simulink model "FeedBack_Linearization"  (R2021b)
settings: Solver=VariableStepAuto  StartTime=0.0  StopTime=10.0  RelTol=1e-3
undefined symbols (not defined in the file): Kd, Kp, q_dq_init
(part 2 of 9)

== matlab function FeedBack_Linearization/M ==
  data: q input; M output
function M = M_fun(q)
%M_fun
%    M = M_fun(Q1,Q2,Q3,Q4,Q5,Q6,Q7)

%    This function was generated by the Symbolic Math Toolbox version 9.0.
%    15-Apr-2022 02:51:43

q1 = q(1);
q2 = q(2);
q3 = q(3);
q4 = q(4);
q5 = q(5);
q6 = q(6);
q7 = q(7);

t2 = cos(q1);
t3 = cos(q2);
t4 = cos(q3);
t5 = cos(q4);
t6 = cos(q5);
t7 = cos(q6);
t8 = cos(q7);
t9 = sin(q1);
t10 = sin(q2);
t11 = sin(q3);
t12 = sin(q4);
t13 = sin(q5);
t14 = sin(q6);
t15 = sin(q7);
t16 = t2.^2;
t17 = t3.^2;
t18 = t9.^2;
t19 = t10.^2;
t20 = t11.^2;
t21 = t2.*t4;
t22 = t3.*t5;
t23 = t2.*t11;
t24 = t4.*t9;
t25 = t3.*t12;
t26 = t5.*t10;
t27 = t9.*t11;
t28 = t10.*t12;
t30 = t10.*t11.*t13;
t44 = t3.*t4.*t10;
t48 = t3.*t6.*t11;
t49 = t4.*t6.*t10;
t55 = t3.*t11.*t13;
t56 = t4.*t10.*t13;
t57 = t6.*t10.*t11;
t60 = t10.*(2.1e+1./5.0e+1);
t86 = t2.*t3.*(2.1e+1./5.0e+1);
t90 = t3.*t9.*(2.1e+1./5.0e+1);
t329 = t2.*3.55e-3;
t332 = t9.*3.55e-3;
t359 = t10.*t11.*2.25e-3;
t360 = t2.*t3.*1.6669e-1;
t361 = t2.*t10.*1.6669e-1;
t362 = t3.*t9.*1.6669e-1;
t364 = t9.*t10.*1.6669e-1;
t372 = t3.*t4.*2.25e-3;
t383 = t3.*t11.*3.492e-2;
t384 = t4.*t10.*3.492e-2;
t388 = t2.*t10.*7.669999999999999e-3;
t389 = t3.*t9.*7.669999999999999e-3;
t390 = t9.*t10.*7.669999999999999e-3;
t405 = t3.*t11.*3.818e-2;
t406 = t4.*t10.*3.818e-2;
t415 = t2.*t3.*7.669999999999999e-3;
t416 = t10.*3.9348e-1;
t471 = t2.*t3.*3.9348e-1;
t473 = t3.*t9.*3.9348e-1;
t493 = t9.*t10.*(-3.9348e-1);
t29 = t9.*t28;
t31 = t3.*t16;
t32 = t3.*t18;
t33 = t10.*t16;
t34 = t4.*t19;
t35 = t11.*t17;
t36 = t10.*t18;
t37 = t3.*t21;
t38 = t2.*t22;
t39 = t4.*t22;
t40 = t3.*t23;
t41 = t3.*t24;
t42 = t2.*t25;
t43 = t2.*t26;
t45 = t9.*t22;
t46 = t4.*t25;
t47 = t4.*t26;
t50 = t3.*t27;
t51 = t2.*t28;
t52 = t9.*t25;
t53 = t9.*t26;
t54 = t4.*t28;
t58 = t25.*(2.0./5.0);
t59 = t26.*(2.0./5.0);
t62 = t21.*t26;
t63 = t21.*t28;
t64 = t11.*t44;
t65 = t24.*t26;
t66 = t6.*t10.*t23;
t67 = t6.*t11.*t26;
t68 = t16.*t19;
t70 = t24.*t28;
t71 = t10.*t13.*t23;
t72 = t6.*t10.*t27;
t73 = t11.*t13.*t26;
t74 = t7.*t11.*t28;
t75 = t18.*t19;
t76 = t19.*t20;
t79 = t10.*t13.*t27;
t80 = t11.*t14.*t28;
t84 = -t55;
t85 = -t57;
t88 = t11.*t28.*(2.0./5.0);
t89 = t2.*t60;
t91 = t9.*t60;
t99 = -t86;
t101 = -t90;
t330 = t25.*1.8866e-1;
t331 = t26.*1.8866e-1;
t335 = -t332;
t355 = t11.*t28.*1.8866e-1;
t356 = t23.*2.25e-3;
t357 = t24.*2.25e-3;
t358 = t27.*2.25e-3;
t371 = t21.*2.25e-3;
t373 = t25.*5.267999999999999e-2;
t374 = t26.*5.267999999999999e-2;
t377 = t48.*2.37e-3;
t378 = t49.*2.37e-3;
t379 = t21.*3.492e-2;
t380 = t30.*2.37e-3;
t381 = t23.*3.492e-2;
t382 = t24.*3.492e-2;
t385 = t27.*3.492e-2;
t387 = -t372;
t391 = t48.*2.75e-2;
t392 = t49.*2.75e-2;
t393 = t30.*2.75e-2;
t402 = t21.*3.818e-2;
t403 = t23.*3.818e-2;
t404 = t24.*3.818e-2;
t408 = t27.*3.818e-2;
t418 = -t388;
t423 = -t390;
t428 = t11.*t28.*5.267999999999999e-2;
t435 = t22.*2.0e-4;
t440 = t28.*2.0e-4;
t441 = -t406;
t447 = t55.*5.000000000000001e-5;
t448 = t56.*5.000000000000001e-5;
t449 = t57.*5.000000000000001e-5;
t466 = t10.*t23.*(-3.492e-2);
t469 = t10.*t27.*(-3.492e-2);
t472 = t2.*t416;
t474 = t9.*t416;
t491 = t11.*t26.*2.0e-4;
t615 = t17.*1.16152294893368e-19;
t629 = t17.*8.909980864224564e-21;
t807 = t44.*7.000000000000001e-5;
t830 = t44.*4.999999999999997e-5;
t845 = t44.*2.23e-3;
t944 = t359+t384;
t1327 = t329+t364+t389;
t61 = -t58;
t69 = -t37;
t77 = -t46;
t78 = -t47;
t81 = -t50;
t82 = -t51;
t83 = -t53;
t87 = t29.*(2.0./5.0);
t92 = t38.*(2.0./5.0);
t93 = t43.*(2.0./5.0);
t94 = t45.*(2.0./5.0);
t95 = t46.*(2.0./5.0);
t96 = t47.*(2.0./5.0);
t97 = t51.*(2.0./5.0);
t98 = t53.*(2.0./5.0);
t100 = -t88;
t102 = t11.*t68;
t103 = -t62;
t104 = t11.*t75;
t105 = t12.*t76;
t106 = -t65;
t107 = -t66;
t108 = -t72;
t109 = -t73;
t110 = -t74;
t113 = t63.*(2.0./5.0);
t114 = t70.*(2.0./5.0);
t115 = t23+t41;
t116 = t24+t40;
t117 = t22+t54;
t118 = t28+t39;
t119 = t31+t32;
t120 = t33+t36;
t137 = t38+t63;
t138 = t45+t70;
t139 = t56+t67;
t223 = t17+t68+t75;
t334 = -t330;
t347 = t38.*1.8866e-1;
t348 = t43.*1.8866e-1;
t349 = t45.*1.8866e-1;
t350 = t46.*1.8866e-1;
t351 = t47.*1.8866e-1;
t352 = t51.*1.8866e-1;
t353 = t53.*1.8866e-1;
t354 = t29.*1.8866e-1;
t366 = -t355;
t375 = t63.*1.8866e-1;
t376 = t70.*1.8866e-1;
t386 = -t371;
t394 = -t374;
t400 = -t378;
t407 = t37.*2.25e-3;
t409 = -t385;
t410 = t40.*2.25e-3;
t411 = t10.*t371;
t412 = t41.*2.25e-3;
t413 = t50.*2.25e-3;
t414 = t10.*t357;
t417 = t38.*5.267999999999999e-2;
t419 = t43.*5.267999999999999e-2;
t420 = t45.*5.267999999999999e-2;
t421 = t46.*5.267999999999999e-2;
t422 = t47.*5.267999999999999e-2;
t424 = -t392;
t425 = t51.*5.267999999999999e-2;
t426 = t53.*5.267999999999999e-2;
t427 = t29.*5.267999999999999e-2;
t429 = t66.*2.37e-3;
t430 = t37.*3.492e-2;
t431 = t72.*2.37e-3;
t432 = t73.*2.37e-3;
t433 = t40.*3.492e-2;
t434 = t41.*3.492e-2;
t436 = t10.*t381;
t437 = t50.*3.492e-2;
t438 = -t402;
t439 = t10.*t385;
t443 = t72.*2.75e-2;
t444 = t73.*2.75e-2;
t458 = t37.*3.818e-2;
t460 = t40.*3.818e-2;
t461 = t41.*3.818e-2;
t464 = t10.*t403;
t465 = t50.*3.818e-2;
t468 = t10.*t408;
t475 = t66.*2.75e-2;
t476 = t70.*5.267999999999999e-2;
t478 = -t447;
t479 = t39.*2.0e-4;
t482 = t42.*2.0e-4;
t483 = t43.*2.0e-4;
t487 = t51.*2.0e-4;
t488 = t52.*2.0e-4;
t489 = t53.*2.0e-4;
t490 = t54.*2.0e-4;
t492 = t29.*2.0e-4;
t494 = t80.*4.9e-4;
t495 = t63.*5.267999999999999e-2;
t497 = t79.*5.000000000000001e-5;
t502 = t74.*2.019e-2;
t505 = t67.*5.000000000000001e-5;
t506 = t71.*5.000000000000001e-5;
t507 = t62.*2.0e-4;
t509 = t65.*2.0e-4;
t559 = t74.*1.9738e-1;
t647 = t31.*1.16152294893368e-19;
t652 = t32.*1.16152294893368e-19;
t662 = t33.*8.909980864224564e-21;
t663 = t36.*8.909980864224564e-21;
t666 = t68.*1.16152294893368e-19;
t667 = t75.*1.16152294893368e-19;
t681 = t68.*8.909980864224564e-21;
t684 = t75.*8.909980864224564e-21;
t805 = t34.*7.000000000000022e-5;
t811 = t35.*7.000000000000001e-5;
t829 = t64.*7.000000000000001e-5;
t831 = t76.*7.000000000000001e-5;
t832 = t64.*7.000000000000022e-5;
t833 = t76.*7.000000000000022e-5;
t834 = t34.*4.999999999999997e-5;
t835 = t35.*4.999999999999997e-5;
t839 = -t830;
t840 = t35.*2.23e-3;
t853 = t34.*2.19e-3;
t886 = t64.*7.299999999999999e-4;
t887 = t76.*7.299999999999999e-4;
t979 = t360+t418;
t980 = t362+t423;
t1340 = t335+t361+t415;
t1366 = t383+t387+t416;
t1410 = t428+t441+t491;
t111 = -t95;
t112 = -t97;
t121 = t21+t81;
t122 = t27+t69;
t123 = t25+t78;
t124 = t26+t77;
t125 = t116.^2;
t126 = t117.^2;
t127 = t5.*t115;
t128 = t6.*t115;
t129 = t6.*t116;
t130 = t6.*t118;
t131 = t7.*t117;
t132 = t12.*t115;
t133 = t13.*t115;
t134 = t13.*t116;
t135 = t13.*t118;
t136 = t14.*t117;
t145 = t2.*t10.*t115;
t146 = t3.*t9.*t115;
t148 = t7.*t12.*t116;
t150 = t8.*t13.*t117;
t151 = t9.*t10.*t115;
t152 = t9.*t10.*t116;
t153 = t12.*t14.*t116;
t154 = t13.*t15.*t117;
t169 = t42+t103;
t170 = t52+t106;
t171 = t49+t109;
t174 = t12.*t116.*(2.0./5.0);
t176 = t7.*t137;
t177 = t10.*t21.*t116;
t178 = t14.*t137;
t179 = t7.*t138;
t180 = t11.*t26.*t117;
t181 = t7.*t139;
t185 = t14.*t138;
t186 = t14.*t139;
t230 = t115.*t116;
t231 = t117.*t118;
t252 = t35+t102+t104;
t272 = t116.*t137;
t363 = -t350;
t365 = -t352;
t442 = -t407;
t445 = -t419;
t446 = -t422;
t450 = -t426;
t457 = -t429;
t459 = -t431;
t467 = -t437;
t477 = -t443;
t484 = -t458;
t496 = -t475;
t501 = -t482;
t503 = -t488;
t522 = t12.*t116.*1.8866e-1;
t542 = t13.*t117.*2.37e-3;
t556 = t13.*t117.*2.75e-2;
t571 = t12.*t116.*5.267999999999999e-2;
t578 = t6.*t117.*5.000000000000001e-5;
t588 = t5.*t116.*2.0e-4;
t837 = -t829;
t846 = -t834;
t847 = t102.*7.000000000000001e-5;
t849 = t104.*7.000000000000001e-5;
t859 = t102.*4.999999999999997e-5;
t860 = t104.*4.999999999999997e-5;
t867 = -t853;
t884 = t102.*2.23e-3;
t885 = t104.*2.23e-3;
t895 = -t886;
t907 = t105.*3.844e-2;
t915 = t105.*1.12e-3;
t916 = t105.*8.8e-4;
t1403 = t411+t466+t471;
t1404 = t414+t469+t473;
t1568 = t357+t409+t410+t430;
t1569 = t381+t386+t413+t434;
t1576 = t615+t666+t667;
t1594 = t629+t681+t684;
t1781 = t979.*t1327.*4.50275;
t1782 = t366+t400+t432+t448+t505;
t1785 = t980.*t1340.*4.50275;
t1789 = t944.*t1366.*2.4552;
t1797 = t60+t394+t405+t421+t440+t479;
t1801 = t647+t652+t662+t663;
t140 = t121.^2;
t141 = t12.*t125;
t142 = t13.*t126;
t143 = t5.*t129;
t144 = t6.*t131;
t147 = t5.*t134;
t149 = t6.*t136;
t155 = t5.*t122;
t156 = t6.*t121;
t157 = t6.*t122;
t158 = -t129;
t159 = t6.*t123;
t160 = t7.*t123;
t161 = t7.*t124;
t162 = t12.*t122;
t163 = t13.*t121;
t164 = t13.*t122;
t165 = t13.*t123;
t166 = t14.*t123;
t167 = t14.*t124;
t168 = -t136;
t172 = t127.*(2.0./5.0);
t173 = t132.*(2.0./5.0);
t182 = t2.*t3.*t122;
t187 = t2.*t10.*t121;
t188 = t2.*t10.*t122;
t190 = t3.*t11.*t123;
t191 = t4.*t10.*t123;
t192 = t7.*t12.*t121;
t194 = t9.*t10.*t122;
t195 = -t151;
t196 = t10.*t11.*t123;
t197 = t10.*t11.*t124;
t198 = t12.*t14.*t121;
t199 = -t153;
t200 = -t154;
t203 = -t174;
t206 = t12.*t121.*(2.0./5.0);
t208 = t6.*t169;
t209 = -t177;
t210 = t13.*t169;
t211 = t10.*t24.*t121;
t212 = t6.*t170;
t213 = -t180;
t214 = t8.*t171;
t217 = t13.*t170;
t218 = t15.*t171;
t224 = t29+t127;
t225 = t48+t135;
t226 = t83+t132;
t229 = t84+t130;
t240 = (t53-t132).^2;
t243 = -t7.*(t55-t130);
t244 = -t7.*(t53-t132);
t247 = -t14.*(t55-t130);
t249 = -t14.*(t53-t132);
t254 = t80+t181;
t260 = -t8.*t13.*(t53-t132);
t262 = t121.*t122;
t265 = -t13.*t15.*(t53-t132);
t276 = t110+t186;
t277 = t6.*t7.*(t53-t132);
t281 = t8.*t13.*(t53-t132);
t286 = t121.*t138;
t287 = t117.*t171;
t326 = -t116.*(t53-t132);
t342 = t116.*(t53-t132);
t367 = -t5.*t121.*(t53-t132);
t398 = -t170.*(t53-t132);
t520 = t127.*1.8866e-1;
t521 = t132.*1.8866e-1;
t525 = -t522;
t537 = t12.*t121.*1.8866e-1;
t539 = t128.*2.37e-3;
t540 = t129.*2.37e-3;
t541 = t134.*2.37e-3;
t543 = t135.*2.37e-3;
t553 = t128.*2.75e-2;
t554 = t129.*2.75e-2;
t555 = t134.*2.75e-2;
t557 = t135.*2.75e-2;
t566 = t131.*4.9e-4;
t569 = t127.*5.267999999999999e-2;
t570 = t132.*5.267999999999999e-2;
t574 = t136.*2.019e-2;
t577 = t129.*5.000000000000001e-5;
t579 = t130.*5.000000000000001e-5;
t583 = t133.*5.000000000000001e-5;
t584 = t134.*5.000000000000001e-5;
t587 = t127.*2.0e-4;
t589 = t132.*2.0e-4;
t593 = t153.*4.9e-4;
t602 = t12.*t121.*5.267999999999999e-2;
t604 = t148.*2.019e-2;
t623 = t5.*t121.*2.0e-4;
t627 = t154.*3.466000000000001e-2;
t628 = t178.*4.9e-4;
t630 = t181.*4.9e-4;
t631 = t185.*4.9e-4;
t636 = t179.*2.019e-2;
t637 = t150.*2.324e-2;
t640 = t186.*2.019e-2;
t657 = t176.*2.019e-2;
t664 = t136.*1.9738e-1;
t679 = t148.*1.9738e-1;
t700 = t176.*1.9738e-1;
t702 = t179.*1.9738e-1;
t704 = t186.*1.9738e-1;
t714 = t13.*(t53-t132).*(-2.37e-3);
t719 = t13.*(t53-t132).*(-2.75e-2);
t729 = t7.*(t55-t130).*(-4.9e-4);
t730 = t7.*(t53-t132).*(-4.9e-4);
t732 = t14.*(t53-t132).*(-4.9e-4);
t741 = t7.*(t53-t132).*4.9e-4;
t745 = t6.*(t53-t132).*(-5.000000000000001e-5);
t751 = t7.*(t53-t132).*(-2.019e-2);
t754 = t14.*(t55-t130).*(-2.019e-2);
t756 = t14.*(t53-t132).*(-2.019e-2);
t764 = t14.*(t55-t130).*2.019e-2;
t782 = t6.*t14.*(t53-t132).*2.019e-2;
t784 = t13.*t15.*(t53-t132).*(-3.466000000000001e-2);
t790 = t7.*(t53-t132).*(-1.9738e-1);
t793 = t14.*(t55-t130).*(-1.9738e-1);
t794 = t14.*(t53-t132).*(-1.9738e-1);
t804 = t7.*(t53-t132).*1.9738e-1;
t900 = t125.*7.000000000000001e-5;
t904 = t125.*7.000000000000022e-5;
t908 = t151.*7.000000000000001e-5;
t909 = t152.*7.000000000000001e-5;
t910 = t145.*7.000000000000022e-5;
t911 = t146.*7.000000000000022e-5;
M = ft_1({q1,q2,t10,t100,t101,t105,t107,t108,t11,t111,t112,t113,t114,t115,t116,t117,t119,t12,t120,t121,t122,t123,t124,t125,t126,t128,t129,t13,t130,t131,t132,t1327,t133,t134,t1340,t136,t1366,t137,t138,t139,t14,t140,t1403,t1404,t141,t1410,t142,t143,t144,t145,t146,t147,t148,t149,t15,t150,t151,t152,t153,t154,t155,t156,t1568,t1569,t157,t1576,t158,t159,t1594,t16,t160,t161,t162,t163,t164,t165,t166,t167,t168,t169,t17,t170,t171,t172,t173,t174,t176,t177,t178,t1781,t1782,t1785,t1789,t179,t1797,t18,t180,t1801,t182,t185,t186,t187,t188,t190,t191,t192,t194,t195,t196,t197,t198,t199,t200,t203,t206,t208,t209,t210,t211,t212,t213,t214,t217,t218,t223,t224,t225,t23,t230,t231,t240,t243,t244,t247,t249,t252,t254,t262,t265,t27,t272,t277,t28,t281,t286,t287,t30,t31,t32,t33,t331,t334,t34,t342,t347,t348,t349,t351,t353,t354,t356,t358,t36,t363,t365,t367,t373,t375,t376,t377,t379,t380,t382,t391,t393,t398,t403,t404,t408,t412,t417,t420,t424,t425,t427,t43,t433,t435,t438,t44,t442,t444,t445,t446,t449,t450,t457,t459,t460,t461,t464,t465,t467,t468,t472,t476,t477,t478,t483,t484,t487,t489,t490,t492,t493,t494,t495,t496,t497,t5,t501,t502,t503,t506,t507,t509,t51,t520,t521,t525,t53,t537,t539,t540,t541,t542,t543,t55,t553,t554,t555,t556,t557,t559,t566,t569,t57,t570,t571,t574,t577,t578,t579,t583,t584,t587,t588,t589,t59,t593,t6,t60,t602,t604,t61,t623,t627,t628,t630,t631,t636,t637,t64,t640,t657,t66,t664,t679,t68,t7,t700,t702,t704,t71,t714,t719,t72,t729,t732,t74,t741,t745,t75,t751,t756,t76,t764,t782,t784,t79,t793,t794,t8,t804,t805,t807,t811,t82,t831,t832,t833,t835,t837,t839,t840,t845,t846,t847,t849,t85,t859,t86,t860,t867,t87,t88,t884,t885,t887,t89,t895,t9,t90,t900,t904,t907,t908,t909,t91,t910,t911,t915,t916,t92,t93,t94,t944,t96,t97,t979,t98,t980,t99});
end
function M = ft_1(ct)
q1 = ct{1};
q2 = ct{2};
t10 = ct{3};
t100 = ct{4};
t101 = ct{5};
t105 = ct{6};
t107 = ct{7};
t108 = ct{8};
t11 = ct{9};
t111 = ct{10};
t112 = ct{11};
t113 = ct{12};
t114 = ct{13};
t115 = ct{14};
t116 = ct{15};
t117 = ct{16};
t119 = ct{17};
t12 = ct{18};
t120 = ct{19};
t121 = ct{20};
t122 = ct{21};
t123 = ct{22};
t124 = ct{23};
t125 = ct{24};
t126 = ct{25};
t128 = ct{26};
t129 = ct{27};
t13 = ct{28};
t130 = ct{29};
t131 = ct{30};
t132 = ct{31};
t1327 = ct{32};
t133 = ct{33};
t134 = ct{34};
t1340 = ct{35};
t136 = ct{36};
t1366 = ct{37};
t137 = ct{38};
t138 = ct{39};
t139 = ct{40};
t14 = ct{41};
t140 = ct{42};
t1403 = ct{43};
t1404 = ct{44};
t141 = ct{45};
t1410 = ct{46};
t142 = ct{47};
t143 = ct{48};
t144 = ct{49};
t145 = ct{50};
t146 = ct{51};
t147 = ct{52};
t148 = ct{53};
t149 = ct{54};
t15 = ct{55};
t150 = ct{56};
t151 = ct{57};
t152 = ct{58};
t153 = ct{59};
t154 = ct{60};
t155 = ct{61};
t156 = ct{62};
t1568 = ct{63};
t1569 = ct{64};
t157 = ct{65};
t1576 = ct{66};
t158 = ct{67};
t159 = ct{68};
t1594 = ct{69};
t16 = ct{70};
t160 = ct{71};
t161 = ct{72};
t162 = ct{73};
t163 = ct{74};
t164 = ct{75};
t165 = ct{76};
t166 = ct{77};
t167 = ct{78};
t168 = ct{79};
t169 = ct{80};
t17 = ct{81};
t170 = ct{82};
t171 = ct{83};
t172 = ct{84};
t173 = ct{85};
t174 = ct{86};
t176 = ct{87};
t177 = ct{88};
t178 = ct{89};
t1781 = ct{90};
t1782 = ct{91};
t1785 = ct{92};
t1789 = ct{93};
t179 = ct{94};
t1797 = ct{95};
t18 = ct{96};
t180 = ct{97};
t1801 = ct{98};
t182 = ct{99};
t185 = ct{100};
t186 = ct{101};
t187 = ct{102};
t188 = ct{103};
t190 = ct{104};
t191 = ct{105};
t192 = ct{106};
t194 = ct{107};
t195 = ct{108};
t196 = ct{109};
t197 = ct{110};
t198 = ct{111};
t199 = ct{112};
t200 = ct{113};
t203 = ct{114};
t206 = ct{115};
t208 = ct{116};
t209 = ct{117};
t210 = ct{118};
t211 = ct{119};
t212 = ct{120};
t213 = ct{121};
t214 = ct{122};
t217 = ct{123};
t218 = ct{124};
t223 = ct{125};
t224 = ct{126};
t225 = ct{127};
t23 = ct{128};
t230 = ct{129};
t231 = ct{130};
t240 = ct{131};
t243 = ct{132};
t244 = ct{133};
t247 = ct{134};
t249 = ct{135};
t252 = ct{136};
t254 = ct{137};
t262 = ct{138};
t265 = ct{139};
t27 = ct{140};
t272 = ct{141};
t277 = ct{142};
t28 = ct{143};
t281 = ct{144};
t286 = ct{145};
t287 = ct{146};
t30 = ct{147};
t31 = ct{148};
t32 = ct{149};
t33 = ct{150};
t331 = ct{151};
t334 = ct{152};
t34 = ct{153};
t342 = ct{154};
t347 = ct{155};
t348 = ct{156};
t349 = ct{157};
t351 = ct{158};
t353 = ct{159};
t354 = ct{160};
t356 = ct{161};
t358 = ct{162};
t36 = ct{163};
t363 = ct{164};
t365 = ct{165};
t367 = ct{166};
t373 = ct{167};
t375 = ct{168};
t376 = ct{169};
t377 = ct{170};
t379 = ct{171};
t380 = ct{172};
t382 = ct{173};
t391 = ct{174};
t393 = ct{175};
t398 = ct{176};
t403 = ct{177};
t404 = ct{178};
t408 = ct{179};
t412 = ct{180};
t417 = ct{181};
t420 = ct{182};
t424 = ct{183};
t425 = ct{184};
t427 = ct{185};
t43 = ct{186};
t433 = ct{187};
t435 = ct{188};
t438 = ct{189};
t44 = ct{190};
t442 = ct{191};
t444 = ct{192};
t445 = ct{193};
t446 = ct{194};
t449 = ct{195};
t450 = ct{196};
t457 = ct{197};
t459 = ct{198};
t460 = ct{199};
t461 = ct{200};
t464 = ct{201};
t465 = ct{202};
t467 = ct{203};
t468 = ct{204};
t472 = ct{205};
t476 = ct{206};
t477 = ct{207};
t478 = ct{208};
t483 = ct{209};
t484 = ct{210};
t487 = ct{211};
t489 = ct{212};
t490 = ct{213};
t492 = ct{214};
t493 = ct{215};
t494 = ct{216};
t495 = ct{217};
t496 = ct{218};
t497 = ct{219};
t5 = ct{220};
t501 = ct{221};
t502 = ct{222};
t503 = ct{223};
t506 = ct{224};
t507 = ct{225};
t509 = ct{226};
t51 = ct{227};
t520 = ct{228};
t521 = ct{229};
t525 = ct{230};
t53 = ct{231};
t537 = ct{232};
t539 = ct{233};
t540 = ct{234};
t541 = ct{235};
t542 = ct{236};
t543 = ct{237};
t55 = ct{238};
t553 = ct{239};
t554 = ct{240};
t555 = ct{241};
t556 = ct{242};
t557 = ct{243};
t559 = ct{244};
t566 = ct{245};
t569 = ct{246};
t57 = ct{247};
t570 = ct{248};
t571 = ct{249};
t574 = ct{250};
t577 = ct{251};
t578 = ct{252};
t579 = ct{253};
t583 = ct{254};
t584 = ct{255};
t587 = ct{256};
t588 = ct{257};
t589 = ct{258};
t59 = ct{259};
t593 = ct{260};
t6 = ct{261};
t60 = ct{262};
t602 = ct{263};
t604 = ct{264};
t61 = ct{265};
t623 = ct{266};
t627 = ct{267};
t628 = ct{268};
t630 = ct{269};
t631 = ct{270};
t636 = ct{271};
t637 = ct{272};
t64 = ct{273};
t640 = ct{274};
t657 = ct{275};
t66 = ct{276};
t664 = ct{277};
t679 = ct{278};
t68 = ct{279};
t7 = ct{280};
t700 = ct{281};
t702 = ct{282};
t704 = ct{283};
t71 = ct{284};
t714 = ct{285};
t719 = ct{286};
t72 = ct{287};
t729 = ct{288};
t732 = ct{289};
t74 = ct{290};
t741 = ct{291};
t745 = ct{292};
t75 = ct{293};
t751 = ct{294};
t756 = ct{295};
t76 = ct{296};
t764 = ct{297};
t782 = ct{298};
t784 = ct{299};
t79 = ct{300};
t793 = ct{301};
t794 = ct{302};
t8 = ct{303};
t804 = ct{304};
t805 = ct{305};
t807 = ct{306};
t811 = ct{307};
t82 = ct{308};
t831 = ct{309};
t832 = ct{310};
t833 = ct{311};
t835 = ct{312};
t837 = ct{313};
t839 = ct{314};
t840 = ct{315};
t845 = ct{316};
t846 = ct{317};
t847 = ct{318};
t849 = ct{319};
t85 = ct{320};
t859 = ct{321};
t86 = ct{322};
t860 = ct{323};
t867 = ct{324};
t87 = ct{325};
t88 = ct{326};
t884 = ct{327};
t885 = ct{328};
t887 = ct{329};
t89 = ct{330};
t895 = ct{331};
t9 = ct{332};
t90 = ct{333};
t900 = ct{334};
t904 = ct{335};
t907 = ct{336};
t908 = ct{337};
t909 = ct{338};
t91 = ct{339};
t910 = ct{340};
t911 = ct{341};
t915 = ct{342};
t916 = ct{343};
t92 = ct{344};
t93 = ct{345};
t94 = ct{346};
t944 = ct{347};
t96 = ct{348};
t97 = ct{349};
t979 = ct{350};
t98 = ct{351};
t980 = ct{352};
t99 = ct{353};
t921 = t126.*1.11e-3;
t927 = t177.*7.000000000000022e-5;
t932 = t177.*7.000000000000001e-5;
t934 = t145.*4.999999999999997e-5;
t935 = t146.*4.999999999999997e-5;
t936 = t151.*4.999999999999997e-5;
t937 = t152.*4.999999999999997e-5;
t940 = t125.*7.299999999999999e-4;
t946 = t151.*2.23e-3;
t947 = t152.*2.23e-3;
t967 = t126.*1.12e-3;
t974 = t180.*1.11e-3;
t975 = t145.*2.19e-3;
t976 = t146.*2.19e-3;
t1004 = t177.*7.299999999999999e-4;
t1021 = t230.*7.000000000000022e-5;
t1030 = t180.*1.12e-3;
t1036 = t230.*7.000000000000001e-5;
t1063 = t126.*4.988e-2;
t1066 = t231.*1.11e-3;
t1079 = t230.*7.299999999999999e-4;
t1086 = t180.*4.988e-2;
t1094 = t231.*1.12e-3;
t1124 = t272.*3.844e-2;
t1125 = t272.*8.8e-4;
t1136 = t272.*1.12e-3;
t1155 = t231.*4.988e-2;
t1209 = t5.*t121.*(t53-t132).*(-1.11e-3);
t1233 = t170.*(t53-t132).*(-1.11e-3);
t1249 = t5.*t121.*(t53-t132).*(-1.12e-3);
t1259 = t170.*(t53-t132).*(-1.12e-3);
t1285 = t5.*t121.*(t53-t132).*(-4.988e-2);
t1303 = t170.*(t53-t132).*(-4.988e-2);
t1601 = t373+t435+t446+t490;
t1625 = t334+t351+t542+t578;
t1671 = (t119.*t1576)./2.0;
t1687 = (t120.*t1594)./2.0;
t1699 = t408+t484+t571+t588;
t1771 = t358+t382+t433+t442+t472;
t1777 = t356+t379+t412+t467+t493;
t1784 = -t1781;
t1808 = t101+t420+t468+t476+t503+t509;
t1810 = t99+t417+t464+t495+t501+t507;
t1867 = (t223.*t1801)./2.0;
t1969 = t1403.*t1568.*2.4552;
t1970 = t1404.*t1569.*2.4552;
t1995 = t1410.*t1797.*2.61155;
t175 = t12.*t140;
t183 = t5.*t156;
t184 = -t143;
t189 = t5.*t163;
t193 = -t149;
t201 = -t156;
t202 = -t173;
t204 = -t167;
t205 = t155.*(2.0./5.0);
t207 = t162.*(2.0./5.0);
t215 = -t182;
t219 = -t191;
t220 = -t198;
t222 = -t206;
t227 = t30+t159;
t228 = t43+t162;
t232 = t8.*t225;
t233 = t6.*t224;
t234 = t7.*t224;
t235 = t15.*t225;
t236 = t13.*t224;
t237 = t14.*t224;
t238 = t85+t165;
t241 = t82+t155;
t253 = (t57-t165).^2;
t255 = t6.*t244;
t258 = t10.*t27.*t224;
t259 = t6.*t249;
t263 = -t6.*(t51-t155);
t264 = -t7.*(t51-t155);
t266 = -t13.*(t51-t155);
t267 = -t14.*(t51-t155);
t268 = -t8.*(t57-t165);
t269 = -t15.*(t57-t165);
t271 = t13.*t240;
t274 = t71+t208;
t275 = t79+t212;
t283 = -t262;
t285 = t8.*t254;
t288 = t15.*t254;
t290 = t107+t210;
t291 = t108+t217;
t292 = t7.*t15.*(t57-t165);
t296 = -t286;
t297 = -t10.*t23.*(t51-t155);
t301 = t147+t157;
t302 = t144+t166;
t304 = -t8.*(t66-t210);
t305 = -t15.*(t66-t210);
t307 = -t8.*(t72-t217);
t308 = t10.*t23.*(t51-t155);
t309 = -t15.*(t72-t217);
t310 = t117.*t225;
t311 = t115.*t224;
t312 = t116.*t224;
t313 = t145+t194;
t314 = t152+t187;
t318 = t8.*(t66-t210);
t325 = t121.*t224;
t337 = -t7.*(t143-t164);
t338 = -t116.*(t51-t155);
t341 = -t14.*(t143-t164);
t346 = t76+t125+t140;
t368 = -t6.*t117.*(t57-t165);
t369 = -t121.*(t51-t155);
t370 = -t122.*(t51-t155);
t399 = -t139.*(t57-t165);
t401 = t6.*t117.*(t57-t165);
t452 = t161+t247;
t455 = t44+t188+t195;
t462 = t139.*(t57-t165);
t523 = (t129+t13.*(t51-t155)).^2;
t524 = -t521;
t528 = -t8.*(t129+t13.*(t51-t155));
t529 = -t8.*(t167+t7.*(t55-t130));
t531 = -t15.*(t129+t13.*(t51-t155));
t532 = -t15.*(t167+t7.*(t55-t130));
t536 = t155.*1.8866e-1;
t538 = t162.*1.8866e-1;
t544 = t64+t209+t211;
t545 = -t537;
t548 = (t53-t132).*(t51-t155);
t550 = (t55-t130).*(t57-t165);
t551 = t8.*(t167+t7.*(t55-t130));
t552 = t15.*(t129+t13.*(t51-t155));
t560 = t147.*2.37e-3;
t561 = t156.*2.37e-3;
t562 = t157.*2.37e-3;
t563 = t159.*2.37e-3;
t564 = t163.*2.37e-3;
t576 = t147.*2.75e-2;
t580 = t156.*2.75e-2;
t581 = t157.*2.75e-2;
t582 = t159.*2.75e-2;
t585 = t163.*2.75e-2;
t590 = -t574;
t592 = t144.*4.9e-4;
t594 = t166.*4.9e-4;
t595 = t167.*4.9e-4;
t598 = t155.*5.267999999999999e-2;
t600 = -t583;
t601 = -t584;
t603 = t162.*5.267999999999999e-2;
t605 = t149.*2.019e-2;
t606 = -t589;
t607 = t160.*2.019e-2;
t608 = t161.*2.019e-2;
t609 = t143.*5.000000000000001e-5;
t613 = t156.*5.000000000000001e-5;
t617 = t163.*5.000000000000001e-5;
t618 = t164.*5.000000000000001e-5;
t619 = t165.*5.000000000000001e-5;
t621 = t217.*2.37e-3;
t624 = t155.*2.0e-4;
t625 = t162.*2.0e-4;
t632 = t198.*4.9e-4;
t635 = t210.*2.37e-3;
t638 = (t53-t132).*(t72-t217);
t639 = (t57-t165).*(t74-t186);
t641 = t192.*2.019e-2;
t643 = -t628;
t644 = -t631;
t645 = t210.*2.75e-2;
t651 = t217.*2.75e-2;
t660 = -t636;
t661 = -t640;
t665 = -t657;
t669 = t208.*5.000000000000001e-5;
t670 = t212.*5.000000000000001e-5;
t674 = -t664;
t678 = t218.*3.466000000000001e-2;
t680 = t149.*1.9738e-1;
t682 = t160.*1.9738e-1;
t683 = t161.*1.9738e-1;
t699 = t214.*2.324e-2;
t705 = t192.*1.9738e-1;
t707 = -t8.*(t153+t7.*(t143-t164));
t709 = -t15.*(t153+t7.*(t143-t164));
t712 = -t704;
t725 = t15.*(t153+t7.*(t143-t164));
t726 = (t57-t165).*(t149-t160);
t736 = t6.*(t51-t155).*(-2.37e-3);
t738 = t13.*(t51-t155).*(-2.37e-3);
t744 = t6.*(t51-t155).*(-2.75e-2);
t746 = t13.*(t51-t155).*(-2.75e-2);
t755 = t13.*(t51-t155).*2.37e-3;
t758 = t277.*(-4.9e-4);
t759 = t14.*(t51-t155).*(-4.9e-4);
t760 = t7.*(t57-t165).*(-4.9e-4);
t761 = t13.*(t51-t155).*2.75e-2;
t766 = t7.*(t57-t165).*4.9e-4;
t767 = t6.*(t51-t155).*(-5.000000000000001e-5);
t768 = t13.*(t51-t155).*(-5.000000000000001e-5);
t770 = t6.*t756;
t772 = t7.*(t51-t155).*(-2.019e-2);
t774 = t14.*(t57-t165).*(-2.019e-2);
t776 = t6.*(t51-t155).*5.000000000000001e-5;
t778 = t13.*(t51-t155).*5.000000000000001e-5;
t785 = t8.*(t57-t165).*(-3.466000000000001e-2);
t787 = t281.*(-2.324e-2);
t788 = t15.*(t57-t165).*(-2.324e-2);
t802 = t15.*(t57-t165).*2.324e-2;
t813 = t6.*t794;
t814 = t7.*(t51-t155).*(-1.9738e-1);
t816 = t14.*(t57-t165).*(-1.9738e-1);
t822 = (t129+t13.*(t51-t155)).*(t53-t132);
t828 = t14.*(t57-t165).*1.9738e-1;
t842 = t15.*(t66-t210).*(-3.466000000000001e-2);
t844 = t15.*(t72-t217).*(-3.466000000000001e-2);
t850 = t8.*(t72-t217).*(-2.324e-2);
t869 = t7.*(t143-t164).*(-4.9e-4);
t877 = t14.*(t143-t164).*(-2.019e-2);
t883 = t7.*(t143-t164).*4.9e-4;
t912 = t142.*9.999999999999998e-6;
t913 = t140.*7.000000000000001e-5;
t917 = t140.*7.000000000000022e-5;
t918 = -t908;
t919 = -t909;
t924 = t14.*(t143-t164).*(-1.9738e-1);
t925 = t187.*7.000000000000001e-5;
t926 = t188.*7.000000000000001e-5;
t928 = t182.*7.000000000000022e-5;
t929 = t194.*7.000000000000022e-5;
t939 = (t129+t13.*(t51-t155)).*(t143-t164);
t943 = -t927;
t948 = -t935;
t951 = t211.*7.000000000000022e-5;
t956 = -t946;
t957 = t182.*4.999999999999997e-5;
t958 = t211.*7.000000000000001e-5;
t959 = t187.*4.999999999999997e-5;
t960 = t188.*4.999999999999997e-5;
t961 = t194.*4.999999999999997e-5;
t965 = t140.*7.299999999999999e-4;
t969 = t142.*2.769999999999999e-3;
t971 = t187.*2.23e-3;
t972 = t188.*2.23e-3;
t977 = t190.*1.11e-3;
t978 = t191.*1.11e-3;
t981 = t142.*1.0e-5;
t985 = t141.*3.844e-2;
t991 = t7.*(t129+t13.*(t51-t155)).*(-4.9e-4);
t994 = -t974;
t995 = -t976;
t1000 = t141.*1.12e-3;
t1002 = t14.*(t129+t13.*(t51-t155)).*(-2.019e-2);
t1003 = t141.*8.8e-4;
t1005 = t7.*(t129+t13.*(t51-t155)).*4.9e-4;
t1007 = t182.*2.19e-3;
t1008 = t194.*2.19e-3;
t1012 = t8.*(t129+t13.*(t51-t155)).*(-3.466000000000001e-2);
t1019 = t196.*3.844e-2;
t1020 = t197.*3.844e-2;
t1023 = t15.*(t167+t7.*(t55-t130)).*(-2.324e-2);
t1028 = t211.*7.299999999999999e-4;
t1032 = t196.*1.12e-3;
t1033 = t197.*1.12e-3;
t1034 = t190.*8.8e-4;
t1035 = t191.*8.8e-4;
t1038 = t196.*8.8e-4;
t1039 = t197.*8.8e-4;
t1041 = t8.*(t129+t13.*(t51-t155)).*(-2.324e-2);
t1045 = -t1030;
t1052 = -t1036;
t1058 = t8.*(t129+t13.*(t51-t155)).*2.324e-2;
t1067 = t14.*(t129+t13.*(t51-t155)).*(-1.9738e-1);
t1071 = t262.*7.000000000000022e-5;
t1076 = t14.*(t129+t13.*(t51-t155)).*1.9738e-1;
t1077 = t262.*7.000000000000001e-5;
t1080 = t190.*1.144e-2;
t1081 = t191.*1.144e-2;
t1085 = t240.*1.11e-3;
t1090 = t287.*9.999999999999998e-6;
t1092 = -t1086;
t1104 = t262.*7.299999999999999e-4;
t1115 = t240.*1.12e-3;
t1130 = t287.*2.769999999999999e-3;
t1135 = t287.*1.0e-5;
t1140 = t286.*3.844e-2;
t1146 = t8.*(t153+t7.*(t143-t164)).*(-3.466000000000001e-2);
t1151 = t286.*8.8e-4;
t1154 = t8.*(t153+t7.*(t143-t164)).*3.466000000000001e-2;
t1159 = t286.*1.12e-3;
t1173 = t240.*4.988e-2;
t1200 = t342.*(-3.844e-2);
t1211 = t342.*(-1.12e-3);
t1213 = t121.*(t51-t155).*(-1.11e-3);
t1214 = t122.*(t51-t155).*(-1.11e-3);
t1217 = t342.*(-8.8e-4);
t1221 = t116.*(t51-t155).*(-3.844e-2);
t1223 = t121.*(t51-t155).*1.11e-3;
t1231 = t116.*(t51-t155).*(-1.12e-3);
t1234 = t116.*(t51-t155).*3.844e-2;
t1236 = t116.*(t51-t155).*(-8.8e-4);
t1242 = t116.*(t51-t155).*1.12e-3;
t1246 = t116.*(t51-t155).*8.8e-4;
t1250 = t121.*(t51-t155).*(-8.8e-4);
t1251 = t122.*(t51-t155).*(-8.8e-4);
t1252 = t121.*(t51-t155).*8.8e-4;
t1273 = t121.*(t51-t155).*(-1.144e-2);
t1274 = t122.*(t51-t155).*(-1.144e-2);
t1286 = t121.*(t51-t155).*1.144e-2;
t1715 = t403+t461+t602+t623;
t1776 = t354+t520+t714+t745;
t1919 = t60+t331+t363+t377+t478+t543+t579;
t1949 = t91+t438+t450+t465+t492+t570+t587;
t1972 = t1410.*t1601.*2.61155;
t1991 = t1404.*t1771.*2.4552;
t1992 = t1403.*t1777.*2.4552;
t1996 = -t1995;
t2004 = t1569.*t1771.*2.4552;
t2005 = t1568.*t1777.*2.4552;
t2013 = t1625.*t1782.*(3.41e+2./1.0e+2);
t2015 = t1601.*t1797.*2.61155;
t2021 = t1699.*t1810.*2.61155;
t216 = -t183;
t221 = -t205;
t239 = t228.^2;
t242 = t7.*t228;
t245 = t14.*t228;
t246 = t7.*t227;
t248 = t8.*t227;
t250 = t14.*t227;
t251 = t15.*t227;
t257 = t8.*t13.*t228;
t261 = t13.*t15.*t228;
t279 = t7.*t268;
t280 = t11.*t28.*t227;
t282 = t7.*t269;
t284 = t14.*t253;
t293 = t7.*t274;
t294 = t14.*t274;
t295 = t7.*t275;
t298 = t14.*t275;
t299 = -t288;
t300 = t128+t189;
t316 = t164+t184;
t317 = t160+t193;
t320 = t8.*t301;
t321 = t8.*t302;
t323 = t15.*t301;
t324 = t15.*t302;
t327 = -t312;
t328 = t117.*t227;
t333 = t5.*t116.*t228;
t339 = t121.*t228;
t343 = t123.*t227;
t344 = t124.*t227;
t395 = t163+t233;
t397 = t169.*t228;
t451 = t134+t263;
t453 = t201+t236;
t470 = t34+t146+t215;
t498 = t158+t266;
t499 = t204+t243;
t500 = t105+t141+t175;
t504 = (t156-t236).^2;
t508 = t224.*t228;
t513 = -t8.*(t156-t236);
t517 = -t15.*(t156-t236);
t534 = t15.*(t156-t236);
t546 = t7.*t528;
t547 = t7.*t531;
t558 = t14.*t523;
t568 = t218+t285;
t572 = -t561;
t573 = t7.*t552;
t575 = -t548;
t586 = t189.*2.37e-3;
t599 = -t580;
t611 = t189.*2.75e-2;
t612 = -t595;
t614 = t234+t259;
t616 = -t598;
t620 = -t603;
t622 = -t605;
t626 = -t608;
t633 = -t618;
t634 = -t619;
t642 = -t624;
t646 = t183.*5.000000000000001e-5;
t648 = t148+t341;
t654 = t230+t283;
t655 = t237+t277;
t656 = -t228.*(t66-t210);
t668 = -t639;
t672 = t199+t337;
t676 = t228.*(t66-t210);
t685 = t228.*t301;
t695 = -t682;
t697 = t233.*2.37e-3;
t698 = t236.*2.37e-3;
t701 = t233.*2.75e-2;
t703 = t236.*2.75e-2;
t711 = t237.*4.9e-4;
t713 = t13.*t228.*2.37e-3;
t716 = t233.*5.000000000000001e-5;
t717 = t13.*t228.*2.75e-2;
t718 = t236.*5.000000000000001e-5;
t727 = t234.*2.019e-2;
t739 = t235.*3.466000000000001e-2;
t743 = t6.*t228.*5.000000000000001e-5;
t747 = t232.*2.324e-2;
t777 = t234.*1.9738e-1;
t797 = -t228.*(t156-t236);
t799 = t285.*3.466000000000001e-2;
t801 = t7.*t785;
t808 = t288.*2.324e-2;
t810 = t292.*(-2.324e-2);
t818 = t6.*(t53-t132).*(t156-t236);
t824 = -t452.*(t57-t165);
t827 = t292.*2.324e-2;
t838 = -t6.*t228.*(t129+t13.*(t51-t155));
t843 = -t822;
t848 = t318.*(-2.324e-2);
t852 = -t275.*(t156-t236);
t857 = t232+t532;
t866 = t253.*4.466636216449161e-20;
t870 = -t274.*(t129+t13.*(t51-t155));
t875 = t275.*(t156-t236);
t889 = t235+t551;
t914 = t197+t272+t296;
t933 = t190+t258+t308;
t938 = -t925;
t945 = -t928;
t954 = t7.*(t156-t236).*(-4.9e-4);
t968 = t14.*(t156-t236).*(-2.019e-2);
t973 = t7.*(t156-t236).*4.9e-4;
t982 = -t958;
t983 = -t960;
t986 = t8.*(t156-t236).*(-3.466000000000001e-2);
t990 = -t969;
t996 = -t977;
t997 = -t978;
t998 = t8.*(t156-t236).*(-2.324e-2);
t1013 = t551.*(-3.466000000000001e-2);
t1014 = t175.*3.844e-2;
t1015 = t552.*(-3.466000000000001e-2);
t1016 = t401.*(-4.466636216449161e-20);
t1022 = t552.*(-2.324e-2);
t1024 = t175.*1.12e-3;
t1025 = t551.*3.466000000000001e-2;
t1026 = t552.*3.466000000000001e-2;
t1027 = t175.*8.8e-4;
t1029 = t401.*4.466636216449161e-20;
t1037 = -t1019;
t1042 = t552.*2.324e-2;
t1043 = t462.*(-4.466636216449161e-20);
t1044 = -t1028;
t1048 = t14.*(t156-t236).*(-1.9738e-1);
t1049 = -t1032;
t1050 = -t1034;
t1051 = -t1035;
t1053 = -t1038;
t1059 = t7.*t1012;
t1062 = t14.*(t156-t236).*1.9738e-1;
t1073 = t271.*9.999999999999998e-6;
t1074 = t253.*9.999999999999998e-6;
t1078 = -t1071;
t1087 = -t1080;
t1088 = -t1081;
t1095 = t258.*1.11e-3;
t1097 = t196+t325+t338;
t1103 = t523.*4.466636216449161e-20;
t1109 = t219+t311+t370;
t1111 = t271.*1.0e-5;
t1117 = t271.*2.769999999999999e-3;
t1118 = t550.*4.466636216449161e-20;
t1119 = -t1104;
t1128 = t308.*(-1.11e-3);
t1129 = t310.*9.999999999999998e-6;
t1131 = t258.*8.8e-4;
t1150 = -t1140;
t1153 = t725.*(-2.324e-2);
t1160 = -t1151;
t1163 = t253.*1.2e-4;
t1166 = -t1159;
t1167 = t311.*1.11e-3;
t1168 = t312.*1.11e-3;
t1169 = t308.*(-8.8e-4);
t1176 = t310.*2.769999999999999e-3;
t1181 = t310.*1.0e-5;
t1182 = t258.*1.144e-2;
t1183 = t401.*(-9.999999999999998e-6);
t1186 = t401.*9.999999999999998e-6;
t1193 = t311.*8.8e-4;
t1194 = t312.*8.8e-4;
t1199 = t325.*3.844e-2;
t1201 = t462.*(-9.999999999999998e-6);
t1208 = t308.*(-1.144e-2);
t1210 = t325.*1.12e-3;
t1216 = t325.*8.8e-4;
t1218 = t462.*9.999999999999998e-6;
M = ft_2({q1,q2,t10,t100,t1000,t1002,t1003,t1004,t1005,t1007,t1008,t1012,t1014,t1020,t1021,t1023,t1024,t1025,t1026,t1027,t1029,t1033,t1034,t1037,t1039,t1042,t1043,t1044,t1045,t1049,t1050,t1051,t1052,t1053,t1058,t1059,t1062,t1063,t1066,t1073,t1074,t1076,t1077,t1078,t1079,t1080,t1085,t1087,t1088,t1090,t1092,t1094,t1095,t1097,t1103,t111,t1111,t1115,t1117,t1118,t1119,t112,t1124,t1125,t1128,t1129,t113,t1130,t1131,t1135,t1136,t114,t1140,t1146,t1150,t1151,t1153,t1154,t1155,t1159,t116,t1160,t1163,t1166,t1167,t1168,t1169,t117,t1173,t1176,t1181,t1182,t1183,t1186,t119,t1193,t1194,t1199,t12,t120,t1200,t1208,t1209,t121,t1210,t1211,t1213,t1214,t1216,t1217,t1218,t122,t1223,t1233,t1234,t1242,t1246,t1249,t1250,t1251,t1252,t1259,t126,t1274,t1285,t1286,t129,t13,t130,t1303,t131,t132,t1327,t133,t1340,t136,t1366,t137,t138,t14,t1403,t1404,t1410,t142,t143,t149,t15,t150,t153,t154,t155,t156,t1568,t1569,t16,t160,t1601,t1625,t164,t165,t167,t1671,t168,t1687,t1699,t17,t170,t171,t1715,t172,t173,t174,t176,t1771,t1776,t1777,t178,t1782,t1784,t1785,t1789,t179,t1797,t18,t180,t1808,t1810,t185,t186,t1867,t191,t1919,t192,t1949,t1969,t1970,t1972,t198,t1991,t1992,t1996,t200,t2004,t2005,t2013,t2015,t202,t2021,t203,t205,t206,t207,t210,t213,t214,t216,t217,t220,t221,t222,t223,t224,t225,t227,t228,t231,t236,t239,t240,t242,t244,t245,t246,t248,t249,t250,t251,t252,t253,t254,t257,t261,t264,t265,t267,t268,t269,t271,t274,t277,t279,t280,t281,t284,t287,t292,t293,t294,t295,t298,t299,t300,t301,t302,t305,t307,t308,t309,t31,t310,t311,t312,t313,t314,t318,t32,t320,t321,t323,t324,t327,t328,t33,t333,t339,t342,t343,t344,t346,t347,t348,t349,t353,t36,t365,t367,t369,t375,t376,t380,t391,t393,t395,t397,t398,t401,t404,t424,t425,t427,t444,t445,t449,t451,t452,t455,t457,t459,t460,t462,t470,t477,t483,t487,t489,t494,t496,t497,t5,t500,t502,t504,t506,t508,t51,t513,t517,t523,t524,t525,t528,t53,t534,t536,t538,t539,t540,t541,t544,t545,t546,t548,t55,t550,t552,t553,t554,t555,t556,t557,t558,t559,t560,t562,t563,t564,t566,t568,t569,t57,t572,t573,t575,t576,t577,t580,t581,t582,t585,t586,t59,t590,t592,t593,t594,t599,t6,t60,t600,t601,t604,t606,t607,t609,t61,t611,t612,t613,t614,t616,t617,t620,t621,t622,t625,t626,t627,t630,t632,t633,t634,t635,t637,t638,t639,t641,t642,t643,t644,t645,t646,t648,t651,t654,t655,t66,t660,t661,t665,t668,t669,t670,t674,t676,t678,t679,t68,t680,t683,t685,t695,t697,t698,t699,t7,t700,t701,t702,t703,t705,t707,t711,t712,t713,t716,t717,t718,t719,t72,t725,t726,t727,t729,t732,t736,t739,t74,t741,t743,t744,t747,t75,t751,t755,t756,t758,t759,t761,t764,t766,t770,t772,t774,t776,t777,t778,t782,t784,t785,t787,t788,t793,t794,t797,t799,t8,t801,t802,t804,t805,t807,t808,t811,t813,t814,t818,t822,t824,t827,t828,t831,t832,t833,t835,t837,t838,t839,t840,t842,t843,t844,t845,t846,t847,t848,t849,t850,t857,t859,t86,t860,t866,t867,t87,t870,t875,t877,t88,t883,t884,t885,t887,t889,t89,t895,t9,t90,t900,t904,t907,t909,t91,t910,t911,t912,t913,t914,t915,t916,t917,t918,t919,t92,t921,t924,t926,t929,t93,t932,t933,t934,t936,t937,t938,t939,t94,t940,t943,t944,t945,t947,t948,t951,t956,t957,t959,t96,t961,t965,t967,t968,t969,t97,t971,t972,t973,t975,t977,t979,t98,t980,t981,t982,t983,t985,t986,t990,t994,t995,t996,t997,t998});
end
function M = ft_2(ct)
q1 = ct{1};
q2 = ct{2};
t10 = ct{3};
t100 = ct{4};
t1000 = ct{5};
t1002 = ct{6};
t1003 = ct{7};
t1004 = ct{8};
t1005 = ct{9};
t1007 = ct{10};
t1008 = ct{11};
t1012 = ct{12};
t1014 = ct{13};
t1020 = ct{14};
t1021 = ct{15};
t1023 = ct{16};
t1024 = ct{17};
t1025 = ct{18};
t1026 = ct{19};
t1027 = ct{20};
t1029 = ct{21};
t1033 = ct{22};
t1034 = ct{23};
t1037 = ct{24};
t1039 = ct{25};
t1042 = ct{26};
t1043 = ct{27};
t1044 = ct{28};
t1045 = ct{29};
t1049 = ct{30};
t1050 = ct{31};
t1051 = ct{32};
t1052 = ct{33};
t1053 = ct{34};
t1058 = ct{35};
t1059 = ct{36};
t1062 = ct{37};
t1063 = ct{38};
t1066 = ct{39};
t1073 = ct{40};
t1074 = ct{41};
t1076 = ct{42};
t1077 = ct{43};
t1078 = ct{44};
t1079 = ct{45};
t1080 = ct{46};
t1085 = ct{47};
t1087 = ct{48};
t1088 = ct{49};
t1090 = ct{50};
t1092 = ct{51};
t1094 = ct{52};
t1095 = ct{53};
t1097 = ct{54};
t1103 = ct{55};
t111 = ct{56};
t1111 = ct{57};
t1115 = ct{58};
t1117 = ct{59};
t1118 = ct{60};
t1119 = ct{61};
t112 = ct{62};
t1124 = ct{63};
t1125 = ct{64};
t1128 = ct{65};
t1129 = ct{66};
t113 = ct{67};
t1130 = ct{68};
t1131 = ct{69};
t1135 = ct{70};
t1136 = ct{71};
t114 = ct{72};
t1140 = ct{73};
t1146 = ct{74};
t1150 = ct{75};
t1151 = ct{76};
t1153 = ct{77};
t1154 = ct{78};
t1155 = ct{79};
t1159 = ct{80};
t116 = ct{81};
t1160 = ct{82};
t1163 = ct{83};
t1166 = ct{84};
t1167 = ct{85};
t1168 = ct{86};
t1169 = ct{87};
t117 = ct{88};
t1173 = ct{89};
t1176 = ct{90};
t1181 = ct{91};
t1182 = ct{92};
t1183 = ct{93};
t1186 = ct{94};
t119 = ct{95};
t1193 = ct{96};
t1194 = ct{97};
t1199 = ct{98};
t12 = ct{99};
t120 = ct{100};
t1200 = ct{101};
t1208 = ct{102};
t1209 = ct{103};
t121 = ct{104};
t1210 = ct{105};
t1211 = ct{106};
t1213 = ct{107};
t1214 = ct{108};
t1216 = ct{109};
t1217 = ct{110};
t1218 = ct{111};
t122 = ct{112};
t1223 = ct{113};
t1233 = ct{114};
t1234 = ct{115};
t1242 = ct{116};
t1246 = ct{117};
t1249 = ct{118};
t1250 = ct{119};
t1251 = ct{120};
t1252 = ct{121};
t1259 = ct{122};
t126 = ct{123};
t1274 = ct{124};
t1285 = ct{125};
t1286 = ct{126};
t129 = ct{127};
t13 = ct{128};
t130 = ct{129};
t1303 = ct{130};
t131 = ct{131};
t132 = ct{132};
t1327 = ct{133};
t133 = ct{134};
t1340 = ct{135};
t136 = ct{136};
t1366 = ct{137};
t137 = ct{138};
t138 = ct{139};
t14 = ct{140};
t1403 = ct{141};
t1404 = ct{142};
t1410 = ct{143};
t142 = ct{144};
t143 = ct{145};
t149 = ct{146};
t15 = ct{147};
t150 = ct{148};
t153 = ct{149};
t154 = ct{150};
t155 = ct{151};
t156 = ct{152};
t1568 = ct{153};
t1569 = ct{154};
t16 = ct{155};
t160 = ct{156};
t1601 = ct{157};
t1625 = ct{158};
t164 = ct{159};
t165 = ct{160};
t167 = ct{161};
t1671 = ct{162};
t168 = ct{163};
t1687 = ct{164};
t1699 = ct{165};
t17 = ct{166};
t170 = ct{167};
t171 = ct{168};
t1715 = ct{169};
t172 = ct{170};
t173 = ct{171};
t174 = ct{172};
t176 = ct{173};
t1771 = ct{174};
t1776 = ct{175};
t1777 = ct{176};
t178 = ct{177};
t1782 = ct{178};
t1784 = ct{179};
t1785 = ct{180};
t1789 = ct{181};
t179 = ct{182};
t1797 = ct{183};
t18 = ct{184};
t180 = ct{185};
t1808 = ct{186};
t1810 = ct{187};
t185 = ct{188};
t186 = ct{189};
t1867 = ct{190};
t191 = ct{191};
t1919 = ct{192};
t192 = ct{193};
t1949 = ct{194};
t1969 = ct{195};
t1970 = ct{196};
t1972 = ct{197};
t198 = ct{198};
t1991 = ct{199};
t1992 = ct{200};
t1996 = ct{201};
t200 = ct{202};
t2004 = ct{203};
t2005 = ct{204};
t2013 = ct{205};
t2015 = ct{206};
t202 = ct{207};
t2021 = ct{208};
t203 = ct{209};
t205 = ct{210};
t206 = ct{211};
t207 = ct{212};
t210 = ct{213};
t213 = ct{214};
t214 = ct{215};
t216 = ct{216};
t217 = ct{217};
t220 = ct{218};
t221 = ct{219};
t222 = ct{220};
t223 = ct{221};
t224 = ct{222};
t225 = ct{223};
t227 = ct{224};
t228 = ct{225};
t231 = ct{226};
t236 = ct{227};
t239 = ct{228};
t240 = ct{229};
t242 = ct{230};
t244 = ct{231};
t245 = ct{232};
t246 = ct{233};
t248 = ct{234};
t249 = ct{235};
t250 = ct{236};
t251 = ct{237};
t252 = ct{238};
t253 = ct{239};
t254 = ct{240};
t257 = ct{241};
t261 = ct{242};
t264 = ct{243};
t265 = ct{244};
t267 = ct{245};
t268 = ct{246};
t269 = ct{247};
t271 = ct{248};
t274 = ct{249};
t277 = ct{250};
t279 = ct{251};
t280 = ct{252};
t281 = ct{253};
t284 = ct{254};
t287 = ct{255};
t292 = ct{256};
t293 = ct{257};
t294 = ct{258};
t295 = ct{259};
t298 = ct{260};
t299 = ct{261};
t300 = ct{262};
t301 = ct{263};
t302 = ct{264};
t305 = ct{265};
t307 = ct{266};
t308 = ct{267};
t309 = ct{268};
t31 = ct{269};
t310 = ct{270};
t311 = ct{271};
t312 = ct{272};
t313 = ct{273};
t314 = ct{274};
t318 = ct{275};
t32 = ct{276};
t320 = ct{277};
t321 = ct{278};
t323 = ct{279};
t324 = ct{280};
t327 = ct{281};
t328 = ct{282};
t33 = ct{283};
t333 = ct{284};
t339 = ct{285};
t342 = ct{286};
t343 = ct{287};
t344 = ct{288};
t346 = ct{289};
t347 = ct{290};
t348 = ct{291};
t349 = ct{292};
t353 = ct{293};
t36 = ct{294};
t365 = ct{295};
t367 = ct{296};
t369 = ct{297};
t375 = ct{298};
t376 = ct{299};
t380 = ct{300};
t391 = ct{301};
t393 = ct{302};
t395 = ct{303};
t397 = ct{304};
t398 = ct{305};
t401 = ct{306};
t404 = ct{307};
t424 = ct{308};
t425 = ct{309};
t427 = ct{310};
t444 = ct{311};
t445 = ct{312};
t449 = ct{313};
t451 = ct{314};
t452 = ct{315};
t455 = ct{316};
t457 = ct{317};
t459 = ct{318};
t460 = ct{319};
t462 = ct{320};
t470 = ct{321};
t477 = ct{322};
t483 = ct{323};
t487 = ct{324};
t489 = ct{325};
t494 = ct{326};
t496 = ct{327};
t497 = ct{328};
t5 = ct{329};
t500 = ct{330};
t502 = ct{331};
t504 = ct{332};
t506 = ct{333};
t508 = ct{334};
t51 = ct{335};
t513 = ct{336};
t517 = ct{337};
t523 = ct{338};
t524 = ct{339};
t525 = ct{340};
t528 = ct{341};
t53 = ct{342};
t534 = ct{343};
t536 = ct{344};
t538 = ct{345};
t539 = ct{346};
t540 = ct{347};
t541 = ct{348};
t544 = ct{349};
t545 = ct{350};
t546 = ct{351};
t548 = ct{352};
t55 = ct{353};
t550 = ct{354};
t552 = ct{355};
t553 = ct{356};
t554 = ct{357};
t555 = ct{358};
t556 = ct{359};
t557 = ct{360};
t558 = ct{361};
t559 = ct{362};
t560 = ct{363};
t562 = ct{364};
t563 = ct{365};
t564 = ct{366};
t566 = ct{367};
t568 = ct{368};
t569 = ct{369};
t57 = ct{370};
t572 = ct{371};
t573 = ct{372};
t575 = ct{373};
t576 = ct{374};
t577 = ct{375};
t580 = ct{376};
t581 = ct{377};
t582 = ct{378};
t585 = ct{379};
t586 = ct{380};
t59 = ct{381};
t590 = ct{382};
t592 = ct{383};
t593 = ct{384};
t594 = ct{385};
t599 = ct{386};
t6 = ct{387};
t60 = ct{388};
t600 = ct{389};
t601 = ct{390};
t604 = ct{391};
t606 = ct{392};
t607 = ct{393};
t609 = ct{394};
t61 = ct{395};
t611 = ct{396};
t612 = ct{397};
t613 = ct{398};
t614 = ct{399};
t616 = ct{400};
t617 = ct{401};
t620 = ct{402};
t621 = ct{403};
t622 = ct{404};
t625 = ct{405};
t626 = ct{406};
t627 = ct{407};
t630 = ct{408};
t632 = ct{409};
t633 = ct{410};
t634 = ct{411};
t635 = ct{412};
t637 = ct{413};
t638 = ct{414};
t639 = ct{415};
t641 = ct{416};
t642 = ct{417};
t643 = ct{418};
t644 = ct{419};
t645 = ct{420};
t646 = ct{421};
t648 = ct{422};
t651 = ct{423};
t654 = ct{424};
t655 = ct{425};
t66 = ct{426};
t660 = ct{427};
t661 = ct{428};
t665 = ct{429};
t668 = ct{430};
t669 = ct{431};
t670 = ct{432};
t674 = ct{433};
t676 = ct{434};
t678 = ct{435};
t679 = ct{436};
t68 = ct{437};
t680 = ct{438};
t683 = ct{439};
t685 = ct{440};
t695 = ct{441};
t697 = ct{442};
t698 = ct{443};
t699 = ct{444};
t7 = ct{445};
t700 = ct{446};
t701 = ct{447};
t702 = ct{448};
t703 = ct{449};
t705 = ct{450};
t707 = ct{451};
t711 = ct{452};
t712 = ct{453};
t713 = ct{454};
t716 = ct{455};
t717 = ct{456};
t718 = ct{457};
t719 = ct{458};
t72 = ct{459};
t725 = ct{460};
t726 = ct{461};
t727 = ct{462};
t729 = ct{463};
t732 = ct{464};
t736 = ct{465};
t739 = ct{466};
t74 = ct{467};
t741 = ct{468};
t743 = ct{469};
t744 = ct{470};
t747 = ct{471};
t75 = ct{472};
t751 = ct{473};
t755 = ct{474};
t756 = ct{475};
t758 = ct{476};
t759 = ct{477};
t761 = ct{478};
t764 = ct{479};
t766 = ct{480};
t770 = ct{481};
t772 = ct{482};
t774 = ct{483};
t776 = ct{484};
t777 = ct{485};
t778 = ct{486};
t782 = ct{487};
t784 = ct{488};
t785 = ct{489};
t787 = ct{490};
t788 = ct{491};
t793 = ct{492};
t794 = ct{493};
t797 = ct{494};
t799 = ct{495};
t8 = ct{496};
t801 = ct{497};
t802 = ct{498};
t804 = ct{499};
t805 = ct{500};
t807 = ct{501};
t808 = ct{502};
t811 = ct{503};
t813 = ct{504};
t814 = ct{505};
t818 = ct{506};
t822 = ct{507};
t824 = ct{508};
t827 = ct{509};
t828 = ct{510};
t831 = ct{511};
t832 = ct{512};
t833 = ct{513};
t835 = ct{514};
t837 = ct{515};
t838 = ct{516};
t839 = ct{517};
t840 = ct{518};
t842 = ct{519};
t843 = ct{520};
t844 = ct{521};
t845 = ct{522};
t846 = ct{523};
t847 = ct{524};
t848 = ct{525};
t849 = ct{526};
t850 = ct{527};
t857 = ct{528};
t859 = ct{529};
t86 = ct{530};
t860 = ct{531};
t866 = ct{532};
t867 = ct{533};
t87 = ct{534};
t870 = ct{535};
t875 = ct{536};
t877 = ct{537};
t88 = ct{538};
t883 = ct{539};
t884 = ct{540};
t885 = ct{541};
t887 = ct{542};
t889 = ct{543};
t89 = ct{544};
t895 = ct{545};
t9 = ct{546};
t90 = ct{547};
t900 = ct{548};
t904 = ct{549};
t907 = ct{550};
t909 = ct{551};
t91 = ct{552};
t910 = ct{553};
t911 = ct{554};
t912 = ct{555};
t913 = ct{556};
t914 = ct{557};
t915 = ct{558};
t916 = ct{559};
t917 = ct{560};
t918 = ct{561};
t919 = ct{562};
t92 = ct{563};
t921 = ct{564};
t924 = ct{565};
t926 = ct{566};
t929 = ct{567};
t93 = ct{568};
t932 = ct{569};
t933 = ct{570};
t934 = ct{571};
t936 = ct{572};
t937 = ct{573};
t938 = ct{574};
t939 = ct{575};
t94 = ct{576};
t940 = ct{577};
t943 = ct{578};
t944 = ct{579};
t945 = ct{580};
t947 = ct{581};
t948 = ct{582};
t951 = ct{583};
t956 = ct{584};
t957 = ct{585};
t959 = ct{586};
t96 = ct{587};
t961 = ct{588};
t965 = ct{589};
t967 = ct{590};
t968 = ct{591};
t969 = ct{592};
t97 = ct{593};
t971 = ct{594};
t972 = ct{595};
t973 = ct{596};
t975 = ct{597};
t977 = ct{598};
t979 = ct{599};
t98 = ct{600};
t980 = ct{601};
t981 = ct{602};
t982 = ct{603};
t983 = ct{604};
t985 = ct{605};
t986 = ct{606};
t990 = ct{607};
t994 = ct{608};
t995 = ct{609};
t996 = ct{610};
t997 = ct{611};
t998 = ct{612};
t1238 = t311.*1.144e-2;
t1239 = t312.*1.144e-2;
t1253 = t523.*9.999999999999998e-6;
t1260 = t401.*(-1.2e-4);
t1270 = t550.*9.999999999999998e-6;
t1272 = t462.*(-1.2e-4);
t1283 = t462.*1.2e-4;
t1294 = t548.*1.11e-3;
t1315 = t6.*t228.*(t129+t13.*(t51-t155)).*(-4.466636216449161e-20);
t1318 = t638.*9.999999999999998e-6;
t1324 = t548.*1.12e-3;
t1325 = t639.*3.0e-5;
t1335 = t523.*1.2e-4;
t1342 = t639.*5.0e-5;
t1343 = t550.*1.2e-4;
t1350 = t274.*(t129+t13.*(t51-t155)).*(-4.466636216449161e-20);
t1353 = t638.*2.769999999999999e-3;
t1355 = t639.*5.000000000000004e-4;
t1356 = t274.*(t129+t13.*(t51-t155)).*4.466636216449161e-20;
t1357 = t638.*1.0e-5;
t1365 = t548.*4.988e-2;
t1375 = t726.*3.0e-5;
t1389 = t726.*5.0e-5;
t1392 = t939.*4.466636216449161e-20;
t1396 = t726.*5.000000000000004e-4;
t1405 = t228.*(t156-t236).*(-9.999999999999998e-6);
t1417 = t822.*9.999999999999998e-6;
t1427 = t452.*(t57-t165).*(-3.0e-5);
t1441 = t6.*t228.*(t129+t13.*(t51-t155)).*(-9.999999999999998e-6);
t1444 = t228.*(t156-t236).*(-1.0e-5);
t1446 = t452.*(t57-t165).*(-5.0e-5);
t1450 = t228.*(t156-t236).*(-2.769999999999999e-3);
t1454 = t228.*(t156-t236).*1.0e-5;
t1457 = t228.*(t156-t236).*2.769999999999999e-3;
t1458 = t452.*(t57-t165).*(-5.000000000000004e-4);
t1463 = t822.*1.0e-5;
t1467 = t822.*2.769999999999999e-3;
t1470 = t274.*(t129+t13.*(t51-t155)).*(-9.999999999999998e-6);
t1487 = t6.*t228.*(t129+t13.*(t51-t155)).*(-1.2e-4);
t1491 = t6.*t228.*(t129+t13.*(t51-t155)).*1.2e-4;
t1492 = t939.*9.999999999999998e-6;
t1503 = t274.*(t129+t13.*(t51-t155)).*(-1.2e-4);
t1523 = t939.*1.2e-4;
t1707 = t427+t489+t569+t606;
t1802 = t393+t582+t766+t774;
t1805 = t541+t577+t736+t778;
t1945 = t555+t744+t1002+t1005;
t1953 = t90+t349+t376+t459+t497+t621+t670;
t1954 = t86+t347+t375+t457+t506+t635+t669;
t1965 = t100+t424+t444+t494+t502+t630+t661;
t1985 = t89+t348+t538+t540+t601+t755+t776;
t1999 = t203+t576+t581+t593+t604+t877+t883;
t2017 = -t2015;
t2023 = t1715.*t1808.*2.61155;
t2040 = t1625.*t1919.*(3.41e+2./1.0e+2);
t2043 = t831+t845+t900+t913+t956+t972;
t2048 = t807+t887+t918+t926+t940+t965;
t2056 = t1699.*t1949.*2.61155;
t2058 = t1782.*t1919.*(3.41e+2./1.0e+2);
t2075 = t934+t947+t961+t971+t1052+t1077;
t2095 = t1810.*t1949.*2.61155;
t2191 = t832+t835+t859+t860+t867+t943+t951+t995+t1007;
t256 = t6.*t245;
t270 = t13.*t239;
t273 = t6.*t242;
t278 = -t257;
t303 = -t293;
t306 = -t295;
t315 = t133+t216;
t319 = t8.*t300;
t322 = t15.*t300;
t345 = -t328;
t396 = t131+t250;
t454 = t168+t246;
t456 = -t397;
t480 = t7.*t395;
t481 = t8.*t395;
t485 = t14.*t395;
t486 = t15.*t395;
t510 = t7.*t451;
t511 = t8.*t451;
t512 = t14.*t451;
t514 = t15.*t451;
t515 = -t8.*(t136-t246);
t518 = -t15.*(t136-t246);
t526 = t7.*t513;
t527 = t7.*t517;
t533 = t8.*(t136-t246);
t535 = t14.*t504;
t549 = t7.*t534;
t565 = t176+t294;
t567 = t179+t298;
t597 = t214+t299;
t610 = t150+t324;
t649 = t200+t321;
t675 = t251+t279;
t686 = t138.*t395;
t687 = -t300.*(t53-t132);
t688 = t12.*t116.*t451;
t689 = t12.*t121.*t395;
t690 = t8.*t655;
t691 = -t13.*t117.*(t136-t246);
t692 = t15.*t655;
t696 = t248+t292;
t706 = t137.*t451;
t710 = t13.*t117.*(t136-t246);
t715 = -t711;
t722 = -t171.*(t136-t246);
t728 = t242.*4.9e-4;
t731 = t245.*4.9e-4;
t733 = t250.*4.9e-4;
t734 = -t717;
t735 = -t718;
t737 = -t727;
t748 = t171.*(t136-t246);
t749 = t242.*2.019e-2;
t752 = t245.*2.019e-2;
t753 = t246.*2.019e-2;
t757 = t251.*3.466000000000001e-2;
t762 = t224.*t395;
t771 = t248.*2.324e-2;
t773 = t126+t239+t240;
t779 = t228.*t395;
t780 = -t225.*(t136-t246);
t781 = -t395.*(t53-t132);
t783 = t261.*3.466000000000001e-2;
t786 = t257.*2.324e-2;
t789 = t242.*1.9738e-1;
t791 = t245.*1.9738e-1;
t792 = t246.*1.9738e-1;
t795 = t228.*t451;
t796 = -t451.*(t53-t132);
t798 = -t227.*(t136-t246);
t800 = t293.*4.9e-4;
t803 = t295.*4.9e-4;
t806 = t294.*2.019e-2;
t809 = t298.*2.019e-2;
t820 = -t451.*(t51-t155);
t821 = -t808;
t823 = t451.*(t53-t132);
t826 = (t57-t165).*(t136-t246);
t855 = t294.*1.9738e-1;
t858 = t298.*1.9738e-1;
t863 = t321.*3.466000000000001e-2;
t865 = t323.*3.466000000000001e-2;
t873 = t320.*2.324e-2;
t874 = t324.*2.324e-2;
t896 = t280.*4.466636216449161e-20;
t899 = (t8.*(t57-t165)+t15.*(t136-t246)).^2;
t902 = t339+t342;
t903 = t327+t369;
t988 = t534.*(-3.466000000000001e-2);
t989 = t15.*(t136-t246).*(-3.466000000000001e-2);
t992 = t343.*4.466636216449161e-20;
t993 = t344.*4.466636216449161e-20;
t1001 = t534.*(-2.324e-2);
t1010 = t7.*t986;
t1011 = t534.*2.324e-2;
t1054 = -t451.*(t156-t236);
t1055 = -t395.*(t129+t13.*(t51-t155));
t1064 = t573.*(-2.324e-2);
t1069 = t395.*(t129+t13.*(t51-t155));
t1070 = t573.*2.324e-2;
t1084 = t239.*1.11e-3;
t1091 = t504.*4.466636216449161e-20;
t1098 = t284.*3.0e-5;
t1101 = -t1095;
t1112 = t284.*5.0e-5;
t1114 = t239.*1.12e-3;
t1123 = -t1117;
t1127 = -t1118;
t1132 = t284.*5.000000000000004e-4;
t1137 = t280.*1.0e-5;
t1138 = t323+t707;
t1142 = -t1131;
t1144 = -t614.*(t156-t236);
t1149 = t508+t575;
t1152 = t328.*9.999999999999998e-6;
t1156 = t320+t725;
t1158 = t213+t333+t367;
t1170 = t239.*4.988e-2;
t1177 = -t648.*(t129+t13.*(t51-t155));
t1184 = t280.*2.840000000000012e-3;
t1185 = -t1182;
t1187 = t328.*2.769999999999999e-3;
t1191 = t328.*1.0e-5;
t1192 = t333.*1.11e-3;
t1204 = t343.*1.0e-5;
t1205 = t344.*1.0e-5;
t1215 = -t1199;
t1220 = -t1210;
t1222 = t339.*3.844e-2;
t1225 = -t1216;
t1229 = t397.*1.11e-3;
t1230 = t333.*1.12e-3;
t1232 = t339.*1.12e-3;
t1237 = t339.*8.8e-4;
t1248 = t504.*9.999999999999998e-6;
t1255 = t397.*1.12e-3;
t1256 = t343.*2.840000000000012e-3;
t1257 = t344.*2.840000000000012e-3;
t1263 = t508.*1.11e-3;
t1268 = t333.*4.988e-2;
t1275 = t558.*3.0e-5;
t1292 = t508.*1.12e-3;
t1295 = t558.*5.0e-5;
t1300 = t397.*4.988e-2;
t1301 = t818.*4.466636216449161e-20;
t1302 = t451.*(t51-t155).*(-4.466636216449161e-20);
t1305 = -t1294;
t1312 = t558.*5.000000000000004e-4;
t1316 = t676.*(-9.999999999999998e-6);
t1322 = t504.*1.2e-4;
t1323 = t676.*9.999999999999998e-6;
t1326 = t875.*(-4.466636216449161e-20);
t1328 = -t1324;
t1337 = t508.*4.988e-2;
t1338 = t685.*9.999999999999998e-6;
t1339 = t300.*(t53-t132).*(-9.999999999999998e-6);
t1341 = t253+t504+t523;
t1351 = -t1342;
t1352 = t676.*(-2.769999999999999e-3);
t1354 = t676.*(-1.0e-5);
t1358 = t676.*2.769999999999999e-3;
t1362 = t676.*1.0e-5;
t1369 = -t1365;
t1370 = t685.*2.769999999999999e-3;
t1371 = t300.*(t53-t132).*(-2.769999999999999e-3);
t1373 = t685.*1.0e-5;
t1376 = t300.*(t53-t132).*(-1.0e-5);
t1385 = -t568.*(t8.*(t57-t165)+t15.*(t136-t246));
t1393 = t395.*(t53-t132).*(-9.999999999999998e-6);
t1395 = t568.*(t8.*(t57-t165)+t15.*(t136-t246));
t1400 = -t1392;
t1401 = t225.*(t136-t246).*(-4.000000000000028e-5);
t1406 = t225.*(t136-t246).*4.000000000000028e-5;
t1412 = (t8.*(t57-t165)+t15.*(t136-t246)).*(t154-t321);
t1413 = t227.*(t136-t246).*(-4.000000000000028e-5);
t1416 = t225.*(t136-t246).*(-5.0e-5);
t1419 = t818.*9.999999999999998e-6;
t1420 = -t1417;
t1426 = t225.*(t136-t246).*(-2.81e-3);
t1430 = t395.*(t53-t132).*(-1.0e-5);
t1431 = t227.*(t136-t246).*(-5.0e-5);
t1434 = t395.*(t53-t132).*(-2.769999999999999e-3);
t1438 = t395.*(t53-t132).*1.0e-5;
t1439 = t451.*(t156-t236).*(-4.466636216449161e-20);
t1445 = t227.*(t136-t246).*(-2.81e-3);
t1455 = t227.*(t136-t246).*2.81e-3;
t1456 = t875.*(-9.999999999999998e-6);
t1461 = t451.*(t51-t155).*(-1.0e-5);
t1466 = t875.*9.999999999999998e-6;
t1477 = t797+t843;
t1479 = t818.*1.2e-4;
t1483 = t451.*(t51-t155).*(-2.840000000000012e-3);
t1488 = t451.*(t51-t155).*2.840000000000012e-3;
t1493 = t875.*(-1.2e-4);
t1497 = t875.*1.2e-4;
t1505 = t310+t638+t676;
t1515 = t451.*(t156-t236).*(-9.999999999999998e-6);
t1517 = t451.*(t156-t236).*9.999999999999998e-6;
t1519 = -t889.*(t8.*(t57-t165)+t15.*(t136-t246));
t1528 = t451.*(t156-t236).*(-1.2e-4);
t1533 = t614.*(t156-t236).*(-3.0e-5);
t1539 = t614.*(t156-t236).*(-5.0e-5);
t1557 = t648.*(t129+t13.*(t51-t155)).*(-3.0e-5);
t1558 = t614.*(t156-t236).*(-5.000000000000004e-4);
t1563 = t648.*(t129+t13.*(t51-t155)).*3.0e-5;
t1566 = t648.*(t129+t13.*(t51-t155)).*(-5.0e-5);
t1579 = t648.*(t129+t13.*(t51-t155)).*(-5.000000000000004e-4);
t1587 = t648.*(t129+t13.*(t51-t155)).*5.000000000000004e-4;
t1658 = t401+t818+t838;
t1697 = t380+t449+t563+t634;
t1731 = t425+t483+t616+t625;
t1757 = t550+t870+t875;
t1783 = t365+t536+t713+t743;
t1794 = t889.*(t8.*(t57-t165)+t15.*(t136-t246)).*(-2.900000000000001e-4);
t1795 = t889.*(t8.*(t57-t165)+t15.*(t136-t246)).*(-2.9e-4);
t1798 = t889.*(t8.*(t57-t165)+t15.*(t136-t246)).*(-2.94e-3);
t1883 = t525+t560+t562+t609+t633;
t1885 = t539+t545+t586+t600+t646;
t1930 = t585+t701+t968+t973;
t1935 = t61+t96+t556+t592+t594+t607+t622;
t1960 = t89+t404+t445+t460+t487+t620+t642;
t1983 = t91+t353+t524+t572+t617+t698+t716;
t1993 = t59+t60+t111+t391+t557+t612+t626+t729+t764;
t2008 = t1707.*t1715.*2.61155;
t2022 = t1707.*t1808.*2.61155;
t2025 = -t2023;
t2036 = t59+t60+t111+t683+t739+t747+t793+t1023+t1025;
t2041 = -t2040;
t2042 = t833+t839+t904+t917+t936+t983;
t2059 = -t2058;
t2068 = (t252.*t2043)./2.0;
t2071 = (t314.*t2043)./2.0;
t2076 = t1776.*t1953.*(3.41e+2./1.0e+2);
t2078 = t910+t919+t929+t938+t1079+t1119;
t2081 = t937+t959+t975+t1008+t1021+t1078;
t2086 = (t544.*t2048)./2.0;
t2092 = t1805.*t1954.*(3.41e+2./1.0e+2);
t2094 = (t654.*t2048)./2.0;
t2096 = t1802.*t1965.*3.38795;
t2099 = (t252.*t2075)./2.0;
t2105 = t1776.*t1985.*(3.41e+2./1.0e+2);
t2107 = (t346.*(-t909+t910+t929+t938+t1079+t1119))./2.0;
t2108 = (t455.*t2075)./2.0;
t2116 = (t544.*(-t909+t910+t929+t938+t1079+t1119))./2.0;
t2142 = t1953.*t1985.*(3.41e+2./1.0e+2);
t2168 = t1945.*t1999.*3.38795;
t2183 = t805+t811+t847+t849+t895+t911+t945+t1004+t1044;
t2184 = t837+t840+t846+t884+t885+t932+t948+t957+t982;
t2207 = (t313.*t2191)./2.0;
t289 = -t273;
t336 = t7.*t315;
t340 = t14.*t315;
t463 = t396.^2;
t516 = -t485;
t530 = -t512;
t591 = t178+t303;
t596 = t185+t306;
t671 = t256+t264;
t708 = -t686;
t720 = -t8.*(t273+t14.*(t51-t155));
t723 = -t15.*(t273+t14.*(t51-t155));
t740 = -t728;
t742 = -t731;
t763 = -t749;
t765 = t273.*4.9e-4;
t769 = t256.*2.019e-2;
t812 = t256.*1.9738e-1;
t815 = t254.*t396;
t817 = -t806;
t819 = -t7.*t396.*(t57-t165);
t825 = -t809;
t836 = t249+t480;
t841 = t7.*t396.*(t57-t165);
t854 = t142+t270+t271;
t856 = t245+t510;
t864 = t322.*3.466000000000001e-2;
t871 = t268+t518;
t872 = t319.*2.324e-2;
t878 = -t863;
t880 = -t865;
t881 = (t485+t7.*(t53-t132)).^2;
t890 = t302.*t396;
t893 = -t873;
t897 = t269+t533;
t901 = -t896;
t920 = -t315.*(t156-t236);
t930 = t480.*4.9e-4;
t931 = t485.*4.9e-4;
t941 = t480.*2.019e-2;
t942 = t485.*2.019e-2;
t950 = t8.*t396.*3.466000000000001e-2;
t952 = t486.*3.466000000000001e-2;
t953 = t510.*4.9e-4;
t955 = t512.*4.9e-4;
t962 = t481.*2.324e-2;
t963 = t510.*2.019e-2;
t964 = t15.*t396.*2.324e-2;
t966 = t512.*2.019e-2;
t987 = t514.*3.466000000000001e-2;
t999 = t533.*(-2.324e-2);
t1006 = -t993;
t1009 = t511.*2.324e-2;
t1017 = t480.*1.9738e-1;
t1018 = t485.*1.9738e-1;
t1031 = t265+t690;
t1040 = t549.*(-2.324e-2);
t1046 = t510.*1.9738e-1;
t1047 = t512.*1.9738e-1;
t1056 = -t396.*(t167+t7.*(t55-t130));
t1057 = t549.*2.324e-2;
t1060 = t281+t692;
t1072 = t270.*9.999999999999998e-6;
t1093 = t486+t526;
t1105 = t481+t549;
t1107 = -t567.*(t156-t236);
t1108 = t396.*t597;
t1110 = t270.*1.0e-5;
t1116 = t270.*2.769999999999999e-3;
t1120 = t396.*t610;
t1121 = t690.*3.466000000000001e-2;
t1126 = t514+t546;
t1133 = t567.*(t156-t236);
t1134 = t692.*2.324e-2;
t1139 = -t565.*(t129+t13.*(t51-t155));
t1143 = -t1132;
t1148 = t511+t573;
t1162 = -t1152;
t1164 = t8.*(t273+t14.*(t51-t155)).*(-3.466000000000001e-2);
t1171 = t15.*(t273+t14.*(t51-t155)).*(-2.324e-2);
t1179 = t396.*t696;
t1180 = t15.*(t273+t14.*(t51-t155)).*2.324e-2;
t1195 = -t1187;
t1196 = t686.*4.466636216449161e-20;
t1197 = t688.*4.466636216449161e-20;
t1198 = t689.*4.466636216449161e-20;
t1203 = t14.*(t515+t15.*(t57-t165)).*(t57-t165);
t1219 = t706.*4.466636216449161e-20;
t1226 = (t515+t15.*(t57-t165)).*(t74-t186);
t1235 = -t1222;
t1240 = -t1229;
t1243 = -t1232;
t1247 = -t1237;
t1254 = t762.*4.466636216449161e-20;
t1258 = t231+t398+t456;
t1261 = -t1255;
t1262 = -t1256;
t1264 = t535.*3.0e-5;
t1269 = t779.*4.466636216449161e-20;
t1276 = t535.*5.0e-5;
t1278 = (t515+t15.*(t57-t165)).*(t149-t160);
t1281 = t8.*(t485+t7.*(t53-t132)).*(-3.466000000000001e-2);
t1284 = t823.*(-4.466636216449161e-20);
t1290 = t8.*(t485+t7.*(t53-t132)).*3.466000000000001e-2;
t1291 = t823.*4.466636216449161e-20;
t1293 = t535.*5.000000000000004e-4;
t1299 = t15.*(t485+t7.*(t53-t132)).*(-2.324e-2);
t1306 = t396.*t857;
t1311 = -t1300;
t1317 = -t1312;
t1330 = t7.*(t485+t7.*(t53-t132)).*(t156-t236);
t1331 = -t8.*t396.*(t8.*(t57-t165)+t15.*(t136-t246));
t1333 = (t129+t13.*(t51-t155)).*(t485+t7.*(t53-t132));
t1336 = -t396.*(t515+t15.*(t57-t165));
t1345 = t710.*(-4.000000000000028e-5);
t1346 = t8.*t396.*(t8.*(t57-t165)+t15.*(t136-t246));
t1348 = -t452.*(t515+t15.*(t57-t165));
t1349 = (t515+t15.*(t57-t165)).*(t136-t246);
t1364 = t710.*(-5.0e-5);
t1367 = t710.*5.0e-5;
t1372 = t748.*(-4.000000000000028e-5);
t1374 = t686.*1.0e-5;
t1377 = t688.*1.0e-5;
t1378 = t710.*(-2.81e-3);
t1379 = t689.*1.0e-5;
t1381 = t710.*2.81e-3;
t1382 = t315.*(t156-t236).*(-4.466636216449161e-20);
t1387 = t706.*1.0e-5;
t1388 = t748.*(-5.0e-5);
t1390 = t315.*(t156-t236).*4.466636216449161e-20;
t1391 = t748.*5.0e-5;
t1397 = t748.*(-2.81e-3);
t1398 = t284+t535+t558;
t1402 = -t655.*(t485+t7.*(t53-t132));
t1407 = t686.*2.840000000000012e-3;
t1408 = t688.*2.840000000000012e-3;
t1409 = t689.*2.840000000000012e-3;
t1411 = t795.*9.999999999999998e-6;
t1414 = t762.*1.0e-5;
t1418 = t706.*2.840000000000012e-3;
t1424 = -t675.*(t8.*(t57-t165)+t15.*(t136-t246));
t1428 = t779.*1.0e-5;
t1429 = t826.*3.0e-5;
t1440 = t1069.*(-4.466636216449161e-20);
t1442 = t795.*1.0e-5;
t1443 = t823.*(-1.0e-5);
t1447 = t826.*5.0e-5;
t1448 = t1069.*4.466636216449161e-20;
t1449 = t795.*2.769999999999999e-3;
t1453 = t823.*1.0e-5;
t1459 = t826.*5.000000000000004e-4;
t1460 = t762.*2.840000000000012e-3;
t1465 = t779+t823;
t1471 = t779.*2.840000000000012e-3;
t1476 = t823.*(-2.840000000000012e-3);
t1480 = t823.*2.840000000000012e-3;
t1484 = -t1479;
t1485 = t315.*(t156-t236).*(-9.999999999999998e-6);
t1495 = t899.*2.9e-4;
t1499 = t899.*2.900000000000001e-4;
t1501 = t280+t688+t689;
t1504 = t287+t685+t687;
t1507 = t899.*2.94e-3;
t1516 = t1069.*(-9.999999999999998e-6);
t1518 = t396.*(t167+t7.*(t55-t130)).*(-4.000000000000028e-5);
t1520 = t396.*(t167+t7.*(t55-t130)).*(-3.0e-5);
t1521 = t315.*(t156-t236).*(-1.2e-4);
t1522 = t396.*(t167+t7.*(t55-t130)).*4.000000000000028e-5;
t1524 = t396.*(t167+t7.*(t55-t130)).*(-2.32e-3);
t1529 = t1069.*(-1.2e-4);
t1531 = t1069.*1.2e-4;
t1532 = t565.*(t129+t13.*(t51-t155)).*(-3.0e-5);
t1536 = t565.*(t129+t13.*(t51-t155)).*(-5.0e-5);
t1547 = t565.*(t129+t13.*(t51-t155)).*(-5.000000000000004e-4);
t1602 = t345+t781+t795;
t1603 = t343+t762+t820;
t1627 = t1054+t1069;
t1678 = t396.*(t515+t15.*(t57-t165)).*(-2.2e-4);
t1682 = t396.*(t515+t15.*(t57-t165)).*(-2.900000000000001e-4);
t1689 = t396.*(t515+t15.*(t57-t165)).*(-7.950000000000001e-3);
t1690 = t452.*(t515+t15.*(t57-t165)).*(-1.089e-2);
t1691 = t452.*(t515+t15.*(t57-t165)).*(-2.9e-4);
t1695 = t452.*(t515+t15.*(t57-t165)).*(-2.2e-4);
t1716 = t655.*(t485+t7.*(t53-t132)).*(-4.000000000000028e-5);
t1717 = t655.*(t485+t7.*(t53-t132)).*(-3.0e-5);
t1720 = t655.*(t485+t7.*(t53-t132)).*4.000000000000028e-5;
t1723 = t1395.*(-2.9e-4);
t1724 = t1395.*(-2.900000000000001e-4);
M = ft_3({q1,q2,t10,t1000,t1003,t1006,t1009,t1010,t1011,t1012,t1014,t1017,t1018,t1020,t1024,t1026,t1027,t1029,t1031,t1033,t1034,t1037,t1039,t1042,t1043,t1045,t1046,t1047,t1049,t1050,t1051,t1053,t1056,t1057,t1058,t1059,t1060,t1062,t1063,t1066,t1070,t1072,t1073,t1074,t1076,t1079,t1080,t1084,t1085,t1087,t1088,t1090,t1091,t1092,t1093,t1094,t1095,t1097,t1098,t1101,t1103,t1105,t1107,t1108,t1110,t1111,t1112,t1114,t1115,t1116,t1117,t1119,t112,t1120,t1121,t1123,t1124,t1125,t1126,t1127,t1128,t1129,t113,t1130,t1131,t1132,t1133,t1134,t1135,t1136,t1137,t1138,t1139,t114,t1140,t1142,t1143,t1144,t1146,t1148,t1149,t1150,t1151,t1153,t1154,t1155,t1156,t1159,t1160,t1162,t1163,t1164,t1166,t1167,t1168,t1169,t1170,t1173,t1176,t1177,t1179,t1180,t1181,t1182,t1183,t1184,t1185,t1186,t119,t1191,t1192,t1193,t1194,t1195,t1196,t1197,t1198,t120,t1200,t1203,t1204,t1205,t1208,t1209,t121,t1211,t1213,t1214,t1215,t1217,t1218,t1219,t122,t1220,t1222,t1223,t1225,t1226,t1229,t1230,t1232,t1233,t1234,t1235,t1238,t1239,t1240,t1242,t1243,t1246,t1247,t1248,t1249,t1250,t1251,t1252,t1253,t1254,t1255,t1257,t1259,t1260,t1261,t1262,t1263,t1264,t1268,t1269,t1270,t1272,t1274,t1275,t1276,t1278,t1283,t1284,t1285,t1286,t129,t1290,t1291,t1292,t1293,t1295,t1299,t13,t130,t1300,t1301,t1302,t1303,t1305,t1306,t1311,t1312,t1315,t1317,t1318,t132,t1322,t1323,t1324,t1325,t1326,t1327,t1328,t1330,t1333,t1335,t1336,t1337,t1338,t1339,t1340,t1341,t1342,t1343,t1345,t1346,t1348,t1349,t1351,t1353,t1355,t1356,t1357,t1358,t136,t1362,t1364,t1365,t1366,t1367,t1369,t1370,t1371,t1372,t1373,t1374,t1375,t1376,t1377,t1379,t1381,t1387,t1389,t1390,t1391,t1393,t1395,t1396,t1397,t1398,t14,t1400,t1402,t1403,t1404,t1405,t1406,t1407,t1408,t1409,t1410,t1411,t1412,t1413,t1414,t1416,t1417,t1418,t1419,t1420,t1424,t1426,t1427,t1428,t1429,t143,t1431,t1434,t1438,t1439,t1441,t1442,t1446,t1447,t1448,t1449,t1453,t1454,t1455,t1457,t1458,t1459,t1460,t1461,t1463,t1465,t1466,t1467,t1470,t1471,t1480,t1484,t1485,t1488,t1491,t1492,t1495,t1497,t1499,t15,t1501,t1503,t1504,t1505,t1507,t1516,t1517,t1518,t1519,t1520,t1521,t1522,t1523,t1524,t1528,t1529,t153,t1531,t1532,t1533,t1536,t1539,t1547,t155,t1558,t156,t1563,t1566,t1568,t1569,t1587,t16,t1601,t1603,t1625,t1627,t164,t165,t1658,t167,t1671,t1678,t1682,t1687,t1689,t1690,t1691,t1695,t1697,t1699,t17,t170,t1707,t1715,t1717,t172,t1720,t173,t1731,t174,t1757,t1771,t1776,t1777,t1782,t1783,t1784,t1785,t1789,t1794,t1795,t1797,t1798,t18,t180,t1802,t1805,t1808,t1810,t1867,t1883,t1885,t191,t1919,t192,t1930,t1935,t1945,t1949,t1953,t1954,t1960,t1965,t1969,t1970,t1972,t198,t1983,t1985,t1991,t1992,t1993,t1996,t1999,t2004,t2005,t2008,t2013,t2017,t202,t2021,t2022,t2025,t203,t2036,t2041,t2042,t2043,t2048,t205,t2056,t2059,t206,t2068,t207,t2071,t2075,t2076,t2081,t2086,t2092,t2094,t2095,t2096,t2099,t210,t2105,t2107,t2108,t2116,t2142,t2168,t217,t2183,t2184,t2191,t220,t2207,t221,t222,t223,t225,t227,t228,t231,t236,t242,t244,t246,t252,t257,t261,t267,t273,t277,t278,t289,t300,t301,t305,t307,t308,t309,t31,t311,t312,t313,t314,t315,t318,t319,t32,t322,t328,t33,t333,t336,t340,t342,t344,t346,t36,t395,t396,t397,t451,t452,t455,t462,t463,t470,t477,t485,t496,t5,t500,t51,t513,t515,t516,t528,t53,t530,t533,t534,t544,t55,t552,t553,t554,t559,t564,t565,t566,t567,t57,t580,t590,t591,t596,t599,t6,t61,t611,t613,t614,t627,t632,t637,t639,t641,t643,t644,t645,t648,t651,t654,t655,t66,t660,t665,t668,t671,t674,t675,t678,t679,t68,t680,t695,t697,t699,t7,t700,t702,t703,t705,t706,t708,t710,t711,t712,t715,t717,t719,t72,t720,t723,t725,t726,t727,t732,t733,t734,t735,t737,t740,t741,t742,t748,t75,t751,t752,t753,t756,t757,t758,t759,t761,t763,t765,t769,t770,t771,t772,t773,t777,t780,t782,t783,t784,t785,t786,t787,t788,t789,t791,t792,t794,t795,t798,t799,t8,t800,t801,t802,t803,t804,t812,t813,t814,t815,t817,t821,t822,t824,t825,t826,t827,t828,t836,t841,t842,t844,t848,t850,t854,t855,t856,t858,t86,t864,t865,t866,t87,t872,t873,t874,t878,t88,t880,t881,t889,t89,t890,t893,t896,t899,t9,t90,t901,t902,t907,t909,t91,t910,t912,t914,t915,t916,t92,t920,t921,t924,t929,t93,t930,t931,t933,t938,t939,t94,t941,t942,t944,t950,t952,t953,t955,t96,t962,t963,t964,t966,t967,t969,t97,t977,t979,t98,t980,t981,t985,t986,t987,t988,t989,t990,t992,t994,t996,t997,t998,t999});
end
function M = ft_3(ct)
q1 = ct{1};
q2 = ct{2};
t10 = ct{3};
t1000 = ct{4};
t1003 = ct{5};
t1006 = ct{6};
t1009 = ct{7};
t1010 = ct{8};
t1011 = ct{9};
t1012 = ct{10};
t1014 = ct{11};
t1017 = ct{12};
t1018 = ct{13};
t1020 = ct{14};
t1024 = ct{15};
t1026 = ct{16};
t1027 = ct{17};
t1029 = ct{18};
t1031 = ct{19};
t1033 = ct{20};
t1034 = ct{21};
t1037 = ct{22};
t1039 = ct{23};
t1042 = ct{24};
t1043 = ct{25};
t1045 = ct{26};
t1046 = ct{27};
t1047 = ct{28};
t1049 = ct{29};
t1050 = ct{30};
t1051 = ct{31};
t1053 = ct{32};
t1056 = ct{33};
t1057 = ct{34};
t1058 = ct{35};
t1059 = ct{36};
t1060 = ct{37};
t1062 = ct{38};
t1063 = ct{39};
t1066 = ct{40};
t1070 = ct{41};
t1072 = ct{42};
t1073 = ct{43};
t1074 = ct{44};
t1076 = ct{45};
t1079 = ct{46};
t1080 = ct{47};
t1084 = ct{48};
t1085 = ct{49};
t1087 = ct{50};
t1088 = ct{51};
t1090 = ct{52};
t1091 = ct{53};
t1092 = ct{54};
t1093 = ct{55};
t1094 = ct{56};
t1095 = ct{57};
t1097 = ct{58};
t1098 = ct{59};
t1101 = ct{60};
t1103 = ct{61};
t1105 = ct{62};
t1107 = ct{63};
t1108 = ct{64};
t1110 = ct{65};
t1111 = ct{66};
t1112 = ct{67};
t1114 = ct{68};
t1115 = ct{69};
t1116 = ct{70};
t1117 = ct{71};
t1119 = ct{72};
t112 = ct{73};
t1120 = ct{74};
t1121 = ct{75};
t1123 = ct{76};
t1124 = ct{77};
t1125 = ct{78};
t1126 = ct{79};
t1127 = ct{80};
t1128 = ct{81};
t1129 = ct{82};
t113 = ct{83};
t1130 = ct{84};
t1131 = ct{85};
t1132 = ct{86};
t1133 = ct{87};
t1134 = ct{88};
t1135 = ct{89};
t1136 = ct{90};
t1137 = ct{91};
t1138 = ct{92};
t1139 = ct{93};
t114 = ct{94};
t1140 = ct{95};
t1142 = ct{96};
t1143 = ct{97};
t1144 = ct{98};
t1146 = ct{99};
t1148 = ct{100};
t1149 = ct{101};
t1150 = ct{102};
t1151 = ct{103};
t1153 = ct{104};
t1154 = ct{105};
t1155 = ct{106};
t1156 = ct{107};
t1159 = ct{108};
t1160 = ct{109};
t1162 = ct{110};
t1163 = ct{111};
t1164 = ct{112};
t1166 = ct{113};
t1167 = ct{114};
t1168 = ct{115};
t1169 = ct{116};
t1170 = ct{117};
t1173 = ct{118};
t1176 = ct{119};
t1177 = ct{120};
t1179 = ct{121};
t1180 = ct{122};
t1181 = ct{123};
t1182 = ct{124};
t1183 = ct{125};
t1184 = ct{126};
t1185 = ct{127};
t1186 = ct{128};
t119 = ct{129};
t1191 = ct{130};
t1192 = ct{131};
t1193 = ct{132};
t1194 = ct{133};
t1195 = ct{134};
t1196 = ct{135};
t1197 = ct{136};
t1198 = ct{137};
t120 = ct{138};
t1200 = ct{139};
t1203 = ct{140};
t1204 = ct{141};
t1205 = ct{142};
t1208 = ct{143};
t1209 = ct{144};
t121 = ct{145};
t1211 = ct{146};
t1213 = ct{147};
t1214 = ct{148};
t1215 = ct{149};
t1217 = ct{150};
t1218 = ct{151};
t1219 = ct{152};
t122 = ct{153};
t1220 = ct{154};
t1222 = ct{155};
t1223 = ct{156};
t1225 = ct{157};
t1226 = ct{158};
t1229 = ct{159};
t1230 = ct{160};
t1232 = ct{161};
t1233 = ct{162};
t1234 = ct{163};
t1235 = ct{164};
t1238 = ct{165};
t1239 = ct{166};
t1240 = ct{167};
t1242 = ct{168};
t1243 = ct{169};
t1246 = ct{170};
t1247 = ct{171};
t1248 = ct{172};
t1249 = ct{173};
t1250 = ct{174};
t1251 = ct{175};
t1252 = ct{176};
t1253 = ct{177};
t1254 = ct{178};
t1255 = ct{179};
t1257 = ct{180};
t1259 = ct{181};
t1260 = ct{182};
t1261 = ct{183};
t1262 = ct{184};
t1263 = ct{185};
t1264 = ct{186};
t1268 = ct{187};
t1269 = ct{188};
t1270 = ct{189};
t1272 = ct{190};
t1274 = ct{191};
t1275 = ct{192};
t1276 = ct{193};
t1278 = ct{194};
t1283 = ct{195};
t1284 = ct{196};
t1285 = ct{197};
t1286 = ct{198};
t129 = ct{199};
t1290 = ct{200};
t1291 = ct{201};
t1292 = ct{202};
t1293 = ct{203};
t1295 = ct{204};
t1299 = ct{205};
t13 = ct{206};
t130 = ct{207};
t1300 = ct{208};
t1301 = ct{209};
t1302 = ct{210};
t1303 = ct{211};
t1305 = ct{212};
t1306 = ct{213};
t1311 = ct{214};
t1312 = ct{215};
t1315 = ct{216};
t1317 = ct{217};
t1318 = ct{218};
t132 = ct{219};
t1322 = ct{220};
t1323 = ct{221};
t1324 = ct{222};
t1325 = ct{223};
t1326 = ct{224};
t1327 = ct{225};
t1328 = ct{226};
t1330 = ct{227};
t1333 = ct{228};
t1335 = ct{229};
t1336 = ct{230};
t1337 = ct{231};
t1338 = ct{232};
t1339 = ct{233};
t1340 = ct{234};
t1341 = ct{235};
t1342 = ct{236};
t1343 = ct{237};
t1345 = ct{238};
t1346 = ct{239};
t1348 = ct{240};
t1349 = ct{241};
t1351 = ct{242};
t1353 = ct{243};
t1355 = ct{244};
t1356 = ct{245};
t1357 = ct{246};
t1358 = ct{247};
t136 = ct{248};
t1362 = ct{249};
t1364 = ct{250};
t1365 = ct{251};
t1366 = ct{252};
t1367 = ct{253};
t1369 = ct{254};
t1370 = ct{255};
t1371 = ct{256};
t1372 = ct{257};
t1373 = ct{258};
t1374 = ct{259};
t1375 = ct{260};
t1376 = ct{261};
t1377 = ct{262};
t1379 = ct{263};
t1381 = ct{264};
t1387 = ct{265};
t1389 = ct{266};
t1390 = ct{267};
t1391 = ct{268};
t1393 = ct{269};
t1395 = ct{270};
t1396 = ct{271};
t1397 = ct{272};
t1398 = ct{273};
t14 = ct{274};
t1400 = ct{275};
t1402 = ct{276};
t1403 = ct{277};
t1404 = ct{278};
t1405 = ct{279};
t1406 = ct{280};
t1407 = ct{281};
t1408 = ct{282};
t1409 = ct{283};
t1410 = ct{284};
t1411 = ct{285};
t1412 = ct{286};
t1413 = ct{287};
t1414 = ct{288};
t1416 = ct{289};
t1417 = ct{290};
t1418 = ct{291};
t1419 = ct{292};
t1420 = ct{293};
t1424 = ct{294};
t1426 = ct{295};
t1427 = ct{296};
t1428 = ct{297};
t1429 = ct{298};
t143 = ct{299};
t1431 = ct{300};
t1434 = ct{301};
t1438 = ct{302};
t1439 = ct{303};
t1441 = ct{304};
t1442 = ct{305};
t1446 = ct{306};
t1447 = ct{307};
t1448 = ct{308};
t1449 = ct{309};
t1453 = ct{310};
t1454 = ct{311};
t1455 = ct{312};
t1457 = ct{313};
t1458 = ct{314};
t1459 = ct{315};
t1460 = ct{316};
t1461 = ct{317};
t1463 = ct{318};
t1465 = ct{319};
t1466 = ct{320};
t1467 = ct{321};
t1470 = ct{322};
t1471 = ct{323};
t1480 = ct{324};
t1484 = ct{325};
t1485 = ct{326};
t1488 = ct{327};
t1491 = ct{328};
t1492 = ct{329};
t1495 = ct{330};
t1497 = ct{331};
t1499 = ct{332};
t15 = ct{333};
t1501 = ct{334};
t1503 = ct{335};
t1504 = ct{336};
t1505 = ct{337};
t1507 = ct{338};
t1516 = ct{339};
t1517 = ct{340};
t1518 = ct{341};
t1519 = ct{342};
t1520 = ct{343};
t1521 = ct{344};
t1522 = ct{345};
t1523 = ct{346};
t1524 = ct{347};
t1528 = ct{348};
t1529 = ct{349};
t153 = ct{350};
t1531 = ct{351};
t1532 = ct{352};
t1533 = ct{353};
t1536 = ct{354};
t1539 = ct{355};
t1547 = ct{356};
t155 = ct{357};
t1558 = ct{358};
t156 = ct{359};
t1563 = ct{360};
t1566 = ct{361};
t1568 = ct{362};
t1569 = ct{363};
t1587 = ct{364};
t16 = ct{365};
t1601 = ct{366};
t1603 = ct{367};
t1625 = ct{368};
t1627 = ct{369};
t164 = ct{370};
t165 = ct{371};
t1658 = ct{372};
t167 = ct{373};
t1671 = ct{374};
t1678 = ct{375};
t1682 = ct{376};
t1687 = ct{377};
t1689 = ct{378};
t1690 = ct{379};
t1691 = ct{380};
t1695 = ct{381};
t1697 = ct{382};
t1699 = ct{383};
t17 = ct{384};
t170 = ct{385};
t1707 = ct{386};
t1715 = ct{387};
t1717 = ct{388};
t172 = ct{389};
t1720 = ct{390};
t173 = ct{391};
t1731 = ct{392};
t174 = ct{393};
t1757 = ct{394};
t1771 = ct{395};
t1776 = ct{396};
t1777 = ct{397};
t1782 = ct{398};
t1783 = ct{399};
t1784 = ct{400};
t1785 = ct{401};
t1789 = ct{402};
t1794 = ct{403};
t1795 = ct{404};
t1797 = ct{405};
t1798 = ct{406};
t18 = ct{407};
t180 = ct{408};
t1802 = ct{409};
t1805 = ct{410};
t1808 = ct{411};
t1810 = ct{412};
t1867 = ct{413};
t1883 = ct{414};
t1885 = ct{415};
t191 = ct{416};
t1919 = ct{417};
t192 = ct{418};
t1930 = ct{419};
t1935 = ct{420};
t1945 = ct{421};
t1949 = ct{422};
t1953 = ct{423};
t1954 = ct{424};
t1960 = ct{425};
t1965 = ct{426};
t1969 = ct{427};
t1970 = ct{428};
t1972 = ct{429};
t198 = ct{430};
t1983 = ct{431};
t1985 = ct{432};
t1991 = ct{433};
t1992 = ct{434};
t1993 = ct{435};
t1996 = ct{436};
t1999 = ct{437};
t2004 = ct{438};
t2005 = ct{439};
t2008 = ct{440};
t2013 = ct{441};
t2017 = ct{442};
t202 = ct{443};
t2021 = ct{444};
t2022 = ct{445};
t2025 = ct{446};
t203 = ct{447};
t2036 = ct{448};
t2041 = ct{449};
t2042 = ct{450};
t2043 = ct{451};
t2048 = ct{452};
t205 = ct{453};
t2056 = ct{454};
t2059 = ct{455};
t206 = ct{456};
t2068 = ct{457};
t207 = ct{458};
t2071 = ct{459};
t2075 = ct{460};
t2076 = ct{461};
t2081 = ct{462};
t2086 = ct{463};
t2092 = ct{464};
t2094 = ct{465};
t2095 = ct{466};
t2096 = ct{467};
t2099 = ct{468};
t210 = ct{469};
t2105 = ct{470};
t2107 = ct{471};
t2108 = ct{472};
t2116 = ct{473};
t2142 = ct{474};
t2168 = ct{475};
t217 = ct{476};
t2183 = ct{477};
t2184 = ct{478};
t2191 = ct{479};
t220 = ct{480};
t2207 = ct{481};
t221 = ct{482};
t222 = ct{483};
t223 = ct{484};
t225 = ct{485};
t227 = ct{486};
t228 = ct{487};
t231 = ct{488};
t236 = ct{489};
t242 = ct{490};
t244 = ct{491};
t246 = ct{492};
t252 = ct{493};
t257 = ct{494};
t261 = ct{495};
t267 = ct{496};
t273 = ct{497};
t277 = ct{498};
t278 = ct{499};
t289 = ct{500};
t300 = ct{501};
t301 = ct{502};
t305 = ct{503};
t307 = ct{504};
t308 = ct{505};
t309 = ct{506};
t31 = ct{507};
t311 = ct{508};
t312 = ct{509};
t313 = ct{510};
t314 = ct{511};
t315 = ct{512};
t318 = ct{513};
t319 = ct{514};
t32 = ct{515};
t322 = ct{516};
t328 = ct{517};
t33 = ct{518};
t333 = ct{519};
t336 = ct{520};
t340 = ct{521};
t342 = ct{522};
t344 = ct{523};
t346 = ct{524};
t36 = ct{525};
t395 = ct{526};
t396 = ct{527};
t397 = ct{528};
t451 = ct{529};
t452 = ct{530};
t455 = ct{531};
t462 = ct{532};
t463 = ct{533};
t470 = ct{534};
t477 = ct{535};
t485 = ct{536};
t496 = ct{537};
t5 = ct{538};
t500 = ct{539};
t51 = ct{540};
t513 = ct{541};
t515 = ct{542};
t516 = ct{543};
t528 = ct{544};
t53 = ct{545};
t530 = ct{546};
t533 = ct{547};
t534 = ct{548};
t544 = ct{549};
t55 = ct{550};
t552 = ct{551};
t553 = ct{552};
t554 = ct{553};
t559 = ct{554};
t564 = ct{555};
t565 = ct{556};
t566 = ct{557};
t567 = ct{558};
t57 = ct{559};
t580 = ct{560};
t590 = ct{561};
t591 = ct{562};
t596 = ct{563};
t599 = ct{564};
t6 = ct{565};
t61 = ct{566};
t611 = ct{567};
t613 = ct{568};
t614 = ct{569};
t627 = ct{570};
t632 = ct{571};
t637 = ct{572};
t639 = ct{573};
t641 = ct{574};
t643 = ct{575};
t644 = ct{576};
t645 = ct{577};
t648 = ct{578};
t651 = ct{579};
t654 = ct{580};
t655 = ct{581};
t66 = ct{582};
t660 = ct{583};
t665 = ct{584};
t668 = ct{585};
t671 = ct{586};
t674 = ct{587};
t675 = ct{588};
t678 = ct{589};
t679 = ct{590};
t68 = ct{591};
t680 = ct{592};
t695 = ct{593};
t697 = ct{594};
t699 = ct{595};
t7 = ct{596};
t700 = ct{597};
t702 = ct{598};
t703 = ct{599};
t705 = ct{600};
t706 = ct{601};
t708 = ct{602};
t710 = ct{603};
t711 = ct{604};
t712 = ct{605};
t715 = ct{606};
t717 = ct{607};
t719 = ct{608};
t72 = ct{609};
t720 = ct{610};
t723 = ct{611};
t725 = ct{612};
t726 = ct{613};
t727 = ct{614};
t732 = ct{615};
t733 = ct{616};
t734 = ct{617};
t735 = ct{618};
t737 = ct{619};
t740 = ct{620};
t741 = ct{621};
t742 = ct{622};
t748 = ct{623};
t75 = ct{624};
t751 = ct{625};
t752 = ct{626};
t753 = ct{627};
t756 = ct{628};
t757 = ct{629};
t758 = ct{630};
t759 = ct{631};
t761 = ct{632};
t763 = ct{633};
t765 = ct{634};
t769 = ct{635};
t770 = ct{636};
t771 = ct{637};
t772 = ct{638};
t773 = ct{639};
t777 = ct{640};
t780 = ct{641};
t782 = ct{642};
t783 = ct{643};
t784 = ct{644};
t785 = ct{645};
t786 = ct{646};
t787 = ct{647};
t788 = ct{648};
t789 = ct{649};
t791 = ct{650};
t792 = ct{651};
t794 = ct{652};
t795 = ct{653};
t798 = ct{654};
t799 = ct{655};
t8 = ct{656};
t800 = ct{657};
t801 = ct{658};
t802 = ct{659};
t803 = ct{660};
t804 = ct{661};
t812 = ct{662};
t813 = ct{663};
t814 = ct{664};
t815 = ct{665};
t817 = ct{666};
t821 = ct{667};
t822 = ct{668};
t824 = ct{669};
t825 = ct{670};
t826 = ct{671};
t827 = ct{672};
t828 = ct{673};
t836 = ct{674};
t841 = ct{675};
t842 = ct{676};
t844 = ct{677};
t848 = ct{678};
t850 = ct{679};
t854 = ct{680};
t855 = ct{681};
t856 = ct{682};
t858 = ct{683};
t86 = ct{684};
t864 = ct{685};
t865 = ct{686};
t866 = ct{687};
t87 = ct{688};
t872 = ct{689};
t873 = ct{690};
t874 = ct{691};
t878 = ct{692};
t88 = ct{693};
t880 = ct{694};
t881 = ct{695};
t889 = ct{696};
t89 = ct{697};
t890 = ct{698};
t893 = ct{699};
t896 = ct{700};
t899 = ct{701};
t9 = ct{702};
t90 = ct{703};
t901 = ct{704};
t902 = ct{705};
t907 = ct{706};
t909 = ct{707};
t91 = ct{708};
t910 = ct{709};
t912 = ct{710};
t914 = ct{711};
t915 = ct{712};
t916 = ct{713};
t92 = ct{714};
t920 = ct{715};
t921 = ct{716};
t924 = ct{717};
t929 = ct{718};
t93 = ct{719};
t930 = ct{720};
t931 = ct{721};
t933 = ct{722};
t938 = ct{723};
t939 = ct{724};
t94 = ct{725};
t941 = ct{726};
t942 = ct{727};
t944 = ct{728};
t950 = ct{729};
t952 = ct{730};
t953 = ct{731};
t955 = ct{732};
t96 = ct{733};
t962 = ct{734};
t963 = ct{735};
t964 = ct{736};
t966 = ct{737};
t967 = ct{738};
t969 = ct{739};
t97 = ct{740};
t977 = ct{741};
t979 = ct{742};
t98 = ct{743};
t980 = ct{744};
t981 = ct{745};
t985 = ct{746};
t986 = ct{747};
t987 = ct{748};
t988 = ct{749};
t989 = ct{750};
t990 = ct{751};
t992 = ct{752};
t994 = ct{753};
t996 = ct{754};
t997 = ct{755};
t998 = ct{756};
t999 = ct{757};
t1725 = t1395.*2.9e-4;
t1729 = t1395.*2.900000000000001e-4;
t1732 = t655.*(t485+t7.*(t53-t132)).*(-2.32e-3);
t1735 = t1395.*(-2.94e-3);
t1744 = t1395.*2.94e-3;
t1749 = t1412.*2.9e-4;
t1754 = t1412.*2.900000000000001e-4;
t1758 = t675.*(t8.*(t57-t165)+t15.*(t136-t246)).*(-2.9e-4);
t1760 = t1412.*2.94e-3;
t1763 = t675.*(t8.*(t57-t165)+t15.*(t136-t246)).*(-2.900000000000001e-4);
t1767 = t675.*(t8.*(t57-t165)+t15.*(t136-t246)).*(-2.94e-3);
t1803 = t564+t613+t697+t735;
t1804 = t566+t590+t733+t753;
t1987 = t757+t771+t801+t827+t828;
t1988 = t87+t172+t715+t719+t737+t758+t782;
t1997 = t88+t559+t678+t699+t712+t799+t821;
t1998 = t1625.*t1697.*(3.41e+2./1.0e+2);
t2010 = t1699.*t1731.*2.61155;
t2018 = t1697.*t1782.*(3.41e+2./1.0e+2);
t2024 = -t2022;
t2028 = t1731.*t1810.*2.61155;
t2037 = t1783.*t1805.*(3.41e+2./1.0e+2);
t2046 = t1697.*t1919.*(3.41e+2./1.0e+2);
t2052 = t1776.*t1885.*(3.41e+2./1.0e+2);
t2053 = t1783.*t1883.*(3.41e+2./1.0e+2);
t2061 = t1731.*t1949.*2.61155;
t2062 = t1707.*t1960.*2.61155;
t2064 = t1805.*t1883.*(3.41e+2./1.0e+2);
t2066 = t1715.*t1960.*2.61155;
t2070 = (t313.*t2042)./2.0;
t2073 = -t2071;
t2077 = -t2076;
t2079 = (t470.*t2042)./2.0;
t2080 = t1783.*t1954.*(3.41e+2./1.0e+2);
t2083 = t1802.*t1935.*3.38795;
t2089 = -t2086;
t2093 = -t2092;
t2097 = t1808.*t1960.*2.61155;
t2101 = -t2099;
t2103 = t1783.*t1983.*(3.41e+2./1.0e+2);
t2106 = -t2105;
t2109 = -t2108;
t2110 = t1883.*t1954.*(3.41e+2./1.0e+2);
t2112 = t1885.*t1953.*(3.41e+2./1.0e+2);
t2114 = (t470.*t2081)./2.0;
t2115 = t1805.*t1983.*(3.41e+2./1.0e+2);
t2118 = -t2116;
t2119 = t921+t1053+t1084+t1085+t1225+t1246;
t2122 = t967+t1037+t1114+t1115+t1215+t1234;
t2127 = t1802.*t1993.*3.38795;
t2128 = t1883.*t1983.*(3.41e+2./1.0e+2);
t2131 = t1935.*t1965.*3.38795;
t2133 = t1049+t1063+t1170+t1173+t1220+t1242;
t2135 = t1885.*t1985.*(3.41e+2./1.0e+2);
t2138 = t1954.*t1983.*(3.41e+2./1.0e+2);
t2143 = t1930.*(-t87-t172+t277.*4.9e-4+t711+t727+t770+t13.*(t53-t132).*2.75e-2).*(-3.38795);
t2145 = t1930.*(-t87-t172+t277.*4.9e-4+t711+t727+t770+t13.*(t53-t132).*2.75e-2).*3.38795;
t2147 = t1935.*t1993.*3.38795;
t2160 = t1965.*t1993.*3.38795;
t2194 = t500.*(t342.*3.844e-2-t1194+t1222+t1250-t1292+t1324).*(-1.0./2.0);
t2198 = (t314.*t2184)./2.0;
t2199 = t773.*(t342.*1.12e-3-t1168+t1213+t1232-t1337+t1365).*(-1.0./2.0);
t2202 = (t773.*(t342.*1.12e-3-t1168+t1213+t1232-t1337+t1365))./2.0;
t2203 = (t346.*t2183)./2.0;
t2208 = -t2207;
t2211 = (t455.*t2184)./2.0;
t2212 = t914.*(t342.*3.844e-2-t1194+t1222+t1250-t1292+t1324).*(-1.0./2.0);
t2223 = (t654.*t2183)./2.0;
t2226 = t1097.*(t342.*3.844e-2-t1194+t1222+t1250-t1292+t1324).*(-1.0./2.0);
t2230 = t2036.*(t533.*2.324e-2+t788+t8.*(t57-t165).*3.466000000000001e-2+t15.*(t136-t246).*3.466000000000001e-2).*(-3.5432e-1);
t2231 = t2036.*(t533.*2.324e-2+t788+t8.*(t57-t165).*3.466000000000001e-2+t15.*(t136-t246).*3.466000000000001e-2).*3.5432e-1;
t2232 = ((t180-t333+t5.*t121.*(t53-t132)).*(t342.*1.12e-3-t1168+t1213+t1232-t1337+t1365))./2.0;
t2237 = ((-t231+t397+t170.*(t53-t132)).*(t342.*1.12e-3-t1168+t1213+t1232-t1337+t1365))./2.0;
t2269 = t907+t985+t1014+t1045+t1051+t1193+t1230+t1249+t1251;
t2272 = t916+t994+t1003+t1027+t1088+t1192+t1209+t1238+t1274;
t2273 = t915+t997+t1000+t1024+t1092+t1167+t1214+t1268+t1285;
t2311 = t500.*(t308.*8.8e-4-t1020+t1034-t1094-t1124+t1131+t1140+t1255+t170.*(t53-t132).*1.12e-3).*(-1.0./2.0);
t2330 = t773.*(t308.*1.11e-3+t977-t1033+t1095-t1136-t1155+t1159+t1300+t170.*(t53-t132).*4.988e-2).*(-1.0./2.0);
t2331 = (t773.*(t308.*1.11e-3+t977-t1033+t1095-t1136-t1155+t1159+t1300+t170.*(t53-t132).*4.988e-2))./2.0;
t2333 = t902.*(t308.*8.8e-4-t1020+t1034-t1094-t1124+t1131+t1140+t1255+t170.*(t53-t132).*1.12e-3).*(-1.0./2.0);
t2334 = (t902.*(t308.*8.8e-4-t1020+t1034-t1094-t1124+t1131+t1140+t1255+t170.*(t53-t132).*1.12e-3))./2.0;
t2336 = ((t312+t121.*(t51-t155)).*(t308.*1.144e-2-t1039-t1066+t1080-t1125+t1151+t1182+t1229+t170.*(t53-t132).*1.11e-3))./2.0;
t2341 = t1097.*(t308.*8.8e-4-t1020+t1034-t1094-t1124+t1131+t1140+t1255+t170.*(t53-t132).*1.12e-3).*(-1.0./2.0);
t2344 = ((t191-t311+t122.*(t51-t155)).*(t308.*1.144e-2-t1039-t1066+t1080-t1125+t1151+t1182+t1229+t170.*(t53-t132).*1.11e-3))./2.0;
t2347 = ((t180-t333+t5.*t121.*(t53-t132)).*(t308.*1.11e-3+t977-t1033+t1095-t1136-t1155+t1159+t1300+t170.*(t53-t132).*4.988e-2))./2.0;
t2348 = t1149.*(t308.*1.11e-3+t977-t1033+t1095-t1136-t1155+t1159+t1300+t170.*(t53-t132).*4.988e-2).*(-1.0./2.0);
t519 = t15.*t463;
t650 = t8.*t591;
t653 = t15.*t591;
t658 = t8.*t596;
t659 = t15.*t596;
t673 = t192+t340;
t693 = t267+t289;
t694 = t220+t336;
t721 = -t8.*(t198-t336);
t724 = -t15.*(t198-t336);
t750 = t15.*(t198-t336);
t775 = -t765;
t851 = t244+t516;
t861 = t8.*t836;
t862 = t15.*t836;
t868 = t336.*4.9e-4;
t876 = t340.*2.019e-2;
t879 = -t864;
t888 = t242+t530;
t891 = t8.*t856;
t892 = -t872;
t894 = t15.*t856;
t905 = -t890;
t906 = t15.*t881;
t923 = t340.*1.9738e-1;
t949 = -t942;
t970 = -t953;
t984 = -t964;
t1061 = -t1047;
t1075 = t261+t720;
t1089 = t278+t723;
t1122 = -t1116;
t1141 = -t1120;
t1145 = -t13.*t836.*(t53-t132);
t1147 = -t1134;
t1161 = t13.*t228.*t856;
t1165 = t8.*(t198-t336).*(-3.466000000000001e-2);
t1174 = t8.*(t198-t336).*3.466000000000001e-2;
t1188 = -t671.*(t129+t13.*(t51-t155));
t1189 = -t836.*(t72-t217);
t1190 = -t1179;
t1202 = t836.*(t72-t217);
t1206 = -t1197;
t1207 = -t1198;
t1212 = -t856.*(t66-t210);
t1224 = t300.*t836;
t1227 = -t1219;
t1228 = -t1203;
t1241 = t463.*4.000000000000028e-5;
t1244 = t463.*3.0e-5;
t1245 = t301.*t856;
t1265 = t463.*2.32e-3;
t1288 = t395.*t836;
t1298 = -t1278;
t1304 = -t1293;
t1308 = -t836.*(t156-t236);
t1319 = t451.*t856;
t1320 = -t856.*(t156-t236);
t1321 = -t836.*(t129+t13.*(t51-t155));
t1329 = -t856.*(t129+t13.*(t51-t155));
t1334 = t836.*(t129+t13.*(t51-t155));
t1347 = -t1333;
t1363 = -t1349;
t1380 = -t1374;
t1384 = -t596.*(t485+t7.*(t53-t132));
t1394 = t596.*(t485+t7.*(t53-t132));
t1415 = -t1407;
t1421 = (t485+t7.*(t53-t132)).*(t198-t336);
t1422 = t841.*(-4.000000000000028e-5);
t1423 = t815.*3.0e-5;
t1425 = t841.*(-3.0e-5);
t1432 = t815.*4.000000000000028e-5;
t1435 = t841.*4.000000000000028e-5;
t1436 = t841.*3.0e-5;
t1437 = -t1429;
t1452 = -t1442;
t1462 = t815.*2.32e-3;
t1464 = t841.*(-2.32e-3);
t1468 = -t1459;
t1469 = -t1460;
t1472 = t881.*4.000000000000028e-5;
t1473 = t881.*3.0e-5;
t1474 = t890.*4.000000000000028e-5;
t1475 = t890.*3.0e-5;
t1486 = t890.*2.32e-3;
t1489 = t881.*2.32e-3;
t1500 = -t1495;
t1502 = -t1499;
t1509 = -t856.*(t485+t7.*(t53-t132));
t1512 = -t1507;
t1514 = t856.*(t485+t7.*(t53-t132));
t1525 = t1133.*(-3.0e-5);
t1526 = t344+t706+t708;
t1527 = t1133.*3.0e-5;
t1530 = t1133.*(-5.0e-5);
t1534 = t1133.*5.0e-5;
t1535 = t13.*t836.*(t53-t132).*(-4.000000000000028e-5);
t1537 = t1133.*(-5.000000000000004e-4);
t1538 = t13.*t836.*(t53-t132).*4.000000000000028e-5;
t1540 = t13.*t836.*(t53-t132).*(-5.0e-5);
t1541 = t1108.*2.2e-4;
t1543 = -t1060.*(t485+t7.*(t53-t132));
t1544 = t1108.*2.900000000000001e-4;
t1545 = t1133.*5.000000000000004e-4;
t1546 = t1120.*2.2e-4;
t1550 = t1120.*2.900000000000001e-4;
t1553 = t13.*t836.*(t53-t132).*(-2.81e-3);
t1554 = t1108.*7.950000000000001e-3;
t1560 = t1120.*7.950000000000001e-3;
t1571 = t671.*(t129+t13.*(t51-t155)).*(-3.0e-5);
t1574 = t671.*(t129+t13.*(t51-t155)).*(-5.0e-5);
t1577 = t856.*(t66-t210).*(-4.000000000000028e-5);
t1582 = t856.*(t66-t210).*4.000000000000028e-5;
t1584 = t1179.*2.2e-4;
t1585 = -t1105.*(t485+t7.*(t53-t132));
t1589 = t1179.*2.900000000000001e-4;
t1591 = t856.*(t66-t210).*(-5.0e-5);
t1592 = t671.*(t129+t13.*(t51-t155)).*(-5.000000000000004e-4);
t1595 = t1179.*7.950000000000001e-3;
t1600 = t856.*(t66-t210).*(-2.81e-3);
t1604 = t1203.*1.089e-2;
t1605 = t1203.*2.9e-4;
t1607 = t1203.*2.2e-4;
t1615 = t1226.*1.089e-2;
t1616 = t1226.*2.9e-4;
t1620 = t1226.*2.2e-4;
t1628 = t836.*(t156-t236).*(-3.0e-5);
t1630 = t836.*(t156-t236).*3.0e-5;
t1632 = t1278.*1.089e-2;
t1633 = t1278.*2.9e-4;
t1636 = t856.*(t156-t236).*(-4.000000000000028e-5);
t1637 = t1278.*2.2e-4;
t1640 = t836.*(t156-t236).*(-5.0e-5);
t1643 = t1330.*4.000000000000028e-5;
t1644 = t856.*(t129+t13.*(t51-t155)).*(-3.0e-5);
t1645 = t1330.*3.0e-5;
t1646 = t836.*(t156-t236).*(-5.000000000000004e-4);
t1649 = t1333.*3.0e-5;
t1650 = t856.*(t156-t236).*(-5.0e-5);
t1653 = t1306.*2.900000000000001e-4;
t1654 = t856.*(t129+t13.*(t51-t155)).*3.0e-5;
t1655 = t836.*(t156-t236).*5.000000000000004e-4;
t1657 = t856.*(t156-t236).*5.0e-5;
t1659 = t1306.*2.2e-4;
t1661 = t856.*(t156-t236).*(-2.81e-3);
t1663 = t856.*(t129+t13.*(t51-t155)).*(-5.0e-5);
t1665 = t1333.*5.0e-5;
t1669 = t1306.*7.950000000000001e-3;
t1673 = t856.*(t129+t13.*(t51-t155)).*(-5.000000000000004e-4);
t1675 = t1333.*5.000000000000004e-4;
t1676 = t1330.*2.32e-3;
t1679 = t856.*(t129+t13.*(t51-t155)).*5.000000000000004e-4;
t1680 = t1346.*(-2.900000000000001e-4);
t1684 = t1346.*(-2.9e-4);
t1685 = t1346.*2.900000000000001e-4;
t1686 = t1346.*2.9e-4;
t1688 = t1349.*2.2e-4;
t1692 = t1349.*1.089e-2;
t1693 = t1349.*2.9e-4;
t1694 = t1346.*(-2.94e-3);
t1703 = t1346.*2.94e-3;
t1769 = t462+t920+t939;
t1806 = t1060.*(t485+t7.*(t53-t132)).*(-2.2e-4);
t1807 = t1060.*(t485+t7.*(t53-t132)).*(-2.900000000000001e-4);
t1809 = t1060.*(t485+t7.*(t53-t132)).*(-7.950000000000001e-3);
t1819 = t1105.*(t485+t7.*(t53-t132)).*(-2.900000000000001e-4);
t1823 = t1105.*(t485+t7.*(t53-t132)).*(-2.2e-4);
t1824 = t1105.*(t485+t7.*(t53-t132)).*2.900000000000001e-4;
t1827 = t1105.*(t485+t7.*(t53-t132)).*2.2e-4;
t1828 = t1105.*(t485+t7.*(t53-t132)).*(-7.950000000000001e-3);
t1829 = t1105.*(t485+t7.*(t53-t132)).*7.950000000000001e-3;
t1891 = t824+t1133+t1139;
t1952 = t741+t756+t931+t941;
t1964 = t740+t752+t955+t963;
t1968 = t785+t802+t989+t999;
t2000 = t90+t94+t114+t477+t644+t651+t660+t803+t825;
t2001 = t86+t92+t113+t496+t643+t645+t665+t800+t817;
t2003 = t794+t1017+t1290+t1299;
t2007 = t61+t96+t627+t637+t680+t695+t874+t878;
t2011 = -t2010;
t2019 = t952+t962+t1010+t1057+t1062;
t2027 = t987+t1009+t1059+t1070+t1076;
t2029 = -t2028;
t2030 = t1776.*t1803.*(3.41e+2./1.0e+2);
t2039 = -t2037;
t2044 = t1802.*t1804.*3.38795;
t2047 = -t2046;
t2054 = -t2052;
t2055 = -t2053;
t2060 = t1803.*t1885.*(3.41e+2./1.0e+2);
t2063 = -t2061;
t2072 = t112+t205+t783+t786+t812+t814+t1164+t1180;
t2074 = t174+t679+t880+t893+t924+t1153+t1154;
t2087 = t1804.*t1935.*3.38795;
t2090 = t1803.*t1953.*(3.41e+2./1.0e+2);
t2098 = -t2097;
t2100 = t1804.*t1965.*3.38795;
t2104 = -t2103;
t2111 = -t2110;
t2117 = t1803.*t1985.*(3.41e+2./1.0e+2);
t2129 = -t2127;
t2134 = t1804.*t1993.*3.38795;
t2139 = -t2138;
t2140 = (t500.*t2122)./2.0;
t2148 = -t2147;
t2150 = t2119.*(t312+t121.*(t51-t155)).*(-1.0./2.0);
t2151 = t1945.*(t112+t205+t717+t765-t769+t7.*(t51-t155).*2.019e-2+t14.*(t51-t155).*4.9e-4).*(-3.38795);
t2152 = (t933.*t2119)./2.0;
t2153 = t1987.*(t533.*2.324e-2+t788+t8.*(t57-t165).*3.466000000000001e-2+t15.*(t136-t246).*3.466000000000001e-2).*(-3.5432e-1);
t2154 = (t902.*t2122)./2.0;
t2155 = (t914.*t2122)./2.0;
t2159 = t1194+t1200+t1235+t1252+t1292+t1328;
t2161 = -t2160;
t2162 = t1217+t1239+t1247+t1263+t1286+t1305;
t2163 = t2119.*(t191-t311+t122.*(t51-t155)).*(-1.0./2.0);
t2164 = (t2119.*(t191-t311+t122.*(t51-t155)))./2.0;
t2165 = t1168+t1211+t1223+t1243+t1337+t1369;
t2175 = t1074+t1195+t1248+t1253+t1434+t1449;
t2181 = t1997.*(t533.*2.324e-2+t788+t8.*(t57-t165).*3.466000000000001e-2+t15.*(t136-t246).*3.466000000000001e-2).*(-3.5432e-1);
t2182 = t1997.*(t533.*2.324e-2+t788+t8.*(t57-t165).*3.466000000000001e-2+t15.*(t136-t246).*3.466000000000001e-2).*3.5432e-1;
t2185 = t2133.*(t180-t333+t5.*t121.*(t53-t132)).*(-1.0./2.0);
t2186 = (t1149.*t2133)./2.0;
t2187 = (t2133.*(t180-t333+t5.*t121.*(t53-t132)))./2.0;
t2189 = t1162+t1163+t1322+t1335+t1393+t1411;
t2192 = t2133.*(-t231+t397+t170.*(t53-t132)).*(-1.0./2.0);
t2193 = (t2133.*(-t231+t397+t170.*(t53-t132)))./2.0;
t2196 = t1987.*t1997.*3.5432e-1;
t2201 = -t2198;
t2204 = t1945.*(-t98+t173+t580-t703-t930+t942-t9.*t10.*(2.1e+1./5.0e+1)+t7.*(t53-t132).*2.019e-2+t14.*(t53-t132).*4.9e-4).*(-3.38795);
t2214 = t1999.*(t112+t205+t717+t765-t769+t7.*(t51-t155).*2.019e-2+t14.*(t51-t155).*4.9e-4).*(-3.38795);
t2245 = t1987.*t2036.*3.5432e-1;
et1 = t112+t205+t717+t765-t769+t7.*(t51-t155).*2.019e-2+t14.*(t51-t155).*4.9e-4;
et2 = (-t98+t173+t580-t703-t930+t942-t9.*t10.*(2.1e+1./5.0e+1)+t7.*(t53-t132).*2.019e-2+t14.*(t53-t132).*4.9e-4).*3.38795;
t2249 = et1.*et2;
t2251 = t1269+t1291+t1405+t1420+t1528+t1531;
t2254 = t1439+t1448+t1454+t1463+t1471+t1480;
t2258 = t1999.*(-t98+t173+t580-t703-t930+t942-t9.*t10.*(2.1e+1./5.0e+1)+t7.*(t53-t132).*2.019e-2+t14.*(t53-t132).*4.9e-4).*(-3.38795);
t2263 = t1997.*t2036.*3.5432e-1;
t2267 = t1428+t1453+t1457+t1467+t1516+t1517;
t2275 = t1020+t1050+t1094+t1124+t1142+t1150+t1169+t1259+t1261;
t2279 = t1039+t1066+t1087+t1125+t1160+t1185+t1208+t1233+t1240;
t2282 = t996+t1033+t1101+t1128+t1136+t1155+t1166+t1303+t1311;
t2307 = (t773.*t2273)./2.0;
t2312 = (t902.*t2269)./2.0;
t2315 = (t914.*t2269)./2.0;
t2316 = t1341.*(-t1269+t1284+t1417+t1529+t228.*(t156-t236).*9.999999999999998e-6+t451.*(t156-t236).*1.2e-4).*(-1.0./2.0);
t2317 = t2272.*(t312+t121.*(t51-t155)).*(-1.0./2.0);
t2318 = (t2272.*(t312+t121.*(t51-t155)))./2.0;
t2319 = (t933.*t2272)./2.0;
t2323 = (t1097.*t2269)./2.0;
t2332 = (t1149.*t2273)./2.0;
t2335 = t912+t992+t1072+t1073+t1254+t1260+t1302+t1484+t1491;
t2337 = -t2336;
t2340 = t2273.*(-t231+t397+t170.*(t53-t132)).*(-1.0./2.0);
t2356 = t1658.*(-t1269+t1284+t1417+t1529+t228.*(t156-t236).*9.999999999999998e-6+t451.*(t156-t236).*1.2e-4).*(-1.0./2.0);
t2364 = t1757.*(-t1269+t1284+t1417+t1529+t228.*(t156-t236).*9.999999999999998e-6+t451.*(t156-t236).*1.2e-4).*(-1.0./2.0);
t2377 = t1043+t1135+t1184+t1373+t1376+t1390+t1400+t1408+t1409;
t2379 = t1130+t1137+t1218+t1370+t1371+t1377+t1379+t1485+t1492;
t2410 = t1341.*(t896-t1090+t1197+t1198+t1272-t1338-t1523+t300.*(t53-t132).*9.999999999999998e-6+t315.*(t156-t236).*1.2e-4).*(-1.0./2.0);
t2411 = ((t822+t228.*(t156-t236)).*(t969+t1116+t1117+t1183-t1204-t1414-t1419+t451.*(t51-t155).*1.0e-5+t6.*t228.*(t129+t13.*(t51-t155)).*9.999999999999998e-6))./2.0;
t2419 = t1504.*(t969+t1116+t1117+t1183-t1204-t1414-t1419+t451.*(t51-t155).*1.0e-5+t6.*t228.*(t129+t13.*(t51-t155)).*9.999999999999998e-6).*(-1.0./2.0);
t2421 = t1505.*(t969+t1116+t1117+t1183-t1204-t1414-t1419+t451.*(t51-t155).*1.0e-5+t6.*t228.*(t129+t13.*(t51-t155)).*9.999999999999998e-6).*(-1.0./2.0);
t2431 = ((t328-t795+t395.*(t53-t132)).*(t969+t1116+t1117+t1183-t1204-t1414-t1419+t451.*(t51-t155).*1.0e-5+t6.*t228.*(t129+t13.*(t51-t155)).*9.999999999999998e-6))./2.0;
t2439 = t1627.*(t896-t1090+t1197+t1198+t1272-t1338-t1523+t300.*(t53-t132).*9.999999999999998e-6+t315.*(t156-t236).*1.2e-4).*(-1.0./2.0);
t2441 = t1658.*(t896-t1090+t1197+t1198+t1272-t1338-t1523+t300.*(t53-t132).*9.999999999999998e-6+t315.*(t156-t236).*1.2e-4).*(-1.0./2.0);
t2451 = t1757.*(t896-t1090+t1197+t1198+t1272-t1338-t1523+t300.*(t53-t132).*9.999999999999998e-6+t315.*(t156-t236).*1.2e-4).*(-1.0./2.0);
t677 = -t659;
t882 = -t868;
t898 = t888.^2;
t1065 = t309+t658;
t1068 = t305+t650;
t1083 = t318+t653;
t1096 = t650.*3.466000000000001e-2;
t1099 = t658.*3.466000000000001e-2;
t1100 = t653.*2.324e-2;
t1102 = t659.*2.324e-2;
t1157 = t322+t721;
t1172 = t750.*(-2.324e-2);
t1175 = t319+t750;
t1178 = -t673.*(t156-t236);
t1266 = t861.*3.466000000000001e-2;
t1267 = t862.*3.466000000000001e-2;
t1277 = t861.*2.324e-2;
t1279 = t862.*2.324e-2;
t1280 = t894.*3.466000000000001e-2;
t1282 = t519.*2.2e-4;
t1287 = t519.*2.900000000000001e-4;
t1289 = t891.*3.466000000000001e-2;
t1296 = t891.*2.324e-2;
t1297 = t894.*2.324e-2;
t1307 = t519.*7.950000000000001e-3;
t1310 = t8.*t888.*3.466000000000001e-2;
t1313 = t15.*t888.*2.324e-2;
t1332 = -t888.*(t156-t236);
t1344 = t513+t862;
t1359 = t534+t861;
t1360 = -t7.*t888.*(t129+t13.*(t51-t155));
t1368 = t528+t894;
t1383 = t552+t891;
t1399 = t591.*t888;
t1433 = -t888.*(t153+t7.*(t143-t164));
t1451 = -t888.*(t273+t14.*(t51-t155));
t1478 = -t1475;
t1490 = -t1486;
t1496 = t906.*2.2e-4;
t1498 = t906.*2.900000000000001e-4;
t1508 = t836.*t888;
t1510 = t906.*7.950000000000001e-3;
t1542 = t1161.*4.000000000000028e-5;
t1548 = -t1541;
t1551 = -t1544;
t1552 = t1161.*5.0e-5;
t1555 = -t1546;
t1556 = -t1550;
t1559 = t673.*(t156-t236).*(-3.0e-5);
t1561 = -t1554;
t1562 = (t485+t7.*(t53-t132)).*(t659+t8.*(t72-t217));
t1564 = t673.*(t156-t236).*3.0e-5;
t1565 = -t1560;
t1567 = t673.*(t156-t236).*(-5.0e-5);
t1570 = t1202.*(-4.000000000000028e-5);
t1572 = t1161.*2.81e-3;
t1575 = t1202.*(-5.0e-5);
t1578 = -t888.*(t257+t15.*(t273+t14.*(t51-t155)));
t1580 = t673.*(t156-t236).*(-5.000000000000004e-4);
t1581 = t1202.*5.0e-5;
t1583 = t1224.*4.000000000000028e-5;
t1588 = t673.*(t156-t236).*5.000000000000004e-4;
t1593 = t1202.*(-2.81e-3);
t1596 = t1245.*4.000000000000028e-5;
t1597 = t1224.*5.0e-5;
t1598 = t1202.*2.81e-3;
t1606 = t1224.*2.81e-3;
t1608 = t1245.*5.0e-5;
t1609 = -t1604;
t1610 = -t1605;
t1612 = -t1607;
t1613 = t888.*t1156;
t1618 = t888.*t1148;
t1621 = t1245.*2.81e-3;
t1624 = t1288.*4.000000000000028e-5;
t1629 = t1288.*5.0e-5;
t1634 = t1319.*4.000000000000028e-5;
t1638 = t1334.*(-4.000000000000028e-5);
t1639 = t1288.*2.81e-3;
t1641 = t1334.*4.000000000000028e-5;
t1647 = t888.*(t156-t236).*(-3.0e-5);
t1648 = t1319.*5.0e-5;
t1651 = t1334.*(-5.0e-5);
t1656 = t888.*(t156-t236).*3.0e-5;
t1660 = t1319.*2.81e-3;
t1662 = t1334.*(-2.81e-3);
t1664 = t888.*(t156-t236).*(-5.0e-5);
t1668 = t1334.*2.81e-3;
t1670 = -t1665;
t1672 = t7.*t888.*(t129+t13.*(t51-t155)).*(-3.0e-5);
t1674 = t888.*(t156-t236).*(-5.000000000000004e-4);
t1677 = t7.*t888.*(t129+t13.*(t51-t155)).*(-4.000000000000028e-5);
t1681 = t888.*(t156-t236).*5.000000000000004e-4;
t1683 = -t1676;
t1696 = -t1688;
t1698 = t7.*t888.*(t129+t13.*(t51-t155)).*(-2.32e-3);
t1700 = t1394.*(-4.000000000000028e-5);
t1701 = -t1692;
t1702 = -t1693;
t1704 = t1394.*(-3.0e-5);
t1705 = t7.*t888.*(t129+t13.*(t51-t155)).*2.32e-3;
t1706 = t1394.*3.0e-5;
t1718 = t1394.*(-2.32e-3);
t1721 = t1394.*2.32e-3;
t1734 = t888.*(t153+t7.*(t143-t164)).*(-4.000000000000028e-5);
t1736 = t1421.*4.000000000000028e-5;
t1737 = t888.*(t153+t7.*(t143-t164)).*(-3.0e-5);
t1739 = t1421.*3.0e-5;
t1747 = t888.*(t273+t14.*(t51-t155)).*(-4.000000000000028e-5);
t1748 = t888.*(t273+t14.*(t51-t155)).*(-3.0e-5);
t1751 = t888.*(t273+t14.*(t51-t155)).*4.000000000000028e-5;
t1755 = t1421.*2.32e-3;
t1756 = t888.*(t153+t7.*(t143-t164)).*(-2.32e-3);
t1764 = t888.*(t273+t14.*(t51-t155)).*(-2.32e-3);
t1773 = t1514.*(-4.000000000000028e-5);
t1775 = t1514.*(-3.0e-5);
t1778 = t1514.*4.000000000000028e-5;
t1779 = t1514.*3.0e-5;
t1788 = t1514.*(-2.32e-3);
t1791 = t1514.*2.32e-3;
t1816 = t888.*(t257+t15.*(t273+t14.*(t51-t155))).*(-2.900000000000001e-4);
t1817 = t888.*(t257+t15.*(t273+t14.*(t51-t155))).*(-2.2e-4);
t1825 = t888.*(t257+t15.*(t273+t14.*(t51-t155))).*(-7.950000000000001e-3);
t1826 = t1320+t1334;
t1884 = t710+t1145+t1161;
t1887 = t726+t1144+t1188;
t1928 = t780+t1202+t1212;
t1929 = t748+t1224+t1245;
t1961 = t674+t792+t950+t984;
t1967 = t798+t1288+t1319;
t1971 = t826+t1308+t1329;
t1994 = t97+t221+t734+t759+t769+t772+t775;
t2026 = t91+t98+t202+t599+t703+t732+t751+t930+t949;
t2031 = -t2030;
t2033 = t89+t93+t207+t554+t742+t761+t763+t966+t970;
t2045 = -t2044;
t2057 = t87+t172+t777+t784+t787+t813+t1121+t1147;
t2091 = -t2087;
t2102 = -t2100;
t2123 = t1930.*t1952.*3.38795;
t2130 = t1945.*t1964.*3.38795;
t2141 = -t2140;
t2144 = t866+t1091+t1103+t1191+t1438+t1452;
t2149 = t1952.*(-t87-t172+t277.*4.9e-4+t711+t727+t770+t13.*(t53-t132).*2.75e-2).*(-3.38795);
t2156 = -t2155;
t2157 = t1964.*(t112+t205+t717+t765-t769+t7.*(t51-t155).*2.019e-2+t14.*(t51-t155).*4.9e-4).*(-3.38795);
t2158 = t1964.*(t112+t205+t717+t765-t769+t7.*(t51-t155).*2.019e-2+t14.*(t51-t155).*4.9e-4).*3.38795;
t2166 = t1930.*t2000.*3.38795;
M = ft_4({q1,q2,t10,t1006,t1011,t1012,t1018,t1020,t1026,t1029,t1031,t1033,t1034,t1039,t1042,t1046,t1056,t1058,t1060,t1061,t1065,t1066,t1068,t1075,t1079,t1080,t1083,t1090,t1093,t1094,t1095,t1096,t1097,t1098,t1099,t1100,t1102,t1105,t1107,t1108,t1110,t1111,t1112,t1116,t1117,t1119,t112,t1120,t1122,t1123,t1124,t1125,t1126,t1127,t1129,t113,t1131,t1132,t1136,t1138,t114,t1140,t1141,t1143,t1146,t1149,t1151,t1155,t1157,t1159,t1168,t1172,t1174,t1175,t1176,t1177,t1178,t1179,t1181,t1182,t1183,t1186,t1189,t119,t1190,t1194,t1196,t1197,t1198,t120,t1203,t1204,t1205,t1206,t1207,t121,t1213,t122,t1222,t1226,t1227,t1228,t1229,t1232,t1241,t1244,t1250,t1255,t1257,t1262,t1264,t1265,t1266,t1267,t1269,t1270,t1272,t1275,t1276,t1277,t1279,t1280,t1282,t1283,t1284,t1287,t1289,t129,t1292,t1293,t1295,t1296,t1297,t1298,t13,t130,t1300,t1301,t1304,t1306,t1307,t1310,t1312,t1313,t1315,t1317,t1318,t132,t1323,t1324,t1325,t1326,t1327,t1330,t1332,t1333,t1336,t1337,t1338,t1339,t1340,t1341,t1342,t1343,t1344,t1345,t1346,t1347,t1348,t1351,t1353,t1355,t1356,t1357,t1358,t1359,t136,t1360,t1362,t1363,t1364,t1365,t1366,t1367,t1368,t1372,t1375,t1380,t1381,t1383,t1387,t1389,t1391,t1394,t1395,t1396,t1397,t1398,t1399,t14,t1402,t1403,t1404,t1406,t1410,t1412,t1413,t1414,t1415,t1416,t1417,t1418,t1419,t1421,t1423,t1424,t1425,t1426,t1427,t143,t1431,t1432,t1433,t1435,t1436,t1437,t1441,t1446,t1447,t1451,t1455,t1458,t1461,t1462,t1464,t1465,t1466,t1468,t1469,t1470,t1472,t1473,t1474,t1475,t1478,t1486,t1488,t1489,t1490,t1495,t1496,t1497,t1498,t1499,t15,t1500,t1501,t1502,t1503,t1504,t1505,t1507,t1508,t1510,t1512,t1514,t1518,t1519,t1520,t1521,t1522,t1523,t1524,t1526,t1527,t1529,t153,t1530,t1532,t1533,t1534,t1535,t1536,t1537,t1538,t1539,t1540,t1542,t1543,t1545,t1546,t1547,t1548,t155,t1550,t1551,t1552,t1553,t1555,t1556,t1558,t156,t1560,t1561,t1562,t1563,t1564,t1565,t1566,t1567,t1568,t1569,t1570,t1571,t1572,t1574,t1575,t1578,t1581,t1582,t1583,t1584,t1585,t1587,t1588,t1589,t1591,t1592,t1593,t1595,t1596,t1597,t1598,t16,t1600,t1601,t1603,t1604,t1605,t1606,t1607,t1608,t1609,t1610,t1612,t1613,t1615,t1616,t1618,t1620,t1621,t1624,t1625,t1627,t1629,t1630,t1632,t1633,t1634,t1636,t1637,t1639,t164,t1640,t1641,t1643,t1645,t1648,t1649,t165,t1651,t1653,t1654,t1655,t1656,t1657,t1658,t1659,t1660,t1661,t1662,t1663,t1664,t1665,t1668,t1669,t167,t1670,t1671,t1672,t1675,t1677,t1678,t1679,t1681,t1682,t1683,t1685,t1686,t1687,t1689,t1690,t1691,t1695,t1696,t1697,t1699,t17,t170,t1700,t1701,t1702,t1703,t1704,t1705,t1706,t1707,t1715,t1717,t172,t1720,t1721,t1725,t1729,t173,t1731,t1732,t1734,t1736,t1737,t1739,t1744,t1748,t1749,t1751,t1754,t1755,t1756,t1757,t1758,t1760,t1763,t1764,t1767,t1769,t1771,t1773,t1776,t1777,t1778,t1779,t1782,t1783,t1784,t1785,t1789,t1791,t1794,t1795,t1797,t1798,t18,t180,t1802,t1803,t1804,t1805,t1806,t1807,t1808,t1809,t1810,t1816,t1817,t1819,t1823,t1824,t1825,t1826,t1827,t1828,t1829,t1867,t1883,t1884,t1885,t191,t1919,t1929,t1930,t1935,t1945,t1949,t1952,t1953,t1954,t1960,t1961,t1964,t1965,t1967,t1969,t1970,t1972,t1983,t1985,t1987,t1991,t1992,t1993,t1996,t1997,t1998,t1999,t2000,t2001,t2003,t2004,t2005,t2007,t2008,t2011,t2013,t2017,t2018,t2019,t202,t2021,t2024,t2025,t2027,t2029,t203,t2031,t2033,t2036,t2039,t2041,t2043,t2045,t2047,t2048,t205,t2054,t2055,t2056,t2057,t2059,t206,t2060,t2062,t2063,t2064,t2066,t2068,t207,t2070,t2072,t2073,t2075,t2077,t2079,t2080,t2081,t2083,t2089,t2090,t2091,t2093,t2094,t2095,t2096,t2098,t210,t2101,t2102,t2104,t2106,t2107,t2109,t2111,t2112,t2114,t2115,t2117,t2118,t2122,t2123,t2128,t2129,t2130,t2131,t2133,t2134,t2135,t2139,t2141,t2142,t2144,t2145,t2148,t2149,t2150,t2151,t2152,t2153,t2154,t2156,t2158,t2161,t2162,t2164,t2166,t2168,t2175,t2182,t2183,t2184,t2186,t2187,t2189,t2191,t2193,t2194,t2196,t2201,t2202,t2203,t2204,t2208,t2211,t2212,t2214,t222,t2223,t2226,t223,t2231,t2232,t2237,t2245,t2249,t225,t2254,t2258,t2263,t2267,t2269,t227,t2272,t2273,t228,t2307,t231,t2311,t2312,t2315,t2316,t2318,t2319,t2323,t2331,t2332,t2334,t2335,t2337,t2340,t2341,t2344,t2347,t2348,t2356,t236,t2364,t2377,t2379,t2410,t2411,t2419,t2421,t2431,t2439,t2441,t2451,t246,t252,t257,t273,t277,t300,t307,t308,t31,t311,t312,t313,t314,t315,t32,t328,t33,t333,t342,t346,t36,t395,t396,t397,t451,t452,t455,t463,t470,t485,t5,t500,t51,t515,t519,t53,t533,t544,t55,t553,t565,t567,t57,t580,t6,t611,t614,t632,t639,t641,t648,t654,t655,t66,t668,t671,t673,t675,t677,t679,t68,t7,t700,t702,t703,t705,t710,t711,t717,t725,t726,t727,t748,t75,t765,t769,t770,t773,t788,t789,t791,t795,t8,t804,t815,t822,t826,t836,t841,t842,t844,t848,t850,t854,t855,t856,t858,t86,t865,t87,t873,t876,t879,t881,t882,t888,t889,t89,t890,t892,t896,t898,t899,t9,t90,t901,t902,t905,t906,t909,t91,t910,t914,t92,t923,t929,t93,t930,t933,t938,t94,t942,t944,t969,t977,t979,t98,t980,t981,t986,t988,t990,t998});
end
function M = ft_4(ct)
q1 = ct{1};
q2 = ct{2};
t10 = ct{3};
t1006 = ct{4};
t1011 = ct{5};
t1012 = ct{6};
t1018 = ct{7};
t1020 = ct{8};
t1026 = ct{9};
t1029 = ct{10};
t1031 = ct{11};
t1033 = ct{12};
t1034 = ct{13};
t1039 = ct{14};
t1042 = ct{15};
t1046 = ct{16};
t1056 = ct{17};
t1058 = ct{18};
t1060 = ct{19};
t1061 = ct{20};
t1065 = ct{21};
t1066 = ct{22};
t1068 = ct{23};
t1075 = ct{24};
t1079 = ct{25};
t1080 = ct{26};
t1083 = ct{27};
t1090 = ct{28};
t1093 = ct{29};
t1094 = ct{30};
t1095 = ct{31};
t1096 = ct{32};
t1097 = ct{33};
t1098 = ct{34};
t1099 = ct{35};
t1100 = ct{36};
t1102 = ct{37};
t1105 = ct{38};
t1107 = ct{39};
t1108 = ct{40};
t1110 = ct{41};
t1111 = ct{42};
t1112 = ct{43};
t1116 = ct{44};
t1117 = ct{45};
t1119 = ct{46};
t112 = ct{47};
t1120 = ct{48};
t1122 = ct{49};
t1123 = ct{50};
t1124 = ct{51};
t1125 = ct{52};
t1126 = ct{53};
t1127 = ct{54};
t1129 = ct{55};
t113 = ct{56};
t1131 = ct{57};
t1132 = ct{58};
t1136 = ct{59};
t1138 = ct{60};
t114 = ct{61};
t1140 = ct{62};
t1141 = ct{63};
t1143 = ct{64};
t1146 = ct{65};
t1149 = ct{66};
t1151 = ct{67};
t1155 = ct{68};
t1157 = ct{69};
t1159 = ct{70};
t1168 = ct{71};
t1172 = ct{72};
t1174 = ct{73};
t1175 = ct{74};
t1176 = ct{75};
t1177 = ct{76};
t1178 = ct{77};
t1179 = ct{78};
t1181 = ct{79};
t1182 = ct{80};
t1183 = ct{81};
t1186 = ct{82};
t1189 = ct{83};
t119 = ct{84};
t1190 = ct{85};
t1194 = ct{86};
t1196 = ct{87};
t1197 = ct{88};
t1198 = ct{89};
t120 = ct{90};
t1203 = ct{91};
t1204 = ct{92};
t1205 = ct{93};
t1206 = ct{94};
t1207 = ct{95};
t121 = ct{96};
t1213 = ct{97};
t122 = ct{98};
t1222 = ct{99};
t1226 = ct{100};
t1227 = ct{101};
t1228 = ct{102};
t1229 = ct{103};
t1232 = ct{104};
t1241 = ct{105};
t1244 = ct{106};
t1250 = ct{107};
t1255 = ct{108};
t1257 = ct{109};
t1262 = ct{110};
t1264 = ct{111};
t1265 = ct{112};
t1266 = ct{113};
t1267 = ct{114};
t1269 = ct{115};
t1270 = ct{116};
t1272 = ct{117};
t1275 = ct{118};
t1276 = ct{119};
t1277 = ct{120};
t1279 = ct{121};
t1280 = ct{122};
t1282 = ct{123};
t1283 = ct{124};
t1284 = ct{125};
t1287 = ct{126};
t1289 = ct{127};
t129 = ct{128};
t1292 = ct{129};
t1293 = ct{130};
t1295 = ct{131};
t1296 = ct{132};
t1297 = ct{133};
t1298 = ct{134};
t13 = ct{135};
t130 = ct{136};
t1300 = ct{137};
t1301 = ct{138};
t1304 = ct{139};
t1306 = ct{140};
t1307 = ct{141};
t1310 = ct{142};
t1312 = ct{143};
t1313 = ct{144};
t1315 = ct{145};
t1317 = ct{146};
t1318 = ct{147};
t132 = ct{148};
t1323 = ct{149};
t1324 = ct{150};
t1325 = ct{151};
t1326 = ct{152};
t1327 = ct{153};
t1330 = ct{154};
t1332 = ct{155};
t1333 = ct{156};
t1336 = ct{157};
t1337 = ct{158};
t1338 = ct{159};
t1339 = ct{160};
t1340 = ct{161};
t1341 = ct{162};
t1342 = ct{163};
t1343 = ct{164};
t1344 = ct{165};
t1345 = ct{166};
t1346 = ct{167};
t1347 = ct{168};
t1348 = ct{169};
t1351 = ct{170};
t1353 = ct{171};
t1355 = ct{172};
t1356 = ct{173};
t1357 = ct{174};
t1358 = ct{175};
t1359 = ct{176};
t136 = ct{177};
t1360 = ct{178};
t1362 = ct{179};
t1363 = ct{180};
t1364 = ct{181};
t1365 = ct{182};
t1366 = ct{183};
t1367 = ct{184};
t1368 = ct{185};
t1372 = ct{186};
t1375 = ct{187};
t1380 = ct{188};
t1381 = ct{189};
t1383 = ct{190};
t1387 = ct{191};
t1389 = ct{192};
t1391 = ct{193};
t1394 = ct{194};
t1395 = ct{195};
t1396 = ct{196};
t1397 = ct{197};
t1398 = ct{198};
t1399 = ct{199};
t14 = ct{200};
t1402 = ct{201};
t1403 = ct{202};
t1404 = ct{203};
t1406 = ct{204};
t1410 = ct{205};
t1412 = ct{206};
t1413 = ct{207};
t1414 = ct{208};
t1415 = ct{209};
t1416 = ct{210};
t1417 = ct{211};
t1418 = ct{212};
t1419 = ct{213};
t1421 = ct{214};
t1423 = ct{215};
t1424 = ct{216};
t1425 = ct{217};
t1426 = ct{218};
t1427 = ct{219};
t143 = ct{220};
t1431 = ct{221};
t1432 = ct{222};
t1433 = ct{223};
t1435 = ct{224};
t1436 = ct{225};
t1437 = ct{226};
t1441 = ct{227};
t1446 = ct{228};
t1447 = ct{229};
t1451 = ct{230};
t1455 = ct{231};
t1458 = ct{232};
t1461 = ct{233};
t1462 = ct{234};
t1464 = ct{235};
t1465 = ct{236};
t1466 = ct{237};
t1468 = ct{238};
t1469 = ct{239};
t1470 = ct{240};
t1472 = ct{241};
t1473 = ct{242};
t1474 = ct{243};
t1475 = ct{244};
t1478 = ct{245};
t1486 = ct{246};
t1488 = ct{247};
t1489 = ct{248};
t1490 = ct{249};
t1495 = ct{250};
t1496 = ct{251};
t1497 = ct{252};
t1498 = ct{253};
t1499 = ct{254};
t15 = ct{255};
t1500 = ct{256};
t1501 = ct{257};
t1502 = ct{258};
t1503 = ct{259};
t1504 = ct{260};
t1505 = ct{261};
t1507 = ct{262};
t1508 = ct{263};
t1510 = ct{264};
t1512 = ct{265};
t1514 = ct{266};
t1518 = ct{267};
t1519 = ct{268};
t1520 = ct{269};
t1521 = ct{270};
t1522 = ct{271};
t1523 = ct{272};
t1524 = ct{273};
t1526 = ct{274};
t1527 = ct{275};
t1529 = ct{276};
t153 = ct{277};
t1530 = ct{278};
t1532 = ct{279};
t1533 = ct{280};
t1534 = ct{281};
t1535 = ct{282};
t1536 = ct{283};
t1537 = ct{284};
t1538 = ct{285};
t1539 = ct{286};
t1540 = ct{287};
t1542 = ct{288};
t1543 = ct{289};
t1545 = ct{290};
t1546 = ct{291};
t1547 = ct{292};
t1548 = ct{293};
t155 = ct{294};
t1550 = ct{295};
t1551 = ct{296};
t1552 = ct{297};
t1553 = ct{298};
t1555 = ct{299};
t1556 = ct{300};
t1558 = ct{301};
t156 = ct{302};
t1560 = ct{303};
t1561 = ct{304};
t1562 = ct{305};
t1563 = ct{306};
t1564 = ct{307};
t1565 = ct{308};
t1566 = ct{309};
t1567 = ct{310};
t1568 = ct{311};
t1569 = ct{312};
t1570 = ct{313};
t1571 = ct{314};
t1572 = ct{315};
t1574 = ct{316};
t1575 = ct{317};
t1578 = ct{318};
t1581 = ct{319};
t1582 = ct{320};
t1583 = ct{321};
t1584 = ct{322};
t1585 = ct{323};
t1587 = ct{324};
t1588 = ct{325};
t1589 = ct{326};
t1591 = ct{327};
t1592 = ct{328};
t1593 = ct{329};
t1595 = ct{330};
t1596 = ct{331};
t1597 = ct{332};
t1598 = ct{333};
t16 = ct{334};
t1600 = ct{335};
t1601 = ct{336};
t1603 = ct{337};
t1604 = ct{338};
t1605 = ct{339};
t1606 = ct{340};
t1607 = ct{341};
t1608 = ct{342};
t1609 = ct{343};
t1610 = ct{344};
t1612 = ct{345};
t1613 = ct{346};
t1615 = ct{347};
t1616 = ct{348};
t1618 = ct{349};
t1620 = ct{350};
t1621 = ct{351};
t1624 = ct{352};
t1625 = ct{353};
t1627 = ct{354};
t1629 = ct{355};
t1630 = ct{356};
t1632 = ct{357};
t1633 = ct{358};
t1634 = ct{359};
t1636 = ct{360};
t1637 = ct{361};
t1639 = ct{362};
t164 = ct{363};
t1640 = ct{364};
t1641 = ct{365};
t1643 = ct{366};
t1645 = ct{367};
t1648 = ct{368};
t1649 = ct{369};
t165 = ct{370};
t1651 = ct{371};
t1653 = ct{372};
t1654 = ct{373};
t1655 = ct{374};
t1656 = ct{375};
t1657 = ct{376};
t1658 = ct{377};
t1659 = ct{378};
t1660 = ct{379};
t1661 = ct{380};
t1662 = ct{381};
t1663 = ct{382};
t1664 = ct{383};
t1665 = ct{384};
t1668 = ct{385};
t1669 = ct{386};
t167 = ct{387};
t1670 = ct{388};
t1671 = ct{389};
t1672 = ct{390};
t1675 = ct{391};
t1677 = ct{392};
t1678 = ct{393};
t1679 = ct{394};
t1681 = ct{395};
t1682 = ct{396};
t1683 = ct{397};
t1685 = ct{398};
t1686 = ct{399};
t1687 = ct{400};
t1689 = ct{401};
t1690 = ct{402};
t1691 = ct{403};
t1695 = ct{404};
t1696 = ct{405};
t1697 = ct{406};
t1699 = ct{407};
t17 = ct{408};
t170 = ct{409};
t1700 = ct{410};
t1701 = ct{411};
t1702 = ct{412};
t1703 = ct{413};
t1704 = ct{414};
t1705 = ct{415};
t1706 = ct{416};
t1707 = ct{417};
t1715 = ct{418};
t1717 = ct{419};
t172 = ct{420};
t1720 = ct{421};
t1721 = ct{422};
t1725 = ct{423};
t1729 = ct{424};
t173 = ct{425};
t1731 = ct{426};
t1732 = ct{427};
t1734 = ct{428};
t1736 = ct{429};
t1737 = ct{430};
t1739 = ct{431};
t1744 = ct{432};
t1748 = ct{433};
t1749 = ct{434};
t1751 = ct{435};
t1754 = ct{436};
t1755 = ct{437};
t1756 = ct{438};
t1757 = ct{439};
t1758 = ct{440};
t1760 = ct{441};
t1763 = ct{442};
t1764 = ct{443};
t1767 = ct{444};
t1769 = ct{445};
t1771 = ct{446};
t1773 = ct{447};
t1776 = ct{448};
t1777 = ct{449};
t1778 = ct{450};
t1779 = ct{451};
t1782 = ct{452};
t1783 = ct{453};
t1784 = ct{454};
t1785 = ct{455};
t1789 = ct{456};
t1791 = ct{457};
t1794 = ct{458};
t1795 = ct{459};
t1797 = ct{460};
t1798 = ct{461};
t18 = ct{462};
t180 = ct{463};
t1802 = ct{464};
t1803 = ct{465};
t1804 = ct{466};
t1805 = ct{467};
t1806 = ct{468};
t1807 = ct{469};
t1808 = ct{470};
t1809 = ct{471};
t1810 = ct{472};
t1816 = ct{473};
t1817 = ct{474};
t1819 = ct{475};
t1823 = ct{476};
t1824 = ct{477};
t1825 = ct{478};
t1826 = ct{479};
t1827 = ct{480};
t1828 = ct{481};
t1829 = ct{482};
t1867 = ct{483};
t1883 = ct{484};
t1884 = ct{485};
t1885 = ct{486};
t191 = ct{487};
t1919 = ct{488};
t1929 = ct{489};
t1930 = ct{490};
t1935 = ct{491};
t1945 = ct{492};
t1949 = ct{493};
t1952 = ct{494};
t1953 = ct{495};
t1954 = ct{496};
t1960 = ct{497};
t1961 = ct{498};
t1964 = ct{499};
t1965 = ct{500};
t1967 = ct{501};
t1969 = ct{502};
t1970 = ct{503};
t1972 = ct{504};
t1983 = ct{505};
t1985 = ct{506};
t1987 = ct{507};
t1991 = ct{508};
t1992 = ct{509};
t1993 = ct{510};
t1996 = ct{511};
t1997 = ct{512};
t1998 = ct{513};
t1999 = ct{514};
t2000 = ct{515};
t2001 = ct{516};
t2003 = ct{517};
t2004 = ct{518};
t2005 = ct{519};
t2007 = ct{520};
t2008 = ct{521};
t2011 = ct{522};
t2013 = ct{523};
t2017 = ct{524};
t2018 = ct{525};
t2019 = ct{526};
t202 = ct{527};
t2021 = ct{528};
t2024 = ct{529};
t2025 = ct{530};
t2027 = ct{531};
t2029 = ct{532};
t203 = ct{533};
t2031 = ct{534};
t2033 = ct{535};
t2036 = ct{536};
t2039 = ct{537};
t2041 = ct{538};
t2043 = ct{539};
t2045 = ct{540};
t2047 = ct{541};
t2048 = ct{542};
t205 = ct{543};
t2054 = ct{544};
t2055 = ct{545};
t2056 = ct{546};
t2057 = ct{547};
t2059 = ct{548};
t206 = ct{549};
t2060 = ct{550};
t2062 = ct{551};
t2063 = ct{552};
t2064 = ct{553};
t2066 = ct{554};
t2068 = ct{555};
t207 = ct{556};
t2070 = ct{557};
t2072 = ct{558};
t2073 = ct{559};
t2075 = ct{560};
t2077 = ct{561};
t2079 = ct{562};
t2080 = ct{563};
t2081 = ct{564};
t2083 = ct{565};
t2089 = ct{566};
t2090 = ct{567};
t2091 = ct{568};
t2093 = ct{569};
t2094 = ct{570};
t2095 = ct{571};
t2096 = ct{572};
t2098 = ct{573};
t210 = ct{574};
t2101 = ct{575};
t2102 = ct{576};
t2104 = ct{577};
t2106 = ct{578};
t2107 = ct{579};
t2109 = ct{580};
t2111 = ct{581};
t2112 = ct{582};
t2114 = ct{583};
t2115 = ct{584};
t2117 = ct{585};
t2118 = ct{586};
t2122 = ct{587};
t2123 = ct{588};
t2128 = ct{589};
t2129 = ct{590};
t2130 = ct{591};
t2131 = ct{592};
t2133 = ct{593};
t2134 = ct{594};
t2135 = ct{595};
t2139 = ct{596};
t2141 = ct{597};
t2142 = ct{598};
t2144 = ct{599};
t2145 = ct{600};
t2148 = ct{601};
t2149 = ct{602};
t2150 = ct{603};
t2151 = ct{604};
t2152 = ct{605};
t2153 = ct{606};
t2154 = ct{607};
t2156 = ct{608};
t2158 = ct{609};
t2161 = ct{610};
t2162 = ct{611};
t2164 = ct{612};
t2166 = ct{613};
t2168 = ct{614};
t2175 = ct{615};
t2182 = ct{616};
t2183 = ct{617};
t2184 = ct{618};
t2186 = ct{619};
t2187 = ct{620};
t2189 = ct{621};
t2191 = ct{622};
t2193 = ct{623};
t2194 = ct{624};
t2196 = ct{625};
t2201 = ct{626};
t2202 = ct{627};
t2203 = ct{628};
t2204 = ct{629};
t2208 = ct{630};
t2211 = ct{631};
t2212 = ct{632};
t2214 = ct{633};
t222 = ct{634};
t2223 = ct{635};
t2226 = ct{636};
t223 = ct{637};
t2231 = ct{638};
t2232 = ct{639};
t2237 = ct{640};
t2245 = ct{641};
t2249 = ct{642};
t225 = ct{643};
t2254 = ct{644};
t2258 = ct{645};
t2263 = ct{646};
t2267 = ct{647};
t2269 = ct{648};
t227 = ct{649};
t2272 = ct{650};
t2273 = ct{651};
t228 = ct{652};
t2307 = ct{653};
t231 = ct{654};
t2311 = ct{655};
t2312 = ct{656};
t2315 = ct{657};
t2316 = ct{658};
t2318 = ct{659};
t2319 = ct{660};
t2323 = ct{661};
t2331 = ct{662};
t2332 = ct{663};
t2334 = ct{664};
t2335 = ct{665};
t2337 = ct{666};
t2340 = ct{667};
t2341 = ct{668};
t2344 = ct{669};
t2347 = ct{670};
t2348 = ct{671};
t2356 = ct{672};
t236 = ct{673};
t2364 = ct{674};
t2377 = ct{675};
t2379 = ct{676};
t2410 = ct{677};
t2411 = ct{678};
t2419 = ct{679};
t2421 = ct{680};
t2431 = ct{681};
t2439 = ct{682};
t2441 = ct{683};
t2451 = ct{684};
t246 = ct{685};
t252 = ct{686};
t257 = ct{687};
t273 = ct{688};
t277 = ct{689};
t300 = ct{690};
t307 = ct{691};
t308 = ct{692};
t31 = ct{693};
t311 = ct{694};
t312 = ct{695};
t313 = ct{696};
t314 = ct{697};
t315 = ct{698};
t32 = ct{699};
t328 = ct{700};
t33 = ct{701};
t333 = ct{702};
t342 = ct{703};
t346 = ct{704};
t36 = ct{705};
t395 = ct{706};
t396 = ct{707};
t397 = ct{708};
t451 = ct{709};
t452 = ct{710};
t455 = ct{711};
t463 = ct{712};
t470 = ct{713};
t485 = ct{714};
t5 = ct{715};
t500 = ct{716};
t51 = ct{717};
t515 = ct{718};
t519 = ct{719};
t53 = ct{720};
t533 = ct{721};
t544 = ct{722};
t55 = ct{723};
t553 = ct{724};
t565 = ct{725};
t567 = ct{726};
t57 = ct{727};
t580 = ct{728};
t6 = ct{729};
t611 = ct{730};
t614 = ct{731};
t632 = ct{732};
t639 = ct{733};
t641 = ct{734};
t648 = ct{735};
t654 = ct{736};
t655 = ct{737};
t66 = ct{738};
t668 = ct{739};
t671 = ct{740};
t673 = ct{741};
t675 = ct{742};
t677 = ct{743};
t679 = ct{744};
t68 = ct{745};
t7 = ct{746};
t700 = ct{747};
t702 = ct{748};
t703 = ct{749};
t705 = ct{750};
t710 = ct{751};
t711 = ct{752};
t717 = ct{753};
t725 = ct{754};
t726 = ct{755};
t727 = ct{756};
t748 = ct{757};
t75 = ct{758};
t765 = ct{759};
t769 = ct{760};
t770 = ct{761};
t773 = ct{762};
t788 = ct{763};
t789 = ct{764};
t791 = ct{765};
t795 = ct{766};
t8 = ct{767};
t804 = ct{768};
t815 = ct{769};
t822 = ct{770};
t826 = ct{771};
t836 = ct{772};
t841 = ct{773};
t842 = ct{774};
t844 = ct{775};
t848 = ct{776};
t850 = ct{777};
t854 = ct{778};
t855 = ct{779};
t856 = ct{780};
t858 = ct{781};
t86 = ct{782};
t865 = ct{783};
t87 = ct{784};
t873 = ct{785};
t876 = ct{786};
t879 = ct{787};
t881 = ct{788};
t882 = ct{789};
t888 = ct{790};
t889 = ct{791};
t89 = ct{792};
t890 = ct{793};
t892 = ct{794};
t896 = ct{795};
t898 = ct{796};
t899 = ct{797};
t9 = ct{798};
t90 = ct{799};
t901 = ct{800};
t902 = ct{801};
t905 = ct{802};
t906 = ct{803};
t909 = ct{804};
t91 = ct{805};
t910 = ct{806};
t914 = ct{807};
t92 = ct{808};
t923 = ct{809};
t929 = ct{810};
t93 = ct{811};
t930 = ct{812};
t933 = ct{813};
t938 = ct{814};
t94 = ct{815};
t942 = ct{816};
t944 = ct{817};
t969 = ct{818};
t977 = ct{819};
t979 = ct{820};
t98 = ct{821};
t980 = ct{822};
t981 = ct{823};
t986 = ct{824};
t988 = ct{825};
t990 = ct{826};
t998 = ct{827};
t2167 = t1945.*t2001.*3.38795;
t2173 = t1952.*t2000.*3.38795;
t2176 = t1964.*t2001.*3.38795;
t2177 = t1964.*t1999.*3.38795;
t2188 = -t2186;
t2195 = t2007.*(t533.*2.324e-2+t788+t8.*(t57-t165).*3.466000000000001e-2+t15.*(t136-t246).*3.466000000000001e-2).*(-3.5432e-1);
t2197 = -t2196;
t2200 = t2000.*(-t87-t172+t277.*4.9e-4+t711+t727+t770+t13.*(t53-t132).*2.75e-2).*(-3.38795);
t2205 = t2000.*(-t87-t172+t277.*4.9e-4+t711+t727+t770+t13.*(t53-t132).*2.75e-2).*3.38795;
t2213 = t2001.*(t112+t205+t717+t765-t769+t7.*(t51-t155).*2.019e-2+t14.*(t51-t155).*4.9e-4).*(-3.38795);
t2215 = t1987.*t2007.*3.5432e-1;
t2216 = t2001.*(t112+t205+t717+t765-t769+t7.*(t51-t155).*2.019e-2+t14.*(t51-t155).*4.9e-4).*3.38795;
t2217 = t1964.*(-t98+t173+t580-t703-t930+t942-t9.*t10.*(2.1e+1./5.0e+1)+t7.*(t53-t132).*2.019e-2+t14.*(t53-t132).*4.9e-4).*(-3.38795);
t2218 = t1964.*(-t98+t173+t580-t703-t930+t942-t9.*t10.*(2.1e+1./5.0e+1)+t7.*(t53-t132).*2.019e-2+t14.*(t53-t132).*4.9e-4).*3.38795;
t2219 = (t933.*t2162)./2.0;
t2227 = (t854.*t2175)./2.0;
t2229 = t2162.*(t191-t311+t122.*(t51-t155)).*(-1.0./2.0);
t2233 = t1999.*t2001.*3.38795;
t2238 = t1997.*t2007.*3.5432e-1;
t2246 = -t2245;
t2255 = t2003.*t2019.*3.5432e-1;
t2256 = t2175.*(t822+t228.*(t156-t236)).*(-1.0./2.0);
t2257 = t2001.*(-t98+t173+t580-t703-t930+t942-t9.*t10.*(2.1e+1./5.0e+1)+t7.*(t53-t132).*2.019e-2+t14.*(t53-t132).*4.9e-4).*(-3.38795);
t2259 = t2001.*(-t98+t173+t580-t703-t930+t942-t9.*t10.*(2.1e+1./5.0e+1)+t7.*(t53-t132).*2.019e-2+t14.*(t53-t132).*4.9e-4).*3.38795;
t2260 = (t1504.*t2175)./2.0;
t2261 = (t1505.*t2175)./2.0;
t2270 = t2007.*t2036.*3.5432e-1;
t2274 = (t1627.*t2189)./2.0;
t2276 = (t1658.*t2189)./2.0;
t2289 = (t1757.*t2189)./2.0;
t2295 = (t1769.*t2189)./2.0;
t2306 = (t854.*t2267)./2.0;
t2309 = -t2307;
t2313 = -t2312;
t2320 = -t2319;
t2326 = t2027.*t2072.*3.5432e-1;
t2327 = t2027.*(t203-t679+t725.*2.324e-2+t865+t873+t1146+t14.*(t143-t164).*1.9738e-1).*(-3.5432e-1);
t2329 = t2027.*(t203-t679+t725.*2.324e-2+t865+t873+t1146+t14.*(t143-t164).*1.9738e-1).*3.5432e-1;
t2338 = (t1501.*t2254)./2.0;
t2342 = (t1526.*t2254)./2.0;
t2345 = t981+t1029+t1110+t1111+t1262+t1301+t1315+t1469+t1488;
t2350 = (t1504.*t2267)./2.0;
t2353 = (t1505.*t2267)./2.0;
t2357 = (t1603.*t2254)./2.0;
t2366 = t2072.*(t203-t679+t725.*2.324e-2+t865+t873+t1146+t14.*(t143-t164).*1.9738e-1).*(-3.5432e-1);
t2368 = t990+t1122+t1123+t1186+t1204+t1414+t1419+t1441+t1461;
t2369 = t2267.*(t328-t795+t395.*(t53-t132)).*(-1.0./2.0);
t2370 = t1769.*(-t1269+t1284+t1417+t1529+t228.*(t156-t236).*9.999999999999998e-6+t451.*(t156-t236).*1.2e-4).*(-1.0./2.0);
t2371 = (t2267.*(t328-t795+t395.*(t53-t132)))./2.0;
t2375 = t901+t1090+t1206+t1207+t1283+t1338+t1339+t1521+t1523;
t2376 = t1006+t1129+t1196+t1227+t1318+t1323+t1343+t1497+t1503;
t2378 = t1127+t1181+t1257+t1326+t1356+t1357+t1362+t1415+t1418;
t2380 = t1176+t1205+t1270+t1353+t1358+t1380+t1387+t1466+t1470;
t2381 = (t1341.*t2335)./2.0;
t2402 = (t1627.*t2335)./2.0;
t2407 = (t854.*t2379)./2.0;
t2424 = (t1757.*t2335)./2.0;
t2426 = (t1769.*t2335)./2.0;
t2428 = (t1465.*t2377)./2.0;
t2436 = (t1526.*t2377)./2.0;
t2442 = t2379.*(t822+t228.*(t156-t236)).*(-1.0./2.0);
t2443 = (t1603.*t2377)./2.0;
t2447 = (t1505.*t2379)./2.0;
t2456 = t2379.*(t328-t795+t395.*(t53-t132)).*(-1.0./2.0);
t922 = t15.*t898;
t1082 = t307+t677;
t1106 = -t1100;
t1113 = -t1102;
t1271 = -t1266;
t1309 = -t1297;
t1314 = -t1310;
t1361 = t1344.^2;
t1386 = t1368.^2;
t1481 = t898.*4.000000000000028e-5;
t1482 = t898.*3.0e-5;
t1494 = t898.*2.32e-3;
t1549 = -t1542;
t1573 = t888.*t1083;
t1586 = -t14.*t1359.*(t156-t236);
t1590 = -t1583;
t1599 = -t1596;
t1611 = -t1606;
t1614 = t567.*t1359;
t1617 = -t1175.*(t485+t7.*(t53-t132));
t1619 = -t14.*t1383.*(t129+t13.*(t51-t155));
t1622 = -t1621;
t1623 = t614.*t1359;
t1626 = t565.*t1383;
t1635 = t673.*t1359;
t1642 = -t1639;
t1652 = t648.*t1383;
t1666 = t671.*t1383;
t1667 = -t1660;
t1709 = t1399.*4.000000000000028e-5;
t1710 = t1399.*3.0e-5;
t1727 = t836.*t1359;
t1728 = t1399.*2.32e-3;
t1738 = t463+t881+t898;
t1742 = -t8.*t1344.*(t485+t7.*(t53-t132));
t1743 = t888.*t1344;
t1745 = -t1359.*(t485+t7.*(t53-t132));
t1750 = -t1368.*(t485+t7.*(t53-t132));
t1752 = t888.*t1359;
t1759 = t856.*t1383;
t1761 = -t1383.*(t485+t7.*(t53-t132));
t1765 = t8.*t888.*t1368;
t1766 = t888.*t1383;
t1770 = t1031.*t1344;
t1772 = t1508.*4.000000000000028e-5;
t1774 = t1508.*3.0e-5;
t1780 = t1065.*t1344;
t1787 = t1508.*2.32e-3;
t1790 = t1068.*t1368;
t1792 = t1093.*t1344;
t1793 = t1075.*t1368;
t1796 = t1157.*t1344;
t1799 = t1138.*t1368;
t1800 = t1126.*t1368;
t1811 = t1562.*2.2e-4;
t1812 = t1562.*2.900000000000001e-4;
t1814 = t1562.*7.950000000000001e-3;
t1818 = t14.*t1359.*(t156-t236).*(-2.2e-4);
t1820 = t14.*t1359.*(t156-t236).*(-1.089e-2);
t1821 = t14.*t1359.*(t156-t236).*(-2.9e-4);
t1830 = t1332+t1347;
t1831 = t1618.*2.900000000000001e-4;
t1834 = t1613.*2.2e-4;
t1836 = t14.*t1383.*(t129+t13.*(t51-t155)).*(-1.089e-2);
t1837 = t14.*t1383.*(t129+t13.*(t51-t155)).*(-2.9e-4);
t1838 = t1175.*(t485+t7.*(t53-t132)).*(-2.2e-4);
t1839 = t1618.*2.2e-4;
t1840 = t14.*t1383.*(t129+t13.*(t51-t155)).*(-2.2e-4);
t1841 = t1613.*2.900000000000001e-4;
t1842 = t1175.*(t485+t7.*(t53-t132)).*(-2.900000000000001e-4);
t1845 = t1175.*(t485+t7.*(t53-t132)).*2.2e-4;
t1848 = t1175.*(t485+t7.*(t53-t132)).*2.900000000000001e-4;
t1849 = t1613.*7.950000000000001e-3;
t1850 = t1175.*(t485+t7.*(t53-t132)).*(-7.950000000000001e-3);
t1851 = t1618.*7.950000000000001e-3;
t1853 = t1175.*(t485+t7.*(t53-t132)).*7.950000000000001e-3;
t1871 = t1359.*t1368;
t1872 = t1344.*t1383;
t1886 = t668+t1177+t1178;
t1892 = t8.*t1344.*(t485+t7.*(t53-t132)).*(-2.900000000000001e-4);
t1894 = t1359.*(t485+t7.*(t53-t132)).*(-2.900000000000001e-4);
t1895 = t8.*t1344.*(t485+t7.*(t53-t132)).*(-2.9e-4);
t1897 = t1359.*(t485+t7.*(t53-t132)).*(-2.2e-4);
t1900 = t1368.*(t485+t7.*(t53-t132)).*(-2.900000000000001e-4);
t1902 = t1359.*(t485+t7.*(t53-t132)).*(-7.950000000000001e-3);
t1905 = t1368.*(t485+t7.*(t53-t132)).*(-2.2e-4);
t1907 = t8.*t1344.*(t485+t7.*(t53-t132)).*(-2.94e-3);
t1912 = t1368.*(t485+t7.*(t53-t132)).*(-7.950000000000001e-3);
t1915 = t1383.*(t485+t7.*(t53-t132)).*(-1.089e-2);
t1916 = t1383.*(t485+t7.*(t53-t132)).*(-2.9e-4);
t1918 = t1383.*(t485+t7.*(t53-t132)).*(-2.2e-4);
t1966 = t1508+t1514;
t1973 = t841+t1330+t1360;
t1986 = t815+t1421+t1433;
t1989 = t905+t1402+t1451;
t1990 = t1056+t1394+t1399;
t2002 = t222+t553+t611+t632+t641+t876+t882;
t2009 = t986+t1011+t1267+t1277;
t2016 = t1012+t1042+t1280+t1296;
t2020 = t1141+t1543+t1578;
t2034 = t1190+t1585+t1618;
t2082 = t206+t705+t879+t892+t923+t1172+t1174;
t2124 = -t2123;
t2132 = -t2130;
t2137 = t1961.*(t533.*2.324e-2+t788+t8.*(t57-t165).*3.466000000000001e-2+t15.*(t136-t246).*3.466000000000001e-2).*(-3.5432e-1);
t2146 = t1961.*t1987.*3.5432e-1;
t2170 = -t2167;
t2171 = t1961.*t1997.*3.5432e-1;
t2174 = -t2173;
t2178 = -t2177;
t2190 = t1961.*t2007.*3.5432e-1;
t2206 = t1930.*t2033.*3.38795;
t2220 = t1952.*t2033.*3.38795;
t2221 = -t2219;
t2224 = t1961.*t2036.*3.5432e-1;
t2228 = -t2227;
t2234 = -t2233;
t2236 = (t1465.*t2144)./2.0;
t2239 = -t2238;
t2240 = (t1501.*t2144)./2.0;
t2243 = (t1526.*t2144)./2.0;
t2247 = t2033.*(-t87-t172+t277.*4.9e-4+t711+t727+t770+t13.*(t53-t132).*2.75e-2).*(-3.38795);
t2248 = t2033.*(-t87-t172+t277.*4.9e-4+t711+t727+t770+t13.*(t53-t132).*2.75e-2).*3.38795;
t2252 = (t1603.*t2144)./2.0;
t2264 = t2000.*t2033.*3.38795;
t2271 = -t2270;
t2277 = t2003.*t2057.*3.5432e-1;
t2308 = t2019.*t2057.*3.5432e-1;
t2328 = -t2326;
t2339 = -t2338;
t2343 = -t2342;
t2351 = -t2350;
t2355 = -t2353;
t2358 = -t2357;
t2383 = -t2381;
t2394 = (t1465.*t2345)./2.0;
t2396 = (t1501.*t2345)./2.0;
t2400 = (t1526.*t2345)./2.0;
t2403 = -t2402;
t2409 = -t2407;
t2416 = (t1341.*t2376)./2.0;
t2417 = (t854.*t2380)./2.0;
t2425 = -t2424;
t2427 = -t2426;
t2430 = -t2428;
t2433 = (t1465.*t2378)./2.0;
t2435 = (t1501.*t2378)./2.0;
t2440 = (t1627.*t2376)./2.0;
t2444 = (t1658.*t2376)./2.0;
t2445 = t2380.*(t822+t228.*(t156-t236)).*(-1.0./2.0);
t2446 = (t1603.*t2378)./2.0;
t2450 = (t1504.*t2380)./2.0;
t2454 = (t1769.*t2376)./2.0;
t2459 = t2380.*(t328-t795+t395.*(t53-t132)).*(-1.0./2.0);
t2461 = t1098+t1264+t1275+t1413+t1464+t1624+t1634+t1683+t1705;
t2463 = t1143+t1304+t1317+t1431+t1436+t1629+t1645+t1648+t1672;
t2474 = t1367+t1396+t1478+t1540+t1552+t1558+t1592+t1717+t1748;
t2475 = t1381+t1389+t1474+t1539+t1553+t1572+t1574+t1720+t1751;
t2478 = t1355+t1391+t1423+t1587+t1588+t1597+t1608+t1737+t1739;
t2495 = ((t1333+t888.*(t156-t236)).*(t1132+t1293+t1312+t1425-t1629-t1645-t1648+t227.*(t136-t246).*5.0e-5+t7.*t888.*(t129+t13.*(t51-t155)).*3.0e-5))./2.0;
et3 = t1364-t1396+t1475-t1552+t671.*(t129+t13.*(t51-t155)).*5.000000000000004e-4+t655.*(t485+t7.*(t53-t132)).*3.0e-5;
et4 = t888.*(t273+t14.*(t51-t155)).*3.0e-5+t614.*(t156-t236).*5.000000000000004e-4;
et5 = t13.*t836.*(t53-t132).*5.0e-5;
t2496 = t1398.*(et3+et4+et5).*(-1.0./2.0);
et6 = t639+t648.*(t129+t13.*(t51-t155))+t673.*(t156-t236);
et7 = (t1132+t1293+t1312+t1425-t1629-t1645-t1648+t227.*(t136-t246).*5.0e-5+t7.*t888.*(t129+t13.*(t51-t155)).*3.0e-5)./2.0;
t2500 = et6.*et7;
et8 = -t726+t671.*(t129+t13.*(t51-t155))+t614.*(t156-t236);
et9 = (t1132+t1293+t1312+t1425-t1629-t1645-t1648+t227.*(t136-t246).*5.0e-5+t7.*t888.*(t129+t13.*(t51-t155)).*3.0e-5)./2.0;
t2502 = et8.*et9;
et10 = t1107+t565.*(t129+t13.*(t51-t155))+t452.*(t57-t165);
et11 = (t1132+t1293+t1312+t1425-t1629-t1645-t1648+t227.*(t136-t246).*5.0e-5+t7.*t888.*(t129+t13.*(t51-t155)).*3.0e-5)./2.0;
t2503 = et10.*et11;
et12 = -t826+t856.*(t129+t13.*(t51-t155))+t836.*(t156-t236);
et13 = (t1132+t1293+t1312+t1425-t1629-t1645-t1648+t227.*(t136-t246).*5.0e-5+t7.*t888.*(t129+t13.*(t51-t155)).*3.0e-5)./2.0;
t2511 = et12.*et13;
et14 = t1364-t1396+t1475-t1552+t671.*(t129+t13.*(t51-t155)).*5.000000000000004e-4+t655.*(t485+t7.*(t53-t132)).*3.0e-5;
et15 = t888.*(t273+t14.*(t51-t155)).*3.0e-5+t614.*(t156-t236).*5.000000000000004e-4;
et16 = t13.*t836.*(t53-t132).*5.0e-5;
t2526 = ((t1333+t888.*(t156-t236)).*(et14+et15+et16))./2.0;
et17 = t748.*2.81e-3+t1342-t1432+t1606+t1621-t1736+t648.*(t129+t13.*(t51-t155)).*5.0e-5;
et18 = t888.*(t153+t7.*(t143-t164)).*4.000000000000028e-5+t673.*(t156-t236).*5.0e-5;
t2529 = t1826.*(et17+et18).*(-1.0./2.0);
et19 = t748.*2.81e-3+t1342-t1432+t1606+t1621-t1736+t648.*(t129+t13.*(t51-t155)).*5.0e-5;
et20 = t888.*(t153+t7.*(t143-t164)).*4.000000000000028e-5+t673.*(t156-t236).*5.0e-5;
t2530 = (t1826.*(et19+et20))./2.0;
et21 = t1364-t1396+t1475-t1552+t671.*(t129+t13.*(t51-t155)).*5.000000000000004e-4+t655.*(t485+t7.*(t53-t132)).*3.0e-5;
et22 = t888.*(t273+t14.*(t51-t155)).*3.0e-5+t614.*(t156-t236).*5.000000000000004e-4;
et23 = t13.*t836.*(t53-t132).*5.0e-5;
t2536 = ((t639+t648.*(t129+t13.*(t51-t155))+t673.*(t156-t236)).*(et21+et22+et23))./2.0;
et24 = t1364-t1396+t1475-t1552+t671.*(t129+t13.*(t51-t155)).*5.000000000000004e-4+t655.*(t485+t7.*(t53-t132)).*3.0e-5;
et25 = t888.*(t273+t14.*(t51-t155)).*3.0e-5+t614.*(t156-t236).*5.000000000000004e-4;
et26 = t13.*t836.*(t53-t132).*5.0e-5;
t2542 = ((t1107+t565.*(t129+t13.*(t51-t155))+t452.*(t57-t165)).*(et24+et25+et26))./2.0;
et27 = t748.*2.81e-3+t1342-t1432+t1606+t1621-t1736+t648.*(t129+t13.*(t51-t155)).*5.0e-5;
et28 = t888.*(t153+t7.*(t143-t164)).*4.000000000000028e-5+t673.*(t156-t236).*5.0e-5;
t2546 = t1884.*(et27+et28).*(-1.0./2.0);
et29 = t748.*2.81e-3+t1342-t1432+t1606+t1621-t1736+t648.*(t129+t13.*(t51-t155)).*5.0e-5;
et30 = t888.*(t153+t7.*(t143-t164)).*4.000000000000028e-5+t673.*(t156-t236).*5.0e-5;
t2559 = ((et29+et30).*(t1189+t225.*(t136-t246)+t856.*(t66-t210)))./2.0;
et31 = t1364-t1396+t1475-t1552+t671.*(t129+t13.*(t51-t155)).*5.000000000000004e-4+t655.*(t485+t7.*(t53-t132)).*3.0e-5;
et32 = t888.*(t273+t14.*(t51-t155)).*3.0e-5+t614.*(t156-t236).*5.000000000000004e-4;
et33 = t13.*t836.*(t53-t132).*5.0e-5;
t2570 = ((et31+et32+et33).*(-t826+t856.*(t129+t13.*(t51-t155))+t836.*(t156-t236)))./2.0;
et34 = t748.*2.81e-3+t1342-t1432+t1606+t1621-t1736+t648.*(t129+t13.*(t51-t155)).*5.0e-5;
et35 = t888.*(t153+t7.*(t143-t164)).*4.000000000000028e-5+t673.*(t156-t236).*5.0e-5;
t2574 = t1967.*(et34+et35).*(-1.0./2.0);
et36 = t748.*2.81e-3+t1342-t1432+t1606+t1621-t1736+t648.*(t129+t13.*(t51-t155)).*5.0e-5;
et37 = t888.*(t153+t7.*(t143-t164)).*4.000000000000028e-5+t673.*(t156-t236).*5.0e-5;
t2575 = (t1967.*(et36+et37))./2.0;
t1506 = t922.*2.900000000000001e-4;
t1511 = t922.*2.2e-4;
t1513 = t922.*7.950000000000001e-3;
t1631 = -t1626;
t1708 = t1361.*2.9e-4;
t1711 = t1361.*2.900000000000001e-4;
t1713 = -t1709;
t1719 = t1361.*2.94e-3;
t1726 = t1386.*2.900000000000001e-4;
t1730 = t1386.*2.9e-4;
t1741 = t1386.*2.94e-3;
t1753 = -t1743;
t1762 = -t1752;
t1768 = t519+t906+t922;
t1786 = -t1780;
t1813 = t1573.*2.2e-4;
t1815 = t1573.*2.900000000000001e-4;
t1822 = t1573.*7.950000000000001e-3;
t1832 = t1614.*1.089e-2;
t1833 = t1614.*2.9e-4;
t1835 = t1614.*2.2e-4;
t1843 = -t1831;
t1844 = -t1834;
t1846 = -t1839;
t1847 = -t1841;
t1852 = -t1849;
t1854 = -t1851;
t1855 = t1623.*1.089e-2;
t1856 = t1623.*2.9e-4;
t1857 = t1623.*2.2e-4;
t1858 = t1626.*2.2e-4;
t1862 = t1626.*1.089e-2;
t1863 = t1626.*2.9e-4;
t1868 = t1635.*1.089e-2;
t1869 = t1635.*2.9e-4;
t1870 = t1635.*2.2e-4;
t1873 = t1652.*1.089e-2;
t1874 = t1652.*2.9e-4;
t1875 = t1652.*2.2e-4;
t1876 = -t1872;
t1877 = t1666.*1.089e-2;
t1878 = t1666.*2.9e-4;
t1879 = t1666.*2.2e-4;
t1888 = t1727.*1.089e-2;
t1889 = t1727.*2.9e-4;
t1890 = t1727.*2.2e-4;
t1893 = t1743.*2.900000000000001e-4;
t1896 = t1743.*2.2e-4;
t1901 = t1743.*7.950000000000001e-3;
t1903 = t1752.*1.089e-2;
t1904 = t1752.*2.9e-4;
t1906 = t1752.*2.2e-4;
t1913 = t1759.*1.089e-2;
t1914 = t1759.*2.9e-4;
t1917 = t1759.*2.2e-4;
t1920 = t1765.*2.9e-4;
t1921 = t1766.*2.2e-4;
t1922 = t1765.*2.900000000000001e-4;
t1923 = t1766.*2.900000000000001e-4;
t1924 = t1766.*7.950000000000001e-3;
t1925 = t1765.*2.94e-3;
t1926 = t1770.*2.9e-4;
t1927 = t1770.*2.900000000000001e-4;
t1931 = t1770.*2.94e-3;
t1932 = t1780.*2.900000000000001e-4;
t1933 = t1780.*2.9e-4;
t1937 = t1780.*2.94e-3;
t1939 = t1790.*2.9e-4;
t1940 = t1792.*2.900000000000001e-4;
t1941 = t1790.*2.900000000000001e-4;
t1942 = t1792.*2.9e-4;
t1943 = t1793.*2.900000000000001e-4;
t1944 = t1793.*2.9e-4;
t1946 = t1792.*2.94e-3;
t1947 = t1790.*2.94e-3;
t1948 = t1793.*2.94e-3;
t1950 = t1796.*2.900000000000001e-4;
t1951 = t1796.*2.9e-4;
t1955 = t1800.*2.900000000000001e-4;
t1956 = t1799.*2.9e-4;
t1957 = t1800.*2.9e-4;
t1958 = t1796.*2.94e-3;
t1959 = t1799.*2.900000000000001e-4;
t1962 = t1799.*2.94e-3;
t1963 = t1800.*2.94e-3;
t1974 = t1871.*2.900000000000001e-4;
t1975 = t1872.*2.900000000000001e-4;
t1976 = t1871.*2.9e-4;
t1977 = t1872.*2.9e-4;
t1980 = t1871.*2.94e-3;
t1981 = t1872.*2.94e-3;
t1984 = t899+t1361+t1386;
t2006 = t791+t1046+t1313+t1314;
t2032 = t1108+t1613+t1617;
t2035 = t1306+t1562+t1573;
t2038 = t1228+t1586+t1619;
t2049 = t1226+t1635+t1652;
t2051 = t1298+t1623+t1666;
t2065 = t90+t94+t114+t702+t844+t850+t858+t1099+t1113;
t2067 = t86+t92+t113+t700+t842+t848+t855+t1096+t1106;
t2084 = t1363+t1727+t1759;
t2085 = t1336+t1745+t1766;
t2088 = t1346+t1742+t1765;
t2113 = t1412+t1770+t1793;
t2120 = t1424+t1792+t1800;
t2121 = t1395+t1796+t1799;
t2126 = t91+t98+t202+t804+t988+t998+t1018+t1271+t1279;
t2136 = t89+t93+t207+t789+t1026+t1058+t1061+t1289+t1309;
t2169 = t1930.*t2002.*3.38795;
t2172 = -t2171;
t2179 = t1952.*t2002.*3.38795;
t2209 = t2002.*(-t87-t172+t277.*4.9e-4+t711+t727+t770+t13.*(t53-t132).*2.75e-2).*(-3.38795);
t2210 = t2002.*(-t87-t172+t277.*4.9e-4+t711+t727+t770+t13.*(t53-t132).*2.75e-2).*3.38795;
t2222 = -t2220;
t2225 = -t2224;
t2235 = t2000.*t2002.*3.38795;
t2241 = -t2240;
t2242 = t2003.*t2009.*3.5432e-1;
t2244 = -t2243;
t2253 = -t2252;
t2262 = t2009.*t2019.*3.5432e-1;
t2266 = t2002.*t2033.*3.38795;
t2268 = t2016.*t2027.*3.5432e-1;
t2278 = -t2277;
t2280 = t1241+t1447+t1472+t1481+t1640+t1663;
t2284 = t2009.*t2057.*3.5432e-1;
t2287 = t1244+t1468+t1473+t1482+t1655+t1679;
t2288 = t1265+t1437+t1489+t1494+t1630+t1654;
t2296 = t2003.*t2082.*3.5432e-1;
t2300 = t2016.*t2072.*3.5432e-1;
t2301 = t2009.*t2082.*3.5432e-1;
t2303 = t2016.*(t203-t679+t725.*2.324e-2+t865+t873+t1146+t14.*(t143-t164).*1.9738e-1).*(-3.5432e-1);
t2305 = t2016.*(t203-t679+t725.*2.324e-2+t865+t873+t1146+t14.*(t143-t164).*1.9738e-1).*3.5432e-1;
t2310 = -t2308;
t2324 = t2019.*t2082.*3.5432e-1;
t2363 = t2057.*t2082.*3.5432e-1;
t2397 = -t2396;
t2401 = -t2400;
t2406 = t1636+t1641+t1649+t1656+t1787+t1791;
t2412 = t1661+t1664+t1668+t1670+t1772+t1778;
t2413 = t1651+t1657+t1675+t1681+t1774+t1779;
t2418 = -t2417;
t2434 = -t2433;
t2462 = t1112+t1276+t1295+t1435+t1455+t1642+t1643+t1667+t1677;
t2465 = t1884.*(t1662+t1665-t1772+t1773+t856.*(t156-t236).*2.81e-3+t888.*(t156-t236).*5.0e-5).*(-1.0./2.0);
t2466 = (t1884.*(t1662+t1665-t1772+t1773+t856.*(t156-t236).*2.81e-3+t888.*(t156-t236).*5.0e-5))./2.0;
t2470 = t1345+t1375+t1490+t1533+t1538+t1549+t1571+t1732+t1764;
t2471 = ((t1189+t225.*(t136-t246)+t856.*(t66-t210)).*(t1662+t1665-t1772+t1773+t856.*(t156-t236).*2.81e-3+t888.*(t156-t236).*5.0e-5))./2.0;
t2472 = t1929.*(t1662+t1665-t1772+t1773+t856.*(t156-t236).*2.81e-3+t888.*(t156-t236).*5.0e-5).*(-1.0./2.0);
t2476 = t1325+t1372+t1462+t1563+t1564+t1590+t1599+t1755+t1756;
t2477 = t1351+t1397+t1432+t1566+t1567+t1611+t1622+t1734+t1736;
t2479 = t1406+t1427+t1524+t1527+t1532+t1570+t1582+t1721+t1728;
t2480 = t1967.*(t1662+t1665-t1772+t1773+t856.*(t156-t236).*2.81e-3+t888.*(t156-t236).*5.0e-5).*(-1.0./2.0);
t2481 = t1416+t1458+t1520+t1545+t1547+t1581+t1591+t1706+t1710;
t2492 = (t1738.*t2461)./2.0;
t2497 = (t1398.*t2478)./2.0;
t2501 = -t2500;
t2504 = -t2502;
t2505 = -t2503;
et38 = t1537+t1575+t1704-t1710+t396.*(t167+t7.*(t55-t130)).*3.0e-5+t565.*(t129+t13.*(t51-t155)).*5.000000000000004e-4;
et39 = t225.*(t136-t246).*5.0e-5+t452.*(t57-t165).*5.000000000000004e-4;
et40 = t856.*(t66-t210).*5.0e-5;
t2506 = t1398.*(et38+et39+et40).*(-1.0./2.0);
t2510 = (t1966.*t2461)./2.0;
et41 = t710.*4.000000000000028e-5-t1375+t1486+t1535+t1542+t671.*(t129+t13.*(t51-t155)).*3.0e-5;
et42 = t655.*(t485+t7.*(t53-t132)).*2.32e-3+t888.*(t273+t14.*(t51-t155)).*2.32e-3;
et43 = t614.*(t156-t236).*3.0e-5;
t2512 = t1738.*(et41+et42+et43).*(-1.0./2.0);
t2515 = (t1986.*t2461)./2.0;
t2522 = t2461.*(t890+t655.*(t485+t7.*(t53-t132))+t888.*(t273+t14.*(t51-t155))).*(-1.0./2.0);
t2523 = (t1990.*t2461)./2.0;
t2524 = (t1826.*t2475)./2.0;
t2527 = -t2526;
t2531 = t2478.*(t1333+t888.*(t156-t236)).*(-1.0./2.0);
et44 = t1394.*4.000000000000028e-5+t1518+t1530+t1593+t1709+t565.*(t129+t13.*(t51-t155)).*5.0e-5;
et45 = t225.*(t136-t246).*2.81e-3+t452.*(t57-t165).*5.0e-5;
et46 = t856.*(t66-t210).*2.81e-3;
t2535 = t1826.*(et44+et45+et46).*(-1.0./2.0);
et47 = t1394.*4.000000000000028e-5+t1518+t1530+t1593+t1709+t565.*(t129+t13.*(t51-t155)).*5.0e-5;
et48 = t225.*(t136-t246).*2.81e-3+t452.*(t57-t165).*5.0e-5;
et49 = t856.*(t66-t210).*2.81e-3;
t2537 = (t1826.*(et47+et48+et49))./2.0;
et50 = t1537+t1575+t1704-t1710+t396.*(t167+t7.*(t55-t130)).*3.0e-5+t565.*(t129+t13.*(t51-t155)).*5.000000000000004e-4;
et51 = t225.*(t136-t246).*5.0e-5+t452.*(t57-t165).*5.000000000000004e-4;
et52 = t856.*(t66-t210).*5.0e-5;
t2538 = ((t1333+t888.*(t156-t236)).*(et50+et51+et52))./2.0;
t2547 = t2478.*(-t726+t671.*(t129+t13.*(t51-t155))+t614.*(t156-t236)).*(-1.0./2.0);
t2548 = t2478.*(t1107+t565.*(t129+t13.*(t51-t155))+t452.*(t57-t165)).*(-1.0./2.0);
t2549 = (t2478.*(-t726+t671.*(t129+t13.*(t51-t155))+t614.*(t156-t236)))./2.0;
t2550 = (t2478.*(t1107+t565.*(t129+t13.*(t51-t155))+t452.*(t57-t165)))./2.0;
t2551 = t2475.*(t1189+t225.*(t136-t246)+t856.*(t66-t210)).*(-1.0./2.0);
t2552 = (t1929.*t2475)./2.0;
et53 = t1394.*4.000000000000028e-5+t1518+t1530+t1593+t1709+t565.*(t129+t13.*(t51-t155)).*5.0e-5;
et54 = t225.*(t136-t246).*2.81e-3+t452.*(t57-t165).*5.0e-5;
et55 = t856.*(t66-t210).*2.81e-3;
t2554 = t1884.*(et53+et54+et55).*(-1.0./2.0);
et56 = t1537+t1575+t1704-t1710+t396.*(t167+t7.*(t55-t130)).*3.0e-5+t565.*(t129+t13.*(t51-t155)).*5.000000000000004e-4;
et57 = t225.*(t136-t246).*5.0e-5+t452.*(t57-t165).*5.000000000000004e-4;
et58 = t856.*(t66-t210).*5.0e-5;
t2555 = ((t639+t648.*(t129+t13.*(t51-t155))+t673.*(t156-t236)).*(et56+et57+et58))./2.0;
et59 = t1537+t1575+t1704-t1710+t396.*(t167+t7.*(t55-t130)).*3.0e-5+t565.*(t129+t13.*(t51-t155)).*5.000000000000004e-4;
et60 = t225.*(t136-t246).*5.0e-5+t452.*(t57-t165).*5.000000000000004e-4;
et61 = t856.*(t66-t210).*5.0e-5;
t2558 = ((et59+et60+et61).*(-t726+t671.*(t129+t13.*(t51-t155))+t614.*(t156-t236)))./2.0;
et62 = t710.*4.000000000000028e-5-t1375+t1486+t1535+t1542+t671.*(t129+t13.*(t51-t155)).*3.0e-5;
et63 = t655.*(t485+t7.*(t53-t132)).*2.32e-3+t888.*(t273+t14.*(t51-t155)).*2.32e-3;
et64 = t614.*(t156-t236).*3.0e-5;
t2563 = t1966.*(et62+et63+et64).*(-1.0./2.0);
et65 = t1394.*4.000000000000028e-5+t1518+t1530+t1593+t1709+t565.*(t129+t13.*(t51-t155)).*5.0e-5;
et66 = t225.*(t136-t246).*2.81e-3+t452.*(t57-t165).*5.0e-5;
et67 = t856.*(t66-t210).*2.81e-3;
t2564 = t1929.*(et65+et66+et67).*(-1.0./2.0);
et68 = t1394.*4.000000000000028e-5+t1518+t1530+t1593+t1709+t565.*(t129+t13.*(t51-t155)).*5.0e-5;
et69 = t225.*(t136-t246).*2.81e-3+t452.*(t57-t165).*5.0e-5;
et70 = t856.*(t66-t210).*2.81e-3;
t2565 = (t1929.*(et68+et69+et70))./2.0;
t2566 = (t1967.*t2475)./2.0;
t2571 = -t2570;
et71 = t710.*4.000000000000028e-5-t1375+t1486+t1535+t1542+t671.*(t129+t13.*(t51-t155)).*3.0e-5;
et72 = t655.*(t485+t7.*(t53-t132)).*2.32e-3+t888.*(t273+t14.*(t51-t155)).*2.32e-3;
et73 = t614.*(t156-t236).*3.0e-5;
t2572 = t1973.*(et71+et72+et73).*(-1.0./2.0);
et74 = t710.*4.000000000000028e-5-t1375+t1486+t1535+t1542+t671.*(t129+t13.*(t51-t155)).*3.0e-5;
et75 = t655.*(t485+t7.*(t53-t132)).*2.32e-3+t888.*(t273+t14.*(t51-t155)).*2.32e-3;
et76 = t614.*(t156-t236).*3.0e-5;
t2573 = (t1973.*(et74+et75+et76))./2.0;
